simulink model "untitled"  (R2016a)
settings: Solver=VariableStepAuto  StartTime=0.0  StopTime=10.0  RelTol=1e-3
libraries: neural x419
(part 4 of 5)

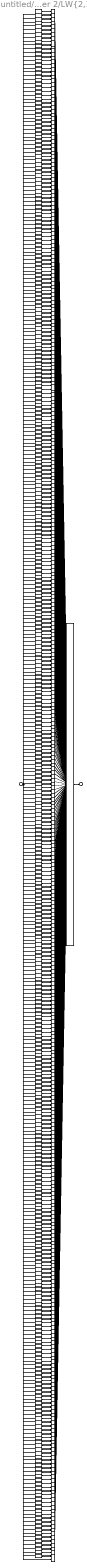
== system untitled/Function Fitting Neural Network/Layer 2/LW{2,1} ==
  "ad{2,1}" : Inport  PortDimensions=10
      mask Display: e = 0.06;c1 = [120 230 180]/255;c2 = ([120 230 180]+0)/(256+128);c3 = ([120 230 180]+128)/(256+128);patch([0 1 1 0],[0 0 1 1],c1);patch([0 1 1 1-e 1-e 0+e],[0 0 1 1-e 0+e 0+e],c2);patch([0 0 1 1-e 0+e 0+e],[0 1 1 1-e 1-e 0+e],c3);plot([0 1 1 0 0],[0 0 1 1 0]);
  "IW{2,1}(1,:)'" : Constant  Value=[0.35457568526871353;-0.37262881568746131;-0.093772998130510987;0.299001882254391;0.71652059707009119;-0.40821366360697064;-1.1727395577661341;-0.24105879281632298;-0.15545806944447227;-0.96766624006371971]
      mask Display: e = 0.06;c1 = [120 150 230]/255;c2 = ([120 150 230]+0)/383;c3 = ([120 150 230]+128)/383;patch([0 1 1 0],[0 0 1 1],c1);patch([0 1 1 1-e 1-e 0+e],[0 0 1 1-e 0+e 0+e],c2);patch([0 0 1 1-e 0+e 0+e],[0 1 1 1-e 1-e 0+e],c3);plot([0 1 1 0 0],[0 0 1 1 0]);disp('weights');
  "IW{2,1}(10,:)'" : Constant  Value=[-0.51241962484819403;0.18696428722763422;0.096689156544264743;-0.91173964698263843;1.2071503274550923;-0.1015978129931896;-1.2900331369557421;-0.89853148309609598;0.72911399796122411;0.2154652253377683]
      mask Display: e = 0.06;c1 = [120 150 230]/255;c2 = ([120 150 230]+0)/383;c3 = ([120 150 230]+128)/383;patch([0 1 1 0],[0 0 1 1],c1);patch([0 1 1 1-e 1-e 0+e],[0 0 1 1-e 0+e 0+e],c2);patch([0 0 1 1-e 0+e 0+e],[0 1 1 1-e 1-e 0+e],c3);plot([0 1 1 0 0],[0 0 1 1 0]);disp('weights');
  "IW{2,1}(100,:)'" : Constant  Value=[-0.59467351366079291;-0.46314267056547948;0.30643708606798353;0.024053983344356877;0.66007872910628429;0.75245943586493769;0.56148392880052234;0.88532483151243879;-0.50114763812176322;0.62203932838690612]
      mask Display: e = 0.06;c1 = [120 150 230]/255;c2 = ([120 150 230]+0)/383;c3 = ([120 150 230]+128)/383;patch([0 1 1 0],[0 0 1 1],c1);patch([0 1 1 1-e 1-e 0+e],[0 0 1 1-e 0+e 0+e],c2);patch([0 0 1 1-e 0+e 0+e],[0 1 1 1-e 1-e 0+e],c3);plot([0 1 1 0 0],[0 0 1 1 0]);disp('weights');
  "IW{2,1}(101,:)'" : Constant  Value=[0.132183354502735;-0.41451653539518085;0.016380979248929839;-0.74444212048968017;-0.35095430295178254;-0.45812487947094915;-0.3864796214085417;-0.1758270264418865;0.44561967553264237;-1.2062139208858689]
      mask Display: e = 0.06;c1 = [120 150 230]/255;c2 = ([120 150 230]+0)/383;c3 = ([120 150 230]+128)/383;patch([0 1 1 0],[0 0 1 1],c1);patch([0 1 1 1-e 1-e 0+e],[0 0 1 1-e 0+e 0+e],c2);patch([0 0 1 1-e 0+e 0+e],[0 1 1 1-e 1-e 0+e],c3);plot([0 1 1 0 0],[0 0 1 1 0]);disp('weights');
  "IW{2,1}(102,:)'" : Constant  Value=[0.91550733628729186;-0.17596632668060738;-0.23501466731066578;-0.43131413009170461;1.0039394563268771;-0.061370045893368474;-0.10056229228428686;0.35460263945948478;0.079910893784825646;-0.89223794061441064]
      mask Display: e = 0.06;c1 = [120 150 230]/255;c2 = ([120 150 230]+0)/383;c3 = ([120 150 230]+128)/383;patch([0 1 1 0],[0 0 1 1],c1);patch([0 1 1 1-e 1-e 0+e],[0 0 1 1-e 0+e 0+e],c2);patch([0 0 1 1-e 0+e 0+e],[0 1 1 1-e 1-e 0+e],c3);plot([0 1 1 0 0],[0 0 1 1 0]);disp('weights');
  "IW{2,1}(103,:)'" : Constant  Value=[0.012259853410431329;-0.31444307148354467;0.35552415069161591;-0.82679374849055298;-0.45038411512840826;-0.39748281945567426;-0.85214363441640906;0.44358232172792822;0.29629420030451536;0.6064841209214985]
      mask Display: e = 0.06;c1 = [120 150 230]/255;c2 = ([120 150 230]+0)/383;c3 = ([120 150 230]+128)/383;patch([0 1 1 0],[0 0 1 1],c1);patch([0 1 1 1-e 1-e 0+e],[0 0 1 1-e 0+e 0+e],c2);patch([0 0 1 1-e 0+e 0+e],[0 1 1 1-e 1-e 0+e],c3);plot([0 1 1 0 0],[0 0 1 1 0]);disp('weights');
  "IW{2,1}(104,:)'" : Constant  Value=[-0.52691192650108576;-0.19464969257009473;-0.16386531967861129;-0.31658642759094502;0.64379806911152437;0.5492776953247257;0.0085904991406464959;-0.27791306732414345;0.45618230462846576;-0.41271807660853826]
      mask Display: e = 0.06;c1 = [120 150 230]/255;c2 = ([120 150 230]+0)/383;c3 = ([120 150 230]+128)/383;patch([0 1 1 0],[0 0 1 1],c1);patch([0 1 1 1-e 1-e 0+e],[0 0 1 1-e 0+e 0+e],c2);patch([0 0 1 1-e 0+e 0+e],[0 1 1 1-e 1-e 0+e],c3);plot([0 1 1 0 0],[0 0 1 1 0]);disp('weights');
  "IW{2,1}(105,:)'" : Constant  Value=[0.0036104131310510656;-0.5108457587075188;-0.42012674601703315;-0.67458325990890222;-1.0099146022211332;0.49569765597714416;0.82567298712166171;0.10590138830719459;0.58403979278397478;0.34540661755692653]
      mask Display: e = 0.06;c1 = [120 150 230]/255;c2 = ([120 150 230]+0)/383;c3 = ([120 150 230]+128)/383;patch([0 1 1 0],[0 0 1 1],c1);patch([0 1 1 1-e 1-e 0+e],[0 0 1 1-e 0+e 0+e],c2);patch([0 0 1 1-e 0+e 0+e],[0 1 1 1-e 1-e 0+e],c3);plot([0 1 1 0 0],[0 0 1 1 0]);disp('weights');
  "IW{2,1}(106,:)'" : Constant  Value=[0.6298401480397835;-0.35713898884332712;1.0969036725783468;0.22290348339327648;0.63928028679609472;0.19280713089077245;0.57375743745156227;0.35484963283244514;0.54621996310164911;-0.42525917136785357]
      mask Display: e = 0.06;c1 = [120 150 230]/255;c2 = ([120 150 230]+0)/383;c3 = ([120 150 230]+128)/383;patch([0 1 1 0],[0 0 1 1],c1);patch([0 1 1 1-e 1-e 0+e],[0 0 1 1-e 0+e 0+e],c2);patch([0 0 1 1-e 0+e 0+e],[0 1 1 1-e 1-e 0+e],c3);plot([0 1 1 0 0],[0 0 1 1 0]);disp('weights');
  "IW{2,1}(107,:)'" : Constant  Value=[-0.54121767469762583;-0.15709203256179666;0.56849802045345743;-0.63744679364538026;-0.83237528600719402;0.30709467382596495;-0.54279673919964622;0.054529333255173174;0.20487910196507619;0.93234667245376635]
      mask Display: e = 0.06;c1 = [120 150 230]/255;c2 = ([120 150 230]+0)/383;c3 = ([120 150 230]+128)/383;patch([0 1 1 0],[0 0 1 1],c1);patch([0 1 1 1-e 1-e 0+e],[0 0 1 1-e 0+e 0+e],c2);patch([0 0 1 1-e 0+e 0+e],[0 1 1 1-e 1-e 0+e],c3);plot([0 1 1 0 0],[0 0 1 1 0]);disp('weights');
  "IW{2,1}(108,:)'" : Constant  Value=[0.87117914257995643;-0.8350687060946369;-0.52769471700262027;0.095004289510615431;1.1883750573422214;-0.049426168392697201;0.77796622090666123;0.47514241846633865;0.70746717159394057;0.46821260443696688]
      mask Display: e = 0.06;c1 = [120 150 230]/255;c2 = ([120 150 230]+0)/383;c3 = ([120 150 230]+128)/383;patch([0 1 1 0],[0 0 1 1],c1);patch([0 1 1 1-e 1-e 0+e],[0 0 1 1-e 0+e 0+e],c2);patch([0 0 1 1-e 0+e 0+e],[0 1 1 1-e 1-e 0+e],c3);plot([0 1 1 0 0],[0 0 1 1 0]);disp('weights');
  "IW{2,1}(109,:)'" : Constant  Value=[-0.093098287400667917;-0.42566624607377573;0.13802357294765616;0.12600752979896604;-0.39805809535751313;0.051077209656586242;-0.010384967949629564;-0.098925686133072455;0.95828758938569147;0.63472242371386045]
      mask Display: e = 0.06;c1 = [120 150 230]/255;c2 = ([120 150 230]+0)/383;c3 = ([120 150 230]+128)/383;patch([0 1 1 0],[0 0 1 1],c1);patch([0 1 1 1-e 1-e 0+e],[0 0 1 1-e 0+e 0+e],c2);patch([0 0 1 1-e 0+e 0+e],[0 1 1 1-e 1-e 0+e],c3);plot([0 1 1 0 0],[0 0 1 1 0]);disp('weights');
  "IW{2,1}(11,:)'" : Constant  Value=[0.87385905042111978;-0.59302251482942259;-0.57235715014876254;0.68353185522794968;1.0174079732112598;0.27032333860384478;-0.055552601487100089;-0.60055456873861501;0.69962443470780555;-0.87073796700187378]
      mask Display: e = 0.06;c1 = [120 150 230]/255;c2 = ([120 150 230]+0)/383;c3 = ([120 150 230]+128)/383;patch([0 1 1 0],[0 0 1 1],c1);patch([0 1 1 1-e 1-e 0+e],[0 0 1 1-e 0+e 0+e],c2);patch([0 0 1 1-e 0+e 0+e],[0 1 1 1-e 1-e 0+e],c3);plot([0 1 1 0 0],[0 0 1 1 0]);disp('weights');
  "IW{2,1}(110,:)'" : Constant  Value=[-0.45402764551089492;-0.4424626913130032;0.70634245673847851;0.12095992557048846;-0.76716468124193804;0.64679971773739886;0.73068307254207221;-0.1155523840382818;0.75520677335095443;-5.4313536676370289e-06]
      mask Display: e = 0.06;c1 = [120 150 230]/255;c2 = ([120 150 230]+0)/383;c3 = ([120 150 230]+128)/383;patch([0 1 1 0],[0 0 1 1],c1);patch([0 1 1 1-e 1-e 0+e],[0 0 1 1-e 0+e 0+e],c2);patch([0 0 1 1-e 0+e 0+e],[0 1 1 1-e 1-e 0+e],c3);plot([0 1 1 0 0],[0 0 1 1 0]);disp('weights');
  "IW{2,1}(111,:)'" : Constant  Value=[0.35856321400782343;-0.12534766693171134;0.07962987090539092;-0.60785703622425813;-0.38430086232607419;0.30093885714405233;-0.29137973701213238;0.24631778243741809;-0.5626882874146204;-0.6833696969081674]
      mask Display: e = 0.06;c1 = [120 150 230]/255;c2 = ([120 150 230]+0)/383;c3 = ([120 150 230]+128)/383;patch([0 1 1 0],[0 0 1 1],c1);patch([0 1 1 1-e 1-e 0+e],[0 0 1 1-e 0+e 0+e],c2);patch([0 0 1 1-e 0+e 0+e],[0 1 1 1-e 1-e 0+e],c3);plot([0 1 1 0 0],[0 0 1 1 0]);disp('weights');
  "IW{2,1}(112,:)'" : Constant  Value=[-0.51368243852562334;-0.48320720571860942;0.15046834876398124;-0.15687559453180761;0.4695672881405818;0.40398577095198729;-0.8294845938603097;0.45460692171736328;-0.65214613716902159;0.5645422206690478]
      mask Display: e = 0.06;c1 = [120 150 230]/255;c2 = ([120 150 230]+0)/383;c3 = ([120 150 230]+128)/383;patch([0 1 1 0],[0 0 1 1],c1);patch([0 1 1 1-e 1-e 0+e],[0 0 1 1-e 0+e 0+e],c2);patch([0 0 1 1-e 0+e 0+e],[0 1 1 1-e 1-e 0+e],c3);plot([0 1 1 0 0],[0 0 1 1 0]);disp('weights');
  "IW{2,1}(113,:)'" : Constant  Value=[0.2249827070654358;-0.5547870151241886;0.44125214045465366;0.10185870942545092;-0.72373304904497293;0.36734856354623896;-0.3943082956206293;-0.013381755084662945;-0.61597198634890338;0.073567333518367112]
      mask Display: e = 0.06;c1 = [120 150 230]/255;c2 = ([120 150 230]+0)/383;c3 = ([120 150 230]+128)/383;patch([0 1 1 0],[0 0 1 1],c1);patch([0 1 1 1-e 1-e 0+e],[0 0 1 1-e 0+e 0+e],c2);patch([0 0 1 1-e 0+e 0+e],[0 1 1 1-e 1-e 0+e],c3);plot([0 1 1 0 0],[0 0 1 1 0]);disp('weights');
  "IW{2,1}(114,:)'" : Constant  Value=[0.44715657086469585;-0.72184644042513646;-0.10679542344572371;0.33394805863425275;1.3097117535626552;0.13752345875085706;0.0041012097003376366;0.52921934544137084;0.47705001987924522;0.60162273497358432]
      mask Display: e = 0.06;c1 = [120 150 230]/255;c2 = ([120 150 230]+0)/383;c3 = ([120 150 230]+128)/383;patch([0 1 1 0],[0 0 1 1],c1);patch([0 1 1 1-e 1-e 0+e],[0 0 1 1-e 0+e 0+e],c2);patch([0 0 1 1-e 0+e 0+e],[0 1 1 1-e 1-e 0+e],c3);plot([0 1 1 0 0],[0 0 1 1 0]);disp('weights');
  "IW{2,1}(115,:)'" : Constant  Value=[0.072990874063348754;0.3863994496468931;-0.99669381823398551;-0.82947335628810992;-0.926316182620321;0.12138423091903472;-0.42001636335877995;-0.52417760541218628;0.11809912221407559;0.74754410579861164]
      mask Display: e = 0.06;c1 = [120 150 230]/255;c2 = ([120 150 230]+0)/383;c3 = ([120 150 230]+128)/383;patch([0 1 1 0],[0 0 1 1],c1);patch([0 1 1 1-e 1-e 0+e],[0 0 1 1-e 0+e 0+e],c2);patch([0 0 1 1-e 0+e 0+e],[0 1 1 1-e 1-e 0+e],c3);plot([0 1 1 0 0],[0 0 1 1 0]);disp('weights');
  "IW{2,1}(116,:)'" : Constant  Value=[-0.2288055411522181;0.14131988055967634;0.52041469449043676;-0.99856714860427098;0.17410368995406242;-0.052745805695831871;-0.99979512395444892;-0.35899147958971089;0.020783894468624331;-0.074273715439050342]
      mask Display: e = 0.06;c1 = [120 150 230]/255;c2 = ([120 150 230]+0)/383;c3 = ([120 150 230]+128)/383;patch([0 1 1 0],[0 0 1 1],c1);patch([0 1 1 1-e 1-e 0+e],[0 0 1 1-e 0+e 0+e],c2);patch([0 0 1 1-e 0+e 0+e],[0 1 1 1-e 1-e 0+e],c3);plot([0 1 1 0 0],[0 0 1 1 0]);disp('weights');
  "IW{2,1}(117,:)'" : Constant  Value=[-0.82340701668346539;-0.51434424071955409;0.91471776355589407;-0.33288238922418745;0.25648880682466646;0.70822982577740778;-0.6932001556180224;0.31607280530056825;-0.93009913518226872;0.068609139618715453]
      mask Display: e = 0.06;c1 = [120 150 230]/255;c2 = ([120 150 230]+0)/383;c3 = ([120 150 230]+128)/383;patch([0 1 1 0],[0 0 1 1],c1);patch([0 1 1 1-e 1-e 0+e],[0 0 1 1-e 0+e 0+e],c2);patch([0 0 1 1-e 0+e 0+e],[0 1 1 1-e 1-e 0+e],c3);plot([0 1 1 0 0],[0 0 1 1 0]);disp('weights');
  "IW{2,1}(118,:)'" : Constant  Value=[-0.49649736447447651;0.45372633367474352;-0.34080312653242439;-0.66503308065530253;-0.1437992940186234;0.40249309287773155;-0.99295207713203126;-0.33562443638377937;-0.56546214554735619;0.49432810354427731]
      mask Display: e = 0.06;c1 = [120 150 230]/255;c2 = ([120 150 230]+0)/383;c3 = ([120 150 230]+128)/383;patch([0 1 1 0],[0 0 1 1],c1);patch([0 1 1 1-e 1-e 0+e],[0 0 1 1-e 0+e 0+e],c2);patch([0 0 1 1-e 0+e 0+e],[0 1 1 1-e 1-e 0+e],c3);plot([0 1 1 0 0],[0 0 1 1 0]);disp('weights');
  "IW{2,1}(119,:)'" : Constant  Value=[-0.10669085982625769;-0.21956149733535044;0.58793916789199496;-0.40100123749963718;-0.91327196109126496;0.53224945141593838;0.47283979571705442;-0.4790545028876399;1.1407185294966518;0.0053917100134790452]
      mask Display: e = 0.06;c1 = [120 150 230]/255;c2 = ([120 150 230]+0)/383;c3 = ([120 150 230]+128)/383;patch([0 1 1 0],[0 0 1 1],c1);patch([0 1 1 1-e 1-e 0+e],[0 0 1 1-e 0+e 0+e],c2);patch([0 0 1 1-e 0+e 0+e],[0 1 1 1-e 1-e 0+e],c3);plot([0 1 1 0 0],[0 0 1 1 0]);disp('weights');
  "IW{2,1}(12,:)'" : Constant  Value=[0.48160846672355573;0.19812719218488389;-0.44365884094007213;-0.1118865542679382;0.27293932443032587;-0.22992509263083483;-1.2232905553509303;-0.49844923236274263;0.45638164301901762;0.12236853164908057]
      mask Display: e = 0.06;c1 = [120 150 230]/255;c2 = ([120 150 230]+0)/383;c3 = ([120 150 230]+128)/383;patch([0 1 1 0],[0 0 1 1],c1);patch([0 1 1 1-e 1-e 0+e],[0 0 1 1-e 0+e 0+e],c2);patch([0 0 1 1-e 0+e 0+e],[0 1 1 1-e 1-e 0+e],c3);plot([0 1 1 0 0],[0 0 1 1 0]);disp('weights');
  "IW{2,1}(120,:)'" : Constant  Value=[-0.10634859977705739;-0.052631616825708348;1.4195649331520863;-0.00084437965909707957;0.42285466275429279;0.70700655299443582;0.34595288214413045;0.14152229005737385;-0.062790561497810926;-0.50122881361225213]
      mask Display: e = 0.06;c1 = [120 150 230]/255;c2 = ([120 150 230]+0)/383;c3 = ([120 150 230]+128)/383;patch([0 1 1 0],[0 0 1 1],c1);patch([0 1 1 1-e 1-e 0+e],[0 0 1 1-e 0+e 0+e],c2);patch([0 0 1 1-e 0+e 0+e],[0 1 1 1-e 1-e 0+e],c3);plot([0 1 1 0 0],[0 0 1 1 0]);disp('weights');
  "IW{2,1}(121,:)'" : Constant  Value=[0.75241460306983421;-0.12382045592416158;-0.18934015310768379;0.15978093552599948;-0.40957040115013393;0.55440558737447043;0.31139781430429297;0.35891166148113807;0.84576008771658606;-0.92215142010749429]
      mask Display: e = 0.06;c1 = [120 150 230]/255;c2 = ([120 150 230]+0)/383;c3 = ([120 150 230]+128)/383;patch([0 1 1 0],[0 0 1 1],c1);patch([0 1 1 1-e 1-e 0+e],[0 0 1 1-e 0+e 0+e],c2);patch([0 0 1 1-e 0+e 0+e],[0 1 1 1-e 1-e 0+e],c3);plot([0 1 1 0 0],[0 0 1 1 0]);disp('weights');
  "IW{2,1}(122,:)'" : Constant  Value=[0.014533892077952471;-1.0864692283910478;-0.24978734334647062;-0.20714287190409467;0.41688992619603121;0.020843004186868241;-0.30036513169667467;0.6447122172862042;-0.44816953174537666;-0.6254452491744753]
      mask Display: e = 0.06;c1 = [120 150 230]/255;c2 = ([120 150 230]+0)/383;c3 = ([120 150 230]+128)/383;patch([0 1 1 0],[0 0 1 1],c1);patch([0 1 1 1-e 1-e 0+e],[0 0 1 1-e 0+e 0+e],c2);patch([0 0 1 1-e 0+e 0+e],[0 1 1 1-e 1-e 0+e],c3);plot([0 1 1 0 0],[0 0 1 1 0]);disp('weights');
  "IW{2,1}(123,:)'" : Constant  Value=[-0.55358584751208206;-0.92521608564350843;0.67501683373877341;-0.070487248336855296;0.020102317195281716;-0.31375904864237314;-1.0252812554265067;-0.29798368298503497;-0.22574251461160327;-0.057919377180048304]
      mask Display: e = 0.06;c1 = [120 150 230]/255;c2 = ([120 150 230]+0)/383;c3 = ([120 150 230]+128)/383;patch([0 1 1 0],[0 0 1 1],c1);patch([0 1 1 1-e 1-e 0+e],[0 0 1 1-e 0+e 0+e],c2);patch([0 0 1 1-e 0+e 0+e],[0 1 1 1-e 1-e 0+e],c3);plot([0 1 1 0 0],[0 0 1 1 0]);disp('weights');
  "IW{2,1}(124,:)'" : Constant  Value=[-0.094164787441411352;-0.90477229098315259;-0.14308614220465629;0.68442827404295736;0.95717575287916334;-0.18018870819129618;-1.0367015099687653;-0.228224166373137;0.44195239019836341;0.29375654463105255]
      mask Display: e = 0.06;c1 = [120 150 230]/255;c2 = ([120 150 230]+0)/383;c3 = ([120 150 230]+128)/383;patch([0 1 1 0],[0 0 1 1],c1);patch([0 1 1 1-e 1-e 0+e],[0 0 1 1-e 0+e 0+e],c2);patch([0 0 1 1-e 0+e 0+e],[0 1 1 1-e 1-e 0+e],c3);plot([0 1 1 0 0],[0 0 1 1 0]);disp('weights');
  "IW{2,1}(125,:)'" : Constant  Value=[0.25918346779046053;-0.66229732874088987;-0.14821536867020529;0.37319280184569709;0.77589616900903002;0.66975340214018286;0.86153956282309252;0.34949141088372687;-0.71824829000813462;0.8783877605606627]
      mask Display: e = 0.06;c1 = [120 150 230]/255;c2 = ([120 150 230]+0)/383;c3 = ([120 150 230]+128)/383;patch([0 1 1 0],[0 0 1 1],c1);patch([0 1 1 1-e 1-e 0+e],[0 0 1 1-e 0+e 0+e],c2);patch([0 0 1 1-e 0+e 0+e],[0 1 1 1-e 1-e 0+e],c3);plot([0 1 1 0 0],[0 0 1 1 0]);disp('weights');
  "IW{2,1}(126,:)'" : Constant  Value=[-0.085774924571177247;-1.2775593839237314;-1.0753491198620599;-0.1245259294998598;0.88107812747589931;-0.42695412098538321;-0.58480038198142781;0.82133593724887144;-0.75444202274592564;0.17411838762112253]
      mask Display: e = 0.06;c1 = [120 150 230]/255;c2 = ([120 150 230]+0)/383;c3 = ([120 150 230]+128)/383;patch([0 1 1 0],[0 0 1 1],c1);patch([0 1 1 1-e 1-e 0+e],[0 0 1 1-e 0+e 0+e],c2);patch([0 0 1 1-e 0+e 0+e],[0 1 1 1-e 1-e 0+e],c3);plot([0 1 1 0 0],[0 0 1 1 0]);disp('weights');
  "IW{2,1}(127,:)'" : Constant  Value=[0.19769923896271896;-0.89301981169820355;-0.11564107353940761;-0.25978116749604885;0.56145028987742485;0.42377493028536328;1.2224631895737739;0.57960114490207171;0.37954472845902248;0.11026282514903726]
      mask Display: e = 0.06;c1 = [120 150 230]/255;c2 = ([120 150 230]+0)/383;c3 = ([120 150 230]+128)/383;patch([0 1 1 0],[0 0 1 1],c1);patch([0 1 1 1-e 1-e 0+e],[0 0 1 1-e 0+e 0+e],c2);patch([0 0 1 1-e 0+e 0+e],[0 1 1 1-e 1-e 0+e],c3);plot([0 1 1 0 0],[0 0 1 1 0]);disp('weights');
  "IW{2,1}(128,:)'" : Constant  Value=[0.52884557596552373;-0.25984156317850038;-0.12794366690907111;0.01803659075444497;-0.27347206670087748;0.342733749696636;-0.51354095947049949;0.16186322264992775;-1.0862616684542652;1.4767430332722691]
      mask Display: e = 0.06;c1 = [120 150 230]/255;c2 = ([120 150 230]+0)/383;c3 = ([120 150 230]+128)/383;patch([0 1 1 0],[0 0 1 1],c1);patch([0 1 1 1-e 1-e 0+e],[0 0 1 1-e 0+e 0+e],c2);patch([0 0 1 1-e 0+e 0+e],[0 1 1 1-e 1-e 0+e],c3);plot([0 1 1 0 0],[0 0 1 1 0]);disp('weights');
  "IW{2,1}(129,:)'" : Constant  Value=[0.75786961871891667;-0.074835868624982871;0.79040911501239242;1.0007053012623659;0.37791249894770557;0.85316218872741612;0.40970699716135928;0.88783479708554969;-0.87875083537845844;0.59899649409211353]
      mask Display: e = 0.06;c1 = [120 150 230]/255;c2 = ([120 150 230]+0)/383;c3 = ([120 150 230]+128)/383;patch([0 1 1 0],[0 0 1 1],c1);patch([0 1 1 1-e 1-e 0+e],[0 0 1 1-e 0+e 0+e],c2);patch([0 0 1 1-e 0+e 0+e],[0 1 1 1-e 1-e 0+e],c3);plot([0 1 1 0 0],[0 0 1 1 0]);disp('weights');
  "IW{2,1}(13,:)'" : Constant  Value=[0.68737360350036181;0.14343559982558957;0.35348444111783106;0.60648354004990934;0.91124708494743012;0.04306279224824705;-0.18153377551600688;0.68901300485973116;-0.50222409270449153;0.13877128185435972]
      mask Display: e = 0.06;c1 = [120 150 230]/255;c2 = ([120 150 230]+0)/383;c3 = ([120 150 230]+128)/383;patch([0 1 1 0],[0 0 1 1],c1);patch([0 1 1 1-e 1-e 0+e],[0 0 1 1-e 0+e 0+e],c2);patch([0 0 1 1-e 0+e 0+e],[0 1 1 1-e 1-e 0+e],c3);plot([0 1 1 0 0],[0 0 1 1 0]);disp('weights');
  "IW{2,1}(130,:)'" : Constant  Value=[0.54323359350819234;-0.25298207203940526;0.39779238695437691;0.28493583185010518;-0.72980298213089956;0.0007700830524480784;-0.45352416582028754;0.077090561776502087;-0.19742973340063341;-0.29070953650683073]
      mask Display: e = 0.06;c1 = [120 150 230]/255;c2 = ([120 150 230]+0)/383;c3 = ([120 150 230]+128)/383;patch([0 1 1 0],[0 0 1 1],c1);patch([0 1 1 1-e 1-e 0+e],[0 0 1 1-e 0+e 0+e],c2);patch([0 0 1 1-e 0+e 0+e],[0 1 1 1-e 1-e 0+e],c3);plot([0 1 1 0 0],[0 0 1 1 0]);disp('weights');
  "IW{2,1}(131,:)'" : Constant  Value=[0.97878280264957052;-0.49403704756137012;-0.36677975235608196;0.097786011441210408;-0.018498962251421613;-0.36530395873255661;0.2334949438478936;-0.22826989708304976;0.15268980758730025;0.14933168696978888]
      mask Display: e = 0.06;c1 = [120 150 230]/255;c2 = ([120 150 230]+0)/383;c3 = ([120 150 230]+128)/383;patch([0 1 1 0],[0 0 1 1],c1);patch([0 1 1 1-e 1-e 0+e],[0 0 1 1-e 0+e 0+e],c2);patch([0 0 1 1-e 0+e 0+e],[0 1 1 1-e 1-e 0+e],c3);plot([0 1 1 0 0],[0 0 1 1 0]);disp('weights');
  "IW{2,1}(132,:)'" : Constant  Value=[0.60411093516280645;0.81353606944854429;0.003599919896469711;-0.9407960401058918;0.13795065004212817;0.41634349891179523;0.61553232960671089;0.18584762270653454;0.75915028452746958;-0.72757720678792848]
      mask Display: e = 0.06;c1 = [120 150 230]/255;c2 = ([120 150 230]+0)/383;c3 = ([120 150 230]+128)/383;patch([0 1 1 0],[0 0 1 1],c1);patch([0 1 1 1-e 1-e 0+e],[0 0 1 1-e 0+e 0+e],c2);patch([0 0 1 1-e 0+e 0+e],[0 1 1 1-e 1-e 0+e],c3);plot([0 1 1 0 0],[0 0 1 1 0]);disp('weights');
  "IW{2,1}(133,:)'" : Constant  Value=[0.89636858614286585;-0.43930648748674328;0.36348095586936136;0.42202233354664997;0.080242274820562204;-0.17527706896099893;-0.27678234817463548;0.18205392307498788;0.26248544652801364;-0.60731321474183864]
      mask Display: e = 0.06;c1 = [120 150 230]/255;c2 = ([120 150 230]+0)/383;c3 = ([120 150 230]+128)/383;patch([0 1 1 0],[0 0 1 1],c1);patch([0 1 1 1-e 1-e 0+e],[0 0 1 1-e 0+e 0+e],c2);patch([0 0 1 1-e 0+e 0+e],[0 1 1 1-e 1-e 0+e],c3);plot([0 1 1 0 0],[0 0 1 1 0]);disp('weights');
  "IW{2,1}(134,:)'" : Constant  Value=[0.46766779301282968;-0.66166835902964338;-0.053471630666557482;0.20941091529739264;-0.27431112396490887;-0.038380363421930963;0.57150995549276795;-0.11805819126615381;0.4542250235667678;0.55470191658962753]
      mask Display: e = 0.06;c1 = [120 150 230]/255;c2 = ([120 150 230]+0)/383;c3 = ([120 150 230]+128)/383;patch([0 1 1 0],[0 0 1 1],c1);patch([0 1 1 1-e 1-e 0+e],[0 0 1 1-e 0+e 0+e],c2);patch([0 0 1 1-e 0+e 0+e],[0 1 1 1-e 1-e 0+e],c3);plot([0 1 1 0 0],[0 0 1 1 0]);disp('weights');
  "IW{2,1}(135,:)'" : Constant  Value=[0.43487119300343791;-0.12294690238958098;-0.087736019523446507;0.26167006899088735;-0.5885537372425822;0.57930981669587878;-0.33638400569811111;0.3704508366766428;-0.3399032648473701;-0.28242557070351021]
      mask Display: e = 0.06;c1 = [120 150 230]/255;c2 = ([120 150 230]+0)/383;c3 = ([120 150 230]+128)/383;patch([0 1 1 0],[0 0 1 1],c1);patch([0 1 1 1-e 1-e 0+e],[0 0 1 1-e 0+e 0+e],c2);patch([0 0 1 1-e 0+e 0+e],[0 1 1 1-e 1-e 0+e],c3);plot([0 1 1 0 0],[0 0 1 1 0]);disp('weights');
  "IW{2,1}(136,:)'" : Constant  Value=[0.87531369177677609;-0.088562053715001116;-0.50157240895004473;-0.47102435346078919;0.69915570499538215;-0.27921213245334076;-0.87326892756430141;0.36052387179430673;-0.96143693001145092;-0.17549088416610464]
      mask Display: e = 0.06;c1 = [120 150 230]/255;c2 = ([120 150 230]+0)/383;c3 = ([120 150 230]+128)/383;patch([0 1 1 0],[0 0 1 1],c1);patch([0 1 1 1-e 1-e 0+e],[0 0 1 1-e 0+e 0+e],c2);patch([0 0 1 1-e 0+e 0+e],[0 1 1 1-e 1-e 0+e],c3);plot([0 1 1 0 0],[0 0 1 1 0]);disp('weights');
  "IW{2,1}(137,:)'" : Constant  Value=[0.04084567294535886;-0.45479850199360849;-0.15935677807927359;-0.16347981152794955;0.83695772071454166;0.69898633357112272;0.92626956822206041;0.31086917495667193;-0.18959112727733612;0.7499543456261748]
      mask Display: e = 0.06;c1 = [120 150 230]/255;c2 = ([120 150 230]+0)/383;c3 = ([120 150 230]+128)/383;patch([0 1 1 0],[0 0 1 1],c1);patch([0 1 1 1-e 1-e 0+e],[0 0 1 1-e 0+e 0+e],c2);patch([0 0 1 1-e 0+e 0+e],[0 1 1 1-e 1-e 0+e],c3);plot([0 1 1 0 0],[0 0 1 1 0]);disp('weights');
  "IW{2,1}(138,:)'" : Constant  Value=[0.57219232295499267;0.020263776079628176;-0.079704395170736755;-0.74272920860931724;0.82984320022030256;0.24958130088689573;0.77599202689430868;0.31725933454895744;0.42162457988928725;-0.24703646084574413]
      mask Display: e = 0.06;c1 = [120 150 230]/255;c2 = ([120 150 230]+0)/383;c3 = ([120 150 230]+128)/383;patch([0 1 1 0],[0 0 1 1],c1);patch([0 1 1 1-e 1-e 0+e],[0 0 1 1-e 0+e 0+e],c2);patch([0 0 1 1-e 0+e 0+e],[0 1 1 1-e 1-e 0+e],c3);plot([0 1 1 0 0],[0 0 1 1 0]);disp('weights');
  "IW{2,1}(139,:)'" : Constant  Value=[-0.64791329129744479;-0.68039534992550543;0.46068321870552537;-0.44670816247921685;-0.85457524198659396;0.052372287861784883;-0.28315196682942978;0.050960586513293604;-0.34113385269778135;-0.12619683269990617]
      mask Display: e = 0.06;c1 = [120 150 230]/255;c2 = ([120 150 230]+0)/383;c3 = ([120 150 230]+128)/383;patch([0 1 1 0],[0 0 1 1],c1);patch([0 1 1 1-e 1-e 0+e],[0 0 1 1-e 0+e 0+e],c2);patch([0 0 1 1-e 0+e 0+e],[0 1 1 1-e 1-e 0+e],c3);plot([0 1 1 0 0],[0 0 1 1 0]);disp('weights');
  "IW{2,1}(14,:)'" : Constant  Value=[0.60307547539237827;0.26160630807644503;-0.31915455123711362;0.35648864783644302;0.10935038552164415;0.57115159516591585;0.13337076223726663;-0.33810699894513374;-0.0076439180204547971;-0.34620005775426466]
      mask Display: e = 0.06;c1 = [120 150 230]/255;c2 = ([120 150 230]+0)/383;c3 = ([120 150 230]+128)/383;patch([0 1 1 0],[0 0 1 1],c1);patch([0 1 1 1-e 1-e 0+e],[0 0 1 1-e 0+e 0+e],c2);patch([0 0 1 1-e 0+e 0+e],[0 1 1 1-e 1-e 0+e],c3);plot([0 1 1 0 0],[0 0 1 1 0]);disp('weights');
  "IW{2,1}(140,:)'" : Constant  Value=[-0.0030291752852869558;-0.67980394133413324;-0.17885139181676857;-0.76669362139205643;0.22816259255475249;-0.47415457060627852;-1.1503135723297553;-0.61111712626978165;-0.12145632927079997;-0.85689992494030265]
      mask Display: e = 0.06;c1 = [120 150 230]/255;c2 = ([120 150 230]+0)/383;c3 = ([120 150 230]+128)/383;patch([0 1 1 0],[0 0 1 1],c1);patch([0 1 1 1-e 1-e 0+e],[0 0 1 1-e 0+e 0+e],c2);patch([0 0 1 1-e 0+e 0+e],[0 1 1 1-e 1-e 0+e],c3);plot([0 1 1 0 0],[0 0 1 1 0]);disp('weights');
  "IW{2,1}(141,:)'" : Constant  Value=[1.1528381514813444;-0.19886352123262094;-0.32237521779107103;0.53280504643341076;0.54235638409397091;-0.20431979798160893;0.41859342160632868;-0.27049055688648832;0.72348698962931113;0.22721198189363229]
      mask Display: e = 0.06;c1 = [120 150 230]/255;c2 = ([120 150 230]+0)/383;c3 = ([120 150 230]+128)/383;patch([0 1 1 0],[0 0 1 1],c1);patch([0 1 1 1-e 1-e 0+e],[0 0 1 1-e 0+e 0+e],c2);patch([0 0 1 1-e 0+e 0+e],[0 1 1 1-e 1-e 0+e],c3);plot([0 1 1 0 0],[0 0 1 1 0]);disp('weights');
  "IW{2,1}(142,:)'" : Constant  Value=[1.0348774094391338;0.39994075004194773;-0.10449199246842319;0.58555814890475077;-0.43854398931414074;0.62129764197704607;0.57989198576789014;0.61806327947082651;-0.80509314522689135;0.22740352648194026]
      mask Display: e = 0.06;c1 = [120 150 230]/255;c2 = ([120 150 230]+0)/383;c3 = ([120 150 230]+128)/383;patch([0 1 1 0],[0 0 1 1],c1);patch([0 1 1 1-e 1-e 0+e],[0 0 1 1-e 0+e 0+e],c2);patch([0 0 1 1-e 0+e 0+e],[0 1 1 1-e 1-e 0+e],c3);plot([0 1 1 0 0],[0 0 1 1 0]);disp('weights');
  "IW{2,1}(143,:)'" : Constant  Value=[0.47591930778768854;0.11029936675550972;-0.11704275436264812;-1.1282355903680503;0.035452001204951289;-0.35020455737237144;-0.41406855655358321;-0.057474545214064456;-0.24301739685938317;-0.75257830822867067]
      mask Display: e = 0.06;c1 = [120 150 230]/255;c2 = ([120 150 230]+0)/383;c3 = ([120 150 230]+128)/383;patch([0 1 1 0],[0 0 1 1],c1);patch([0 1 1 1-e 1-e 0+e],[0 0 1 1-e 0+e 0+e],c2);patch([0 0 1 1-e 0+e 0+e],[0 1 1 1-e 1-e 0+e],c3);plot([0 1 1 0 0],[0 0 1 1 0]);disp('weights');
  "IW{2,1}(144,:)'" : Constant  Value=[0.013610878879226157;-0.5936025788659649;0.17473336943233647;0.11562238591574327;0.65243191169465042;0.69623129247364601;0.033335398108974762;0.26830968898347057;-0.18982946576075041;-0.3178018271525288]
      mask Display: e = 0.06;c1 = [120 150 230]/255;c2 = ([120 150 230]+0)/383;c3 = ([120 150 230]+128)/383;patch([0 1 1 0],[0 0 1 1],c1);patch([0 1 1 1-e 1-e 0+e],[0 0 1 1-e 0+e 0+e],c2);patch([0 0 1 1-e 0+e 0+e],[0 1 1 1-e 1-e 0+e],c3);plot([0 1 1 0 0],[0 0 1 1 0]);disp('weights');
  "IW{2,1}(145,:)'" : Constant  Value=[0.79353310108425479;-0.98041238760606764;0.43142067668329331;0.94935906057659536;-0.25235217004692806;-0.11597467566125697;-0.79824077009467964;0.58212520912044108;-0.62611583634461465;-0.26615231117298133]
      mask Display: e = 0.06;c1 = [120 150 230]/255;c2 = ([120 150 230]+0)/383;c3 = ([120 150 230]+128)/383;patch([0 1 1 0],[0 0 1 1],c1);patch([0 1 1 1-e 1-e 0+e],[0 0 1 1-e 0+e 0+e],c2);patch([0 0 1 1-e 0+e 0+e],[0 1 1 1-e 1-e 0+e],c3);plot([0 1 1 0 0],[0 0 1 1 0]);disp('weights');
  "IW{2,1}(146,:)'" : Constant  Value=[-0.14663084735383669;-0.7152012856519111;0.79022637736240497;-0.39265024231146162;0.11015162851622627;0.1439881491271458;-0.21722187234832716;0.35490782758032535;-0.28781516352467973;-0.83905117783707472]
      mask Display: e = 0.06;c1 = [120 150 230]/255;c2 = ([120 150 230]+0)/383;c3 = ([120 150 230]+128)/383;patch([0 1 1 0],[0 0 1 1],c1);patch([0 1 1 1-e 1-e 0+e],[0 0 1 1-e 0+e 0+e],c2);patch([0 0 1 1-e 0+e 0+e],[0 1 1 1-e 1-e 0+e],c3);plot([0 1 1 0 0],[0 0 1 1 0]);disp('weights');
  "IW{2,1}(147,:)'" : Constant  Value=[0.51456095092215304;0.013308895325224501;0.23973578416266431;-0.39893358253935407;0.86217847435459549;0.23731709690746533;0.32107943016162388;0.4579415028239332;-0.12170571728965782;-0.72497605428726442]
      mask Display: e = 0.06;c1 = [120 150 230]/255;c2 = ([120 150 230]+0)/383;c3 = ([120 150 230]+128)/383;patch([0 1 1 0],[0 0 1 1],c1);patch([0 1 1 1-e 1-e 0+e],[0 0 1 1-e 0+e 0+e],c2);patch([0 0 1 1-e 0+e 0+e],[0 1 1 1-e 1-e 0+e],c3);plot([0 1 1 0 0],[0 0 1 1 0]);disp('weights');
  "IW{2,1}(148,:)'" : Constant  Value=[-0.28370341159362489;0.14189555301935247;0.22615733950226197;-1.4289170794829864;0.19275807464534023;-0.29588546279050809;-0.60250261553372697;-0.55024367335468194;0.28602429652844596;-1.2087566889439874]
      mask Display: e = 0.06;c1 = [120 150 230]/255;c2 = ([120 150 230]+0)/383;c3 = ([120 150 230]+128)/383;patch([0 1 1 0],[0 0 1 1],c1);patch([0 1 1 1-e 1-e 0+e],[0 0 1 1-e 0+e 0+e],c2);patch([0 0 1 1-e 0+e 0+e],[0 1 1 1-e 1-e 0+e],c3);plot([0 1 1 0 0],[0 0 1 1 0]);disp('weights');
  "IW{2,1}(149,:)'" : Constant  Value=[0.29220286997692346;-0.42868361288169421;0.091667071657286048;0.0023825430328358599;0.68759817291230851;0.48731248515528514;0.073982555723268464;-0.47896314396146461;0.2481890200979214;-0.78006686064629083]
      mask Display: e = 0.06;c1 = [120 150 230]/255;c2 = ([120 150 230]+0)/383;c3 = ([120 150 230]+128)/383;patch([0 1 1 0],[0 0 1 1],c1);patch([0 1 1 1-e 1-e 0+e],[0 0 1 1-e 0+e 0+e],c2);patch([0 0 1 1-e 0+e 0+e],[0 1 1 1-e 1-e 0+e],c3);plot([0 1 1 0 0],[0 0 1 1 0]);disp('weights');
  "IW{2,1}(15,:)'" : Constant  Value=[0.027354246156082423;-0.020646121194017458;0.20550677662375755;-0.27498293666632234;-0.23869423019492847;0.096752104574001796;-1.0510442688956552;-0.83070324486292213;0.79732978178235814;-0.83889015875671324]
      mask Display: e = 0.06;c1 = [120 150 230]/255;c2 = ([120 150 230]+0)/383;c3 = ([120 150 230]+128)/383;patch([0 1 1 0],[0 0 1 1],c1);patch([0 1 1 1-e 1-e 0+e],[0 0 1 1-e 0+e 0+e],c2);patch([0 0 1 1-e 0+e 0+e],[0 1 1 1-e 1-e 0+e],c3);plot([0 1 1 0 0],[0 0 1 1 0]);disp('weights');
  "IW{2,1}(150,:)'" : Constant  Value=[0.072314821230475806;-0.089772997057432122;-0.18096313889990884;-0.68836942558038616;0.61239840942242607;0.20212542154346036;0.45292734172087445;-0.010485284330795569;0.43170063614257087;0.1810436350354182]
      mask Display: e = 0.06;c1 = [120 150 230]/255;c2 = ([120 150 230]+0)/383;c3 = ([120 150 230]+128)/383;patch([0 1 1 0],[0 0 1 1],c1);patch([0 1 1 1-e 1-e 0+e],[0 0 1 1-e 0+e 0+e],c2);patch([0 0 1 1-e 0+e 0+e],[0 1 1 1-e 1-e 0+e],c3);plot([0 1 1 0 0],[0 0 1 1 0]);disp('weights');
  "IW{2,1}(151,:)'" : Constant  Value=[0.63791744792223604;-0.52440012362597233;-0.56769479278375701;0.11437610965471345;-0.80753930809768182;0.067650457274930187;-0.57024662358183942;0.34659618077985344;0.22302197923452585;0.93405287340364618]
      mask Display: e = 0.06;c1 = [120 150 230]/255;c2 = ([120 150 230]+0)/383;c3 = ([120 150 230]+128)/383;patch([0 1 1 0],[0 0 1 1],c1);patch([0 1 1 1-e 1-e 0+e],[0 0 1 1-e 0+e 0+e],c2);patch([0 0 1 1-e 0+e 0+e],[0 1 1 1-e 1-e 0+e],c3);plot([0 1 1 0 0],[0 0 1 1 0]);disp('weights');
  "IW{2,1}(152,:)'" : Constant  Value=[0.024791146885373871;-0.061381854892575499;0.28132930386047827;0.34991097193464282;1.1325090703607825;0.68024391904761816;-0.32738013100226526;0.087353940817818623;-0.39973306984110546;-0.53282532586843079]
      mask Display: e = 0.06;c1 = [120 150 230]/255;c2 = ([120 150 230]+0)/383;c3 = ([120 150 230]+128)/383;patch([0 1 1 0],[0 0 1 1],c1);patch([0 1 1 1-e 1-e 0+e],[0 0 1 1-e 0+e 0+e],c2);patch([0 0 1 1-e 0+e 0+e],[0 1 1 1-e 1-e 0+e],c3);plot([0 1 1 0 0],[0 0 1 1 0]);disp('weights');
  "IW{2,1}(153,:)'" : Constant  Value=[1.06491207737031;0.34010495276119823;-0.33332750748593798;0.28754584157773494;0.1756827854738448;0.27114649356392573;-0.63555735273315328;-0.78358807532218089;0.47929413963746681;-0.41492527236323945]
      mask Display: e = 0.06;c1 = [120 150 230]/255;c2 = ([120 150 230]+0)/383;c3 = ([120 150 230]+128)/383;patch([0 1 1 0],[0 0 1 1],c1);patch([0 1 1 1-e 1-e 0+e],[0 0 1 1-e 0+e 0+e],c2);patch([0 0 1 1-e 0+e 0+e],[0 1 1 1-e 1-e 0+e],c3);plot([0 1 1 0 0],[0 0 1 1 0]);disp('weights');
  "IW{2,1}(154,:)'" : Constant  Value=[0.8907178035764266;0.64946018103878111;0.70999227520614228;-0.30385696809634594;-0.36157016609471532;0.15420578223584994;-0.82312648802465249;0.31504114362832575;0.22849012442186289;-0.53556675269302623]
      mask Display: e = 0.06;c1 = [120 150 230]/255;c2 = ([120 150 230]+0)/383;c3 = ([120 150 230]+128)/383;patch([0 1 1 0],[0 0 1 1],c1);patch([0 1 1 1-e 1-e 0+e],[0 0 1 1-e 0+e 0+e],c2);patch([0 0 1 1-e 0+e 0+e],[0 1 1 1-e 1-e 0+e],c3);plot([0 1 1 0 0],[0 0 1 1 0]);disp('weights');
  "IW{2,1}(155,:)'" : Constant  Value=[0.56845857160035473;0.12794428308819397;-1.0559824792320389;-0.19454418478274776;-0.84777242407021192;0.32075585679187341;-0.16663460168597199;0.1717876039808795;-0.25217272172011002;0.50041646367493386]
      mask Display: e = 0.06;c1 = [120 150 230]/255;c2 = ([120 150 230]+0)/383;c3 = ([120 150 230]+128)/383;patch([0 1 1 0],[0 0 1 1],c1);patch([0 1 1 1-e 1-e 0+e],[0 0 1 1-e 0+e 0+e],c2);patch([0 0 1 1-e 0+e 0+e],[0 1 1 1-e 1-e 0+e],c3);plot([0 1 1 0 0],[0 0 1 1 0]);disp('weights');
  "IW{2,1}(156,:)'" : Constant  Value=[0.31734265948367746;-0.86274430070716202;0.7834191942023877;-0.39048802992256659;-0.63274357899852163;-0.25199370032607038;0.609149678410427;-0.0067052634023740537;1.0982604504147797;-0.44922930641990172]
      mask Display: e = 0.06;c1 = [120 150 230]/255;c2 = ([120 150 230]+0)/383;c3 = ([120 150 230]+128)/383;patch([0 1 1 0],[0 0 1 1],c1);patch([0 1 1 1-e 1-e 0+e],[0 0 1 1-e 0+e 0+e],c2);patch([0 0 1 1-e 0+e 0+e],[0 1 1 1-e 1-e 0+e],c3);plot([0 1 1 0 0],[0 0 1 1 0]);disp('weights');
  "IW{2,1}(157,:)'" : Constant  Value=[0.46809691262560055;0.14921700932002308;-0.65528379707823659;-0.55658907950372849;-0.69744891022332689;-0.60807580914863935;-1.2588155232097933;-0.54444707579354246;0.37452072641424944;-0.14818449071741602]
      mask Display: e = 0.06;c1 = [120 150 230]/255;c2 = ([120 150 230]+0)/383;c3 = ([120 150 230]+128)/383;patch([0 1 1 0],[0 0 1 1],c1);patch([0 1 1 1-e 1-e 0+e],[0 0 1 1-e 0+e 0+e],c2);patch([0 0 1 1-e 0+e 0+e],[0 1 1 1-e 1-e 0+e],c3);plot([0 1 1 0 0],[0 0 1 1 0]);disp('weights');
  "IW{2,1}(158,:)'" : Constant  Value=[0.19381412396696396;-0.4109650382526846;0.10823672208743454;-0.20929112356827995;-0.018694478198532871;0.30898456362246651;0.80357213701133889;0.87978647648148112;0.43286312443462516;-0.69647290849462973]
      mask Display: e = 0.06;c1 = [120 150 230]/255;c2 = ([120 150 230]+0)/383;c3 = ([120 150 230]+128)/383;patch([0 1 1 0],[0 0 1 1],c1);patch([0 1 1 1-e 1-e 0+e],[0 0 1 1-e 0+e 0+e],c2);patch([0 0 1 1-e 0+e 0+e],[0 1 1 1-e 1-e 0+e],c3);plot([0 1 1 0 0],[0 0 1 1 0]);disp('weights');
  "IW{2,1}(159,:)'" : Constant  Value=[-0.16816729366042349;-0.37333912502906175;-0.09840730171743628;-0.5524480626789513;0.38611411392686612;-0.21572732899710118;-0.83672091286657235;-0.560883860276987;0.66597929951592083;0.67041291507497425]
      mask Display: e = 0.06;c1 = [120 150 230]/255;c2 = ([120 150 230]+0)/383;c3 = ([120 150 230]+128)/383;patch([0 1 1 0],[0 0 1 1],c1);patch([0 1 1 1-e 1-e 0+e],[0 0 1 1-e 0+e 0+e],c2);patch([0 0 1 1-e 0+e 0+e],[0 1 1 1-e 1-e 0+e],c3);plot([0 1 1 0 0],[0 0 1 1 0]);disp('weights');
  "IW{2,1}(16,:)'" : Constant  Value=[0.54500389609400801;-0.63254888749985183;0.56314824431668098;-0.23027672723642426;-0.96518502128329753;0.12665190368120977;-0.20424130555782183;1.242002707834805;-0.37284731794168946;-0.37726013178485546]
      mask Display: e = 0.06;c1 = [120 150 230]/255;c2 = ([120 150 230]+0)/383;c3 = ([120 150 230]+128)/383;patch([0 1 1 0],[0 0 1 1],c1);patch([0 1 1 1-e 1-e 0+e],[0 0 1 1-e 0+e 0+e],c2);patch([0 0 1 1-e 0+e 0+e],[0 1 1 1-e 1-e 0+e],c3);plot([0 1 1 0 0],[0 0 1 1 0]);disp('weights');
  "IW{2,1}(160,:)'" : Constant  Value=[-0.23590294691840655;-0.85450674135541582;-0.53479330254763791;-0.36592560334689678;0.70936245493875361;0.59723231973233504;0.30367180773738833;0.31583099812655235;-0.1676910401005674;0.44565952373596124]
      mask Display: e = 0.06;c1 = [120 150 230]/255;c2 = ([120 150 230]+0)/383;c3 = ([120 150 230]+128)/383;patch([0 1 1 0],[0 0 1 1],c1);patch([0 1 1 1-e 1-e 0+e],[0 0 1 1-e 0+e 0+e],c2);patch([0 0 1 1-e 0+e 0+e],[0 1 1 1-e 1-e 0+e],c3);plot([0 1 1 0 0],[0 0 1 1 0]);disp('weights');
  "IW{2,1}(161,:)'" : Constant  Value=[-0.20980911549445522;0.0048233137333358045;-0.7404754118418424;-0.81106299834945106;0.725800071975924;-0.24916693952693403;-0.49543679646348288;-0.19807508926887657;1.1369857852347991;0.067816778055167615]
      mask Display: e = 0.06;c1 = [120 150 230]/255;c2 = ([120 150 230]+0)/383;c3 = ([120 150 230]+128)/383;patch([0 1 1 0],[0 0 1 1],c1);patch([0 1 1 1-e 1-e 0+e],[0 0 1 1-e 0+e 0+e],c2);patch([0 0 1 1-e 0+e 0+e],[0 1 1 1-e 1-e 0+e],c3);plot([0 1 1 0 0],[0 0 1 1 0]);disp('weights');
  "IW{2,1}(162,:)'" : Constant  Value=[0.15946274930453933;0.35736127554318675;-0.95546442801440756;-0.48592108616737795;0.57224277220179176;-0.20782531981751939;-0.41967417167070847;-0.29583239859493787;-0.076514831711105957;0.3931400366352773]
      mask Display: e = 0.06;c1 = [120 150 230]/255;c2 = ([120 150 230]+0)/383;c3 = ([120 150 230]+128)/383;patch([0 1 1 0],[0 0 1 1],c1);patch([0 1 1 1-e 1-e 0+e],[0 0 1 1-e 0+e 0+e],c2);patch([0 0 1 1-e 0+e 0+e],[0 1 1 1-e 1-e 0+e],c3);plot([0 1 1 0 0],[0 0 1 1 0]);disp('weights');
  "IW{2,1}(163,:)'" : Constant  Value=[-0.41818876656468723;0.24666092656643618;0.25895271607792936;-0.21241786365920245;-0.26130772575641703;0.32494949253514976;0.010562454187801495;-0.41456821743445693;0.25700421914338173;0.3203409423415875]
      mask Display: e = 0.06;c1 = [120 150 230]/255;c2 = ([120 150 230]+0)/383;c3 = ([120 150 230]+128)/383;patch([0 1 1 0],[0 0 1 1],c1);patch([0 1 1 1-e 1-e 0+e],[0 0 1 1-e 0+e 0+e],c2);patch([0 0 1 1-e 0+e 0+e],[0 1 1 1-e 1-e 0+e],c3);plot([0 1 1 0 0],[0 0 1 1 0]);disp('weights');
  "IW{2,1}(164,:)'" : Constant  Value=[0.51442066996386182;-0.003015819577765616;-0.063433191582938364;0.29527459969141168;-0.22920317431019332;-0.11623367236491922;-0.67479362637486962;-0.33250111130902082;-0.060330481809740211;-0.4274158094906596]
      mask Display: e = 0.06;c1 = [120 150 230]/255;c2 = ([120 150 230]+0)/383;c3 = ([120 150 230]+128)/383;patch([0 1 1 0],[0 0 1 1],c1);patch([0 1 1 1-e 1-e 0+e],[0 0 1 1-e 0+e 0+e],c2);patch([0 0 1 1-e 0+e 0+e],[0 1 1 1-e 1-e 0+e],c3);plot([0 1 1 0 0],[0 0 1 1 0]);disp('weights');
  "IW{2,1}(165,:)'" : Constant  Value=[0.46264296028077168;-0.47456720555458254;-0.42881117844521055;0.5184619575001751;0.16632291496523247;0.64116846063992838;-0.059537704139637659;-0.44025216263581707;-0.41095361974311811;-0.34776341799400051]
      mask Display: e = 0.06;c1 = [120 150 230]/255;c2 = ([120 150 230]+0)/383;c3 = ([120 150 230]+128)/383;patch([0 1 1 0],[0 0 1 1],c1);patch([0 1 1 1-e 1-e 0+e],[0 0 1 1-e 0+e 0+e],c2);patch([0 0 1 1-e 0+e 0+e],[0 1 1 1-e 1-e 0+e],c3);plot([0 1 1 0 0],[0 0 1 1 0]);disp('weights');
  "IW{2,1}(166,:)'" : Constant  Value=[-0.56682680391906259;-1.0546403264091522;-0.078840842338531239;-0.6012955379016125;-0.28815352659836974;-0.099630358253869566;-1.13460790898653;-0.65049525295991606;-0.29178248430398995;-0.69560962096145773]
      mask Display: e = 0.06;c1 = [120 150 230]/255;c2 = ([120 150 230]+0)/383;c3 = ([120 150 230]+128)/383;patch([0 1 1 0],[0 0 1 1],c1);patch([0 1 1 1-e 1-e 0+e],[0 0 1 1-e 0+e 0+e],c2);patch([0 0 1 1-e 0+e 0+e],[0 1 1 1-e 1-e 0+e],c3);plot([0 1 1 0 0],[0 0 1 1 0]);disp('weights');
  "IW{2,1}(167,:)'" : Constant  Value=[0.6195179573000994;-0.42436485859452522;-0.48387875371814193;0.91662737211073253;0.21389937292278516;0.087568551737672251;-1.0060614399240657;-0.75648432983775293;0.011322954345955497;-0.38600263205734392]
      mask Display: e = 0.06;c1 = [120 150 230]/255;c2 = ([120 150 230]+0)/383;c3 = ([120 150 230]+128)/383;patch([0 1 1 0],[0 0 1 1],c1);patch([0 1 1 1-e 1-e 0+e],[0 0 1 1-e 0+e 0+e],c2);patch([0 0 1 1-e 0+e 0+e],[0 1 1 1-e 1-e 0+e],c3);plot([0 1 1 0 0],[0 0 1 1 0]);disp('weights');
  "IW{2,1}(168,:)'" : Constant  Value=[0.87803930246973994;-0.64967807828078117;-0.0765156835334318;0.35915079988800569;-0.53964414359746771;-0.091909730221217956;0.28389258631612507;0.22304266887181889;-0.17025742639382721;0.27104891723090158]
      mask Display: e = 0.06;c1 = [120 150 230]/255;c2 = ([120 150 230]+0)/383;c3 = ([120 150 230]+128)/383;patch([0 1 1 0],[0 0 1 1],c1);patch([0 1 1 1-e 1-e 0+e],[0 0 1 1-e 0+e 0+e],c2);patch([0 0 1 1-e 0+e 0+e],[0 1 1 1-e 1-e 0+e],c3);plot([0 1 1 0 0],[0 0 1 1 0]);disp('weights');
  "IW{2,1}(169,:)'" : Constant  Value=[0.20939950067808555;-0.6119137149274616;0.19817931006281517;1.0219748917205338;0.096216914609944998;0.39363302227042019;0.44273382852698839;0.21655929294817444;-0.45439108193042532;0.76901779900856715]
      mask Display: e = 0.06;c1 = [120 150 230]/255;c2 = ([120 150 230]+0)/383;c3 = ([120 150 230]+128)/383;patch([0 1 1 0],[0 0 1 1],c1);patch([0 1 1 1-e 1-e 0+e],[0 0 1 1-e 0+e 0+e],c2);patch([0 0 1 1-e 0+e 0+e],[0 1 1 1-e 1-e 0+e],c3);plot([0 1 1 0 0],[0 0 1 1 0]);disp('weights');
  "IW{2,1}(17,:)'" : Constant  Value=[0.81894282446014177;-0.51446726892821204;-0.31038522558405462;0.47285478738766384;-0.020859091060327961;-0.22496815770814105;0.25938528927576238;0.059496496021567202;1.0442686890653139;0.38229940784494337]
      mask Display: e = 0.06;c1 = [120 150 230]/255;c2 = ([120 150 230]+0)/383;c3 = ([120 150 230]+128)/383;patch([0 1 1 0],[0 0 1 1],c1);patch([0 1 1 1-e 1-e 0+e],[0 0 1 1-e 0+e 0+e],c2);patch([0 0 1 1-e 0+e 0+e],[0 1 1 1-e 1-e 0+e],c3);plot([0 1 1 0 0],[0 0 1 1 0]);disp('weights');
  "IW{2,1}(170,:)'" : Constant  Value=[-0.27913100818495928;-0.2454778736151394;0.36675655699298504;0.23697130763511251;1.3133448313299465;0.54989741663652048;0.070807991668398573;0.42521625942145352;-0.65691248034242911;0.5302805390293629]
      mask Display: e = 0.06;c1 = [120 150 230]/255;c2 = ([120 150 230]+0)/383;c3 = ([120 150 230]+128)/383;patch([0 1 1 0],[0 0 1 1],c1);patch([0 1 1 1-e 1-e 0+e],[0 0 1 1-e 0+e 0+e],c2);patch([0 0 1 1-e 0+e 0+e],[0 1 1 1-e 1-e 0+e],c3);plot([0 1 1 0 0],[0 0 1 1 0]);disp('weights');
  "IW{2,1}(171,:)'" : Constant  Value=[-0.25846526751739252;-0.013142232040668833;0.10377364805326694;-0.32671987291845445;-0.23177289387293715;0.78743574151607487;0.030221850926831065;-0.81991417077719653;0.62344408919992222;0.91302104542621609]
      mask Display: e = 0.06;c1 = [120 150 230]/255;c2 = ([120 150 230]+0)/383;c3 = ([120 150 230]+128)/383;patch([0 1 1 0],[0 0 1 1],c1);patch([0 1 1 1-e 1-e 0+e],[0 0 1 1-e 0+e 0+e],c2);patch([0 0 1 1-e 0+e 0+e],[0 1 1 1-e 1-e 0+e],c3);plot([0 1 1 0 0],[0 0 1 1 0]);disp('weights');
  "IW{2,1}(172,:)'" : Constant  Value=[0.10633562063829582;-0.86237993149419501;0.75170695989268177;0.6542559027955126;-0.81783635159227608;0.32967460392178483;0.17193623657594009;0.48051005832656746;-0.65968087717478952;-0.52085021402544907]
      mask Display: e = 0.06;c1 = [120 150 230]/255;c2 = ([120 150 230]+0)/383;c3 = ([120 150 230]+128)/383;patch([0 1 1 0],[0 0 1 1],c1);patch([0 1 1 1-e 1-e 0+e],[0 0 1 1-e 0+e 0+e],c2);patch([0 0 1 1-e 0+e 0+e],[0 1 1 1-e 1-e 0+e],c3);plot([0 1 1 0 0],[0 0 1 1 0]);disp('weights');
  "IW{2,1}(173,:)'" : Constant  Value=[0.016548589156018974;-0.49419750466291595;-0.29641096164146885;0.29117837672946029;-0.44205107244597158;0.41773709504345657;-0.65903750996005239;-0.44714934294122266;0.48686398435158518;-0.10022828916760965]
      mask Display: e = 0.06;c1 = [120 150 230]/255;c2 = ([120 150 230]+0)/383;c3 = ([120 150 230]+128)/383;patch([0 1 1 0],[0 0 1 1],c1);patch([0 1 1 1-e 1-e 0+e],[0 0 1 1-e 0+e 0+e],c2);patch([0 0 1 1-e 0+e 0+e],[0 1 1 1-e 1-e 0+e],c3);plot([0 1 1 0 0],[0 0 1 1 0]);disp('weights');
  "IW{2,1}(174,:)'" : Constant  Value=[-0.88999776304472689;-0.18842923501235428;0.046850110280029833;-0.90343767112563311;0.61503488515168847;0.037403917800678643;0.094057894475024384;0.54278576673373036;0.073287024694441816;0.14100812008670038]
      mask Display: e = 0.06;c1 = [120 150 230]/255;c2 = ([120 150 230]+0)/383;c3 = ([120 150 230]+128)/383;patch([0 1 1 0],[0 0 1 1],c1);patch([0 1 1 1-e 1-e 0+e],[0 0 1 1-e 0+e 0+e],c2);patch([0 0 1 1-e 0+e 0+e],[0 1 1 1-e 1-e 0+e],c3);plot([0 1 1 0 0],[0 0 1 1 0]);disp('weights');
  "IW{2,1}(175,:)'" : Constant  Value=[0.72217215343645957;-0.66903742695171364;-0.10242314493416457;1.018833764230008;0.72161421700818285;0.22189515186677078;0.19254459160618059;-0.45683014048433296;0.53534274244557611;0.011771515362042212]
      mask Display: e = 0.06;c1 = [120 150 230]/255;c2 = ([120 150 230]+0)/383;c3 = ([120 150 230]+128)/383;patch([0 1 1 0],[0 0 1 1],c1);patch([0 1 1 1-e 1-e 0+e],[0 0 1 1-e 0+e 0+e],c2);patch([0 0 1 1-e 0+e 0+e],[0 1 1 1-e 1-e 0+e],c3);plot([0 1 1 0 0],[0 0 1 1 0]);disp('weights');
  "IW{2,1}(176,:)'" : Constant  Value=[-0.7373269705752864;-0.90739110540597945;0.56376119251460188;-0.48156633527009346;0.02782465596027156;-0.27624888250573465;-0.856366138196477;0.47470746186210044;0.18931638585273874;-0.49351285377095633]
      mask Display: e = 0.06;c1 = [120 150 230]/255;c2 = ([120 150 230]+0)/383;c3 = ([120 150 230]+128)/383;patch([0 1 1 0],[0 0 1 1],c1);patch([0 1 1 1-e 1-e 0+e],[0 0 1 1-e 0+e 0+e],c2);patch([0 0 1 1-e 0+e 0+e],[0 1 1 1-e 1-e 0+e],c3);plot([0 1 1 0 0],[0 0 1 1 0]);disp('weights');
  "IW{2,1}(177,:)'" : Constant  Value=[0.10269823935240455;-0.30352664674513768;0.22093178649163309;0.71817796571774806;0.18936923658931637;0.40542095141755036;-0.19702640909188004;-0.440707627651236;0.59900206021414604;-0.74781703845442959]
      mask Display: e = 0.06;c1 = [120 150 230]/255;c2 = ([120 150 230]+0)/383;c3 = ([120 150 230]+128)/383;patch([0 1 1 0],[0 0 1 1],c1);patch([0 1 1 1-e 1-e 0+e],[0 0 1 1-e 0+e 0+e],c2);patch([0 0 1 1-e 0+e 0+e],[0 1 1 1-e 1-e 0+e],c3);plot([0 1 1 0 0],[0 0 1 1 0]);disp('weights');
  "IW{2,1}(178,:)'" : Constant  Value=[-0.36171886361001393;-0.18158881446760097;-0.745179397415204;-0.58052317446565205;0.24984348357947567;0.43177945705306553;-0.15354231227537943;-0.7202415269582757;-0.054053778329340926;0.37901139175012044]
      mask Display: e = 0.06;c1 = [120 150 230]/255;c2 = ([120 150 230]+0)/383;c3 = ([120 150 230]+128)/383;patch([0 1 1 0],[0 0 1 1],c1);patch([0 1 1 1-e 1-e 0+e],[0 0 1 1-e 0+e 0+e],c2);patch([0 0 1 1-e 0+e 0+e],[0 1 1 1-e 1-e 0+e],c3);plot([0 1 1 0 0],[0 0 1 1 0]);disp('weights');
  "IW{2,1}(179,:)'" : Constant  Value=[-0.092182278592989567;0.41337242390499912;0.55728343874011566;-0.87263068876906269;0.74220344764568724;0.76631460808129481;0.31201534345855264;-0.078516748860913477;0.52208645060422088;-0.75478621932196899]
      mask Display: e = 0.06;c1 = [120 150 230]/255;c2 = ([120 150 230]+0)/383;c3 = ([120 150 230]+128)/383;patch([0 1 1 0],[0 0 1 1],c1);patch([0 1 1 1-e 1-e 0+e],[0 0 1 1-e 0+e 0+e],c2);patch([0 0 1 1-e 0+e 0+e],[0 1 1 1-e 1-e 0+e],c3);plot([0 1 1 0 0],[0 0 1 1 0]);disp('weights');
  "IW{2,1}(18,:)'" : Constant  Value=[-0.25108895720467872;-0.093179752262753046;-1.1583518408841476;-1.1986576200001648;0.63971843648226867;0.22639251867300381;-0.1809504493495992;0.61776091742268402;-0.27179554259361055;0.0014167658363768432]
      mask Display: e = 0.06;c1 = [120 150 230]/255;c2 = ([120 150 230]+0)/383;c3 = ([120 150 230]+128)/383;patch([0 1 1 0],[0 0 1 1],c1);patch([0 1 1 1-e 1-e 0+e],[0 0 1 1-e 0+e 0+e],c2);patch([0 0 1 1-e 0+e 0+e],[0 1 1 1-e 1-e 0+e],c3);plot([0 1 1 0 0],[0 0 1 1 0]);disp('weights');
  "IW{2,1}(180,:)'" : Constant  Value=[0.85551308701337014;-0.31060855492951112;0.65255316019715592;0.82401074947796293;0.94011601181086735;0.13552939767779215;0.8035887975255811;0.53757944629404619;0.3186513042647619;0.41886670226367506]
      mask Display: e = 0.06;c1 = [120 150 230]/255;c2 = ([120 150 230]+0)/383;c3 = ([120 150 230]+128)/383;patch([0 1 1 0],[0 0 1 1],c1);patch([0 1 1 1-e 1-e 0+e],[0 0 1 1-e 0+e 0+e],c2);patch([0 0 1 1-e 0+e 0+e],[0 1 1 1-e 1-e 0+e],c3);plot([0 1 1 0 0],[0 0 1 1 0]);disp('weights');
  "IW{2,1}(181,:)'" : Constant  Value=[0.85049256938935047;0.32145161891390411;-0.69781514905558839;0.66679282776124471;-0.53513490708208145;0.39865543790669927;-0.130545513428522;-0.52857480499465515;0.72494884030690532;0.1605976655727967]
      mask Display: e = 0.06;c1 = [120 150 230]/255;c2 = ([120 150 230]+0)/383;c3 = ([120 150 230]+128)/383;patch([0 1 1 0],[0 0 1 1],c1);patch([0 1 1 1-e 1-e 0+e],[0 0 1 1-e 0+e 0+e],c2);patch([0 0 1 1-e 0+e 0+e],[0 1 1 1-e 1-e 0+e],c3);plot([0 1 1 0 0],[0 0 1 1 0]);disp('weights');
  "IW{2,1}(182,:)'" : Constant  Value=[-0.37603792495338156;-0.0099835123339639953;-1.3281817791639543;-0.86314832801347952;1.1728665682731454;0.19397703618908713;-0.18619213302364218;-0.17573168397270189;-0.012107716568831528;0.14348825668909582]
      mask Display: e = 0.06;c1 = [120 150 230]/255;c2 = ([120 150 230]+0)/383;c3 = ([120 150 230]+128)/383;patch([0 1 1 0],[0 0 1 1],c1);patch([0 1 1 1-e 1-e 0+e],[0 0 1 1-e 0+e 0+e],c2);patch([0 0 1 1-e 0+e 0+e],[0 1 1 1-e 1-e 0+e],c3);plot([0 1 1 0 0],[0 0 1 1 0]);disp('weights');
  "IW{2,1}(183,:)'" : Constant  Value=[0.16817333000559975;0.63100536433842369;0.54903222590035905;-0.49679287126849403;0.16875873793777552;0.36791315167548538;0.28663714554804509;-0.70714304785232318;1.4946680158414725;-0.46775720041362062]
      mask Display: e = 0.06;c1 = [120 150 230]/255;c2 = ([120 150 230]+0)/383;c3 = ([120 150 230]+128)/383;patch([0 1 1 0],[0 0 1 1],c1);patch([0 1 1 1-e 1-e 0+e],[0 0 1 1-e 0+e 0+e],c2);patch([0 0 1 1-e 0+e 0+e],[0 1 1 1-e 1-e 0+e],c3);plot([0 1 1 0 0],[0 0 1 1 0]);disp('weights');
  "IW{2,1}(184,:)'" : Constant  Value=[0.047934784280745629;-0.39575624193468595;-1.0959749537890722;0.30627341260610319;0.097091258045236939;0.31774041645006901;-0.67685934300876349;-0.76644321650823677;0.51451311834098856;0.90962500470855057]
      mask Display: e = 0.06;c1 = [120 150 230]/255;c2 = ([120 150 230]+0)/383;c3 = ([120 150 230]+128)/383;patch([0 1 1 0],[0 0 1 1],c1);patch([0 1 1 1-e 1-e 0+e],[0 0 1 1-e 0+e 0+e],c2);patch([0 0 1 1-e 0+e 0+e],[0 1 1 1-e 1-e 0+e],c3);plot([0 1 1 0 0],[0 0 1 1 0]);disp('weights');
  "IW{2,1}(185,:)'" : Constant  Value=[0.046537852836134763;-0.0062843468709279648;-0.37402446162115566;-0.40134023508785066;1.5477063429026801;0.17387883782123947;0.067541254576563403;0.25394819350228459;0.38512740575257087;0.018414650207841166]
      mask Display: e = 0.06;c1 = [120 150 230]/255;c2 = ([120 150 230]+0)/383;c3 = ([120 150 230]+128)/383;patch([0 1 1 0],[0 0 1 1],c1);patch([0 1 1 1-e 1-e 0+e],[0 0 1 1-e 0+e 0+e],c2);patch([0 0 1 1-e 0+e 0+e],[0 1 1 1-e 1-e 0+e],c3);plot([0 1 1 0 0],[0 0 1 1 0]);disp('weights');
  "IW{2,1}(186,:)'" : Constant  Value=[0.61759025866700457;-0.92994575187839823;0.93488927827575541;0.89045936940593584;1.258670562551607;0.11177485271907656;-0.65090925733832561;-0.078664566520097595;0.053694022227722848;-0.87541147860924684]
      mask Display: e = 0.06;c1 = [120 150 230]/255;c2 = ([120 150 230]+0)/383;c3 = ([120 150 230]+128)/383;patch([0 1 1 0],[0 0 1 1],c1);patch([0 1 1 1-e 1-e 0+e],[0 0 1 1-e 0+e 0+e],c2);patch([0 0 1 1-e 0+e 0+e],[0 1 1 1-e 1-e 0+e],c3);plot([0 1 1 0 0],[0 0 1 1 0]);disp('weights');
  "IW{2,1}(187,:)'" : Constant  Value=[0.76884480612180228;0.11329054637067972;-0.21942903182175491;0.67872109840551498;0.95164586301952836;0.35983963025737098;0.022897218012072645;-0.09090443777740459;-0.38171796290943411;0.55375590908588634]
      mask Display: e = 0.06;c1 = [120 150 230]/255;c2 = ([120 150 230]+0)/383;c3 = ([120 150 230]+128)/383;patch([0 1 1 0],[0 0 1 1],c1);patch([0 1 1 1-e 1-e 0+e],[0 0 1 1-e 0+e 0+e],c2);patch([0 0 1 1-e 0+e 0+e],[0 1 1 1-e 1-e 0+e],c3);plot([0 1 1 0 0],[0 0 1 1 0]);disp('weights');
  "IW{2,1}(188,:)'" : Constant  Value=[0.70358793376835527;-0.55796733425216383;-0.45706376825812789;0.4546269675628527;-0.073070748989446377;0.32145936767011574;0.56617430140181313;-0.47748983370511089;0.41123415995988094;0.66336490957639738]
      mask Display: e = 0.06;c1 = [120 150 230]/255;c2 = ([120 150 230]+0)/383;c3 = ([120 150 230]+128)/383;patch([0 1 1 0],[0 0 1 1],c1);patch([0 1 1 1-e 1-e 0+e],[0 0 1 1-e 0+e 0+e],c2);patch([0 0 1 1-e 0+e 0+e],[0 1 1 1-e 1-e 0+e],c3);plot([0 1 1 0 0],[0 0 1 1 0]);disp('weights');
  "IW{2,1}(189,:)'" : Constant  Value=[-0.32110456180561431;-1.2263767891329498;-0.26963321970240545;0.54117992498542966;0.83833156620162641;-0.04136760461162492;-0.94072550481154082;-0.65731100712463597;0.444982980735877;-0.59108501059979646]
      mask Display: e = 0.06;c1 = [120 150 230]/255;c2 = ([120 150 230]+0)/383;c3 = ([120 150 230]+128)/383;patch([0 1 1 0],[0 0 1 1],c1);patch([0 1 1 1-e 1-e 0+e],[0 0 1 1-e 0+e 0+e],c2);patch([0 0 1 1-e 0+e 0+e],[0 1 1 1-e 1-e 0+e],c3);plot([0 1 1 0 0],[0 0 1 1 0]);disp('weights');
  "IW{2,1}(19,:)'" : Constant  Value=[-0.42466338773943008;0.30525837946336959;-0.43246729879998019;-1.1535649631011169;-0.50626563841911876;0.22721417896560964;-0.63118235424394287;-0.28664722582486807;0.28187192581159864;0.24956707676893047]
      mask Display: e = 0.06;c1 = [120 150 230]/255;c2 = ([120 150 230]+0)/383;c3 = ([120 150 230]+128)/383;patch([0 1 1 0],[0 0 1 1],c1);patch([0 1 1 1-e 1-e 0+e],[0 0 1 1-e 0+e 0+e],c2);patch([0 0 1 1-e 0+e 0+e],[0 1 1 1-e 1-e 0+e],c3);plot([0 1 1 0 0],[0 0 1 1 0]);disp('weights');
  "IW{2,1}(190,:)'" : Constant  Value=[0.068537509287233872;-0.25316533762515925;0.49082108051414158;0.038079211205332475;0.10677706184554632;0.26916953009500449;-0.029698750456729511;-0.62706397497197064;0.93344251883839224;0.71886427879899073]
      mask Display: e = 0.06;c1 = [120 150 230]/255;c2 = ([120 150 230]+0)/383;c3 = ([120 150 230]+128)/383;patch([0 1 1 0],[0 0 1 1],c1);patch([0 1 1 1-e 1-e 0+e],[0 0 1 1-e 0+e 0+e],c2);patch([0 0 1 1-e 0+e 0+e],[0 1 1 1-e 1-e 0+e],c3);plot([0 1 1 0 0],[0 0 1 1 0]);disp('weights');
  "IW{2,1}(191,:)'" : Constant  Value=[-0.4927865989812209;-1.010137802556051;-0.63522639455978336;-0.26863243825246297;0.0263531740547778;-0.028208810575061805;-0.59552301125005558;0.12075910858384577;0.11140865234165143;0.77405125598200886]
      mask Display: e = 0.06;c1 = [120 150 230]/255;c2 = ([120 150 230]+0)/383;c3 = ([120 150 230]+128)/383;patch([0 1 1 0],[0 0 1 1],c1);patch([0 1 1 1-e 1-e 0+e],[0 0 1 1-e 0+e 0+e],c2);patch([0 0 1 1-e 0+e 0+e],[0 1 1 1-e 1-e 0+e],c3);plot([0 1 1 0 0],[0 0 1 1 0]);disp('weights');
  "IW{2,1}(192,:)'" : Constant  Value=[-0.35508200362027881;0.94706132028716239;0.46989663584233382;-0.8433788302485925;0.57999810590176826;1.0389219595562069;0.28379895359678009;-0.51398694395277977;0.52139856687887809;0.10668301990223852]
      mask Display: e = 0.06;c1 = [120 150 230]/255;c2 = ([120 150 230]+0)/383;c3 = ([120 150 230]+128)/383;patch([0 1 1 0],[0 0 1 1],c1);patch([0 1 1 1-e 1-e 0+e],[0 0 1 1-e 0+e 0+e],c2);patch([0 0 1 1-e 0+e 0+e],[0 1 1 1-e 1-e 0+e],c3);plot([0 1 1 0 0],[0 0 1 1 0]);disp('weights');
  "IW{2,1}(193,:)'" : Constant  Value=[0.24465911418136888;0.27608872625581377;0.15170135187990061;-0.51613386239583736;-0.44394926509277277;0.39454902502004685;0.16353108390186949;0.43957893086632388;-0.54388947883017535;0.27974083443819675]
      mask Display: e = 0.06;c1 = [120 150 230]/255;c2 = ([120 150 230]+0)/383;c3 = ([120 150 230]+128)/383;patch([0 1 1 0],[0 0 1 1],c1);patch([0 1 1 1-e 1-e 0+e],[0 0 1 1-e 0+e 0+e],c2);patch([0 0 1 1-e 0+e 0+e],[0 1 1 1-e 1-e 0+e],c3);plot([0 1 1 0 0],[0 0 1 1 0]);disp('weights');
  "IW{2,1}(194,:)'" : Constant  Value=[0.47078374800802336;-0.32947934122827388;-0.45952905102777986;-0.53009841622510789;-0.55905423526645204;-0.44796068088372587;-1.0912203084322505;-0.20628949073363131;-0.77994015298617447;-0.6343331343812868]
      mask Display: e = 0.06;c1 = [120 150 230]/255;c2 = ([120 150 230]+0)/383;c3 = ([120 150 230]+128)/383;patch([0 1 1 0],[0 0 1 1],c1);patch([0 1 1 1-e 1-e 0+e],[0 0 1 1-e 0+e 0+e],c2);patch([0 0 1 1-e 0+e 0+e],[0 1 1 1-e 1-e 0+e],c3);plot([0 1 1 0 0],[0 0 1 1 0]);disp('weights');
  "IW{2,1}(195,:)'" : Constant  Value=[-0.22384741006970438;0.065343623252045707;-0.6524115814439666;-0.42393982071009739;-0.43987623838173229;0.38576026597986673;0.21575954523952179;-0.48632729101776229;-0.19020413942221132;0.90922376853824127]
      mask Display: e = 0.06;c1 = [120 150 230]/255;c2 = ([120 150 230]+0)/383;c3 = ([120 150 230]+128)/383;patch([0 1 1 0],[0 0 1 1],c1);patch([0 1 1 1-e 1-e 0+e],[0 0 1 1-e 0+e 0+e],c2);patch([0 0 1 1-e 0+e 0+e],[0 1 1 1-e 1-e 0+e],c3);plot([0 1 1 0 0],[0 0 1 1 0]);disp('weights');
  "IW{2,1}(196,:)'" : Constant  Value=[-0.26431345529015293;-0.20147583687366455;0.02822469528429572;-0.014445151914472876;0.048333138607184689;-0.072064632745538315;0.24803174662007194;-0.60429093322208316;1.31439641348351;-0.14707347828765271]
      mask Display: e = 0.06;c1 = [120 150 230]/255;c2 = ([120 150 230]+0)/383;c3 = ([120 150 230]+128)/383;patch([0 1 1 0],[0 0 1 1],c1);patch([0 1 1 1-e 1-e 0+e],[0 0 1 1-e 0+e 0+e],c2);patch([0 0 1 1-e 0+e 0+e],[0 1 1 1-e 1-e 0+e],c3);plot([0 1 1 0 0],[0 0 1 1 0]);disp('weights');
  "IW{2,1}(197,:)'" : Constant  Value=[0.20802221234898938;-0.22721838625378779;0.10045488554222855;0.52692609166272075;-0.82060639733571661;0.47539644727342345;-0.29116438496536468;0.42767627109377976;0.17015301828332521;0.78947831663936585]
      mask Display: e = 0.06;c1 = [120 150 230]/255;c2 = ([120 150 230]+0)/383;c3 = ([120 150 230]+128)/383;patch([0 1 1 0],[0 0 1 1],c1);patch([0 1 1 1-e 1-e 0+e],[0 0 1 1-e 0+e 0+e],c2);patch([0 0 1 1-e 0+e 0+e],[0 1 1 1-e 1-e 0+e],c3);plot([0 1 1 0 0],[0 0 1 1 0]);disp('weights');
  "IW{2,1}(198,:)'" : Constant  Value=[0.42099525080402705;0.46525784710580842;-0.1242949312516361;-0.5487899104190973;0.57248605256128349;-0.27937504230969046;-1.3174899428052336;-0.0025540508195908973;-0.20213103084916789;-0.16985247156171523]
      mask Display: e = 0.06;c1 = [120 150 230]/255;c2 = ([120 150 230]+0)/383;c3 = ([120 150 230]+128)/383;patch([0 1 1 0],[0 0 1 1],c1);patch([0 1 1 1-e 1-e 0+e],[0 0 1 1-e 0+e 0+e],c2);patch([0 0 1 1-e 0+e 0+e],[0 1 1 1-e 1-e 0+e],c3);plot([0 1 1 0 0],[0 0 1 1 0]);disp('weights');
  "IW{2,1}(199,:)'" : Constant  Value=[-0.23117054456329983;-0.5321444346425197;-0.65304074440914728;-0.62217423440882302;1.2676055555517332;0.41300397965323249;0.61218365726099278;0.61556940114801761;-0.1874023035490433;-0.65886423604674682]
      mask Display: e = 0.06;c1 = [120 150 230]/255;c2 = ([120 150 230]+0)/383;c3 = ([120 150 230]+128)/383;patch([0 1 1 0],[0 0 1 1],c1);patch([0 1 1 1-e 1-e 0+e],[0 0 1 1-e 0+e 0+e],c2);patch([0 0 1 1-e 0+e 0+e],[0 1 1 1-e 1-e 0+e],c3);plot([0 1 1 0 0],[0 0 1 1 0]);disp('weights');
  "IW{2,1}(2,:)'" : Constant  Value=[0.25949474513700821;0.27404905561003717;0.24689148904879843;-0.27900883154251277;0.026418089508562947;-0.16549248779253889;-0.66848679485546136;-0.18877728693607593;0.68189394237642176;-1.0292156166463777]
      mask Display: e = 0.06;c1 = [120 150 230]/255;c2 = ([120 150 230]+0)/383;c3 = ([120 150 230]+128)/383;patch([0 1 1 0],[0 0 1 1],c1);patch([0 1 1 1-e 1-e 0+e],[0 0 1 1-e 0+e 0+e],c2);patch([0 0 1 1-e 0+e 0+e],[0 1 1 1-e 1-e 0+e],c3);plot([0 1 1 0 0],[0 0 1 1 0]);disp('weights');
  "IW{2,1}(20,:)'" : Constant  Value=[-0.19545683452662219;0.50875214343101505;0.66654983585370642;-1.0535271615333135;-0.46270573105690765;0.69351314666331454;-0.032681624300444342;0.44314299974200017;-0.30959621197586668;-0.28439955807584327]
      mask Display: e = 0.06;c1 = [120 150 230]/255;c2 = ([120 150 230]+0)/383;c3 = ([120 150 230]+128)/383;patch([0 1 1 0],[0 0 1 1],c1);patch([0 1 1 1-e 1-e 0+e],[0 0 1 1-e 0+e 0+e],c2);patch([0 0 1 1-e 0+e 0+e],[0 1 1 1-e 1-e 0+e],c3);plot([0 1 1 0 0],[0 0 1 1 0]);disp('weights');
  "IW{2,1}(200,:)'" : Constant  Value=[-0.72899873579023677;-0.37936256536626978;0.63724945914508635;-0.33756626789769151;0.73649645979662914;0.64136803888965099;-0.053590218177324428;-0.31298479545605379;0.3190340057275638;0.41508454219615926]
      mask Display: e = 0.06;c1 = [120 150 230]/255;c2 = ([120 150 230]+0)/383;c3 = ([120 150 230]+128)/383;patch([0 1 1 0],[0 0 1 1],c1);patch([0 1 1 1-e 1-e 0+e],[0 0 1 1-e 0+e 0+e],c2);patch([0 0 1 1-e 0+e 0+e],[0 1 1 1-e 1-e 0+e],c3);plot([0 1 1 0 0],[0 0 1 1 0]);disp('weights');
  "IW{2,1}(201,:)'" : Constant  Value=[0.92340333043975265;-0.0039808182425180028;-0.046844512802280011;-0.34763059017447517;-0.1267756517840104;-0.19812607805181814;0.31023516072429325;0.56543241203741068;0.095077584589467135;-0.66491864721197458]
      mask Display: e = 0.06;c1 = [120 150 230]/255;c2 = ([120 150 230]+0)/383;c3 = ([120 150 230]+128)/383;patch([0 1 1 0],[0 0 1 1],c1);patch([0 1 1 1-e 1-e 0+e],[0 0 1 1-e 0+e 0+e],c2);patch([0 0 1 1-e 0+e 0+e],[0 1 1 1-e 1-e 0+e],c3);plot([0 1 1 0 0],[0 0 1 1 0]);disp('weights');
  "IW{2,1}(202,:)'" : Constant  Value=[0.46312235821641756;0.5559448238418957;0.18093720218458409;-0.24065938651651231;0.86294613845269952;0.56838426897923244;0.5738945385310037;-0.05309197528972058;1.2565388129265169;-0.20107442312165602]
      mask Display: e = 0.06;c1 = [120 150 230]/255;c2 = ([120 150 230]+0)/383;c3 = ([120 150 230]+128)/383;patch([0 1 1 0],[0 0 1 1],c1);patch([0 1 1 1-e 1-e 0+e],[0 0 1 1-e 0+e 0+e],c2);patch([0 0 1 1-e 0+e 0+e],[0 1 1 1-e 1-e 0+e],c3);plot([0 1 1 0 0],[0 0 1 1 0]);disp('weights');
  "IW{2,1}(203,:)'" : Constant  Value=[0.50630743154547242;-0.51395221199921903;0.8199556135957452;0.50085566911179669;-0.64232154587450641;-0.057979383595117229;0.16322308534987262;-0.28332042741319902;0.62246227342986504;-0.63567211574527049]
      mask Display: e = 0.06;c1 = [120 150 230]/255;c2 = ([120 150 230]+0)/383;c3 = ([120 150 230]+128)/383;patch([0 1 1 0],[0 0 1 1],c1);patch([0 1 1 1-e 1-e 0+e],[0 0 1 1-e 0+e 0+e],c2);patch([0 0 1 1-e 0+e 0+e],[0 1 1 1-e 1-e 0+e],c3);plot([0 1 1 0 0],[0 0 1 1 0]);disp('weights');
  "IW{2,1}(204,:)'" : Constant  Value=[-0.66968452976597581;0.092865303655802089;-0.60992566012051364;-1.2244707935701307;0.64085097511385913;0.48666688235405697;0.55290514547448466;-0.7096068043461472;0.21973430669400296;-0.029957128558043777]
      mask Display: e = 0.06;c1 = [120 150 230]/255;c2 = ([120 150 230]+0)/383;c3 = ([120 150 230]+128)/383;patch([0 1 1 0],[0 0 1 1],c1);patch([0 1 1 1-e 1-e 0+e],[0 0 1 1-e 0+e 0+e],c2);patch([0 0 1 1-e 0+e 0+e],[0 1 1 1-e 1-e 0+e],c3);plot([0 1 1 0 0],[0 0 1 1 0]);disp('weights');
  "IW{2,1}(205,:)'" : Constant  Value=[0.11397993506061543;-0.42798673212952532;-0.13718165410915778;0.48726746852653796;-0.084421798623953548;-0.23622739608265009;-0.85987350105819771;-0.36294441940663974;-0.21612462443617386;0.11731792628614579]
      mask Display: e = 0.06;c1 = [120 150 230]/255;c2 = ([120 150 230]+0)/383;c3 = ([120 150 230]+128)/383;patch([0 1 1 0],[0 0 1 1],c1);patch([0 1 1 1-e 1-e 0+e],[0 0 1 1-e 0+e 0+e],c2);patch([0 0 1 1-e 0+e 0+e],[0 1 1 1-e 1-e 0+e],c3);plot([0 1 1 0 0],[0 0 1 1 0]);disp('weights');
  "IW{2,1}(206,:)'" : Constant  Value=[0.057318410942542197;-0.76850256118465377;-0.53145164584056626;-0.36944081061591505;-0.2441054311638714;0.026461896444463173;0.35882347355104577;0.18623345523413559;-0.14954928892099145;0.75454904401198264]
      mask Display: e = 0.06;c1 = [120 150 230]/255;c2 = ([120 150 230]+0)/383;c3 = ([120 150 230]+128)/383;patch([0 1 1 0],[0 0 1 1],c1);patch([0 1 1 1-e 1-e 0+e],[0 0 1 1-e 0+e 0+e],c2);patch([0 0 1 1-e 0+e 0+e],[0 1 1 1-e 1-e 0+e],c3);plot([0 1 1 0 0],[0 0 1 1 0]);disp('weights');
  "IW{2,1}(207,:)'" : Constant  Value=[0.19356060696320265;-0.06106389421450388;-0.59874036118572938;0.21964758165026138;0.51145415801312055;0.74301144123098883;0.75249351939945941;-0.58733170812658941;-0.00091217610775649882;-0.10879235041151854]
      mask Display: e = 0.06;c1 = [120 150 230]/255;c2 = ([120 150 230]+0)/383;c3 = ([120 150 230]+128)/383;patch([0 1 1 0],[0 0 1 1],c1);patch([0 1 1 1-e 1-e 0+e],[0 0 1 1-e 0+e 0+e],c2);patch([0 0 1 1-e 0+e 0+e],[0 1 1 1-e 1-e 0+e],c3);plot([0 1 1 0 0],[0 0 1 1 0]);disp('weights');
  "IW{2,1}(208,:)'" : Constant  Value=[-0.74248088429949866;-0.54201161233097661;1.1567315469730624;-1.0829767846213416;0.040741747913651982;-0.17994590602310034;0.11151391403344207;-0.37906942028107082;0.040505884534297654;-0.78942496529865402]
      mask Display: e = 0.06;c1 = [120 150 230]/255;c2 = ([120 150 230]+0)/383;c3 = ([120 150 230]+128)/383;patch([0 1 1 0],[0 0 1 1],c1);patch([0 1 1 1-e 1-e 0+e],[0 0 1 1-e 0+e 0+e],c2);patch([0 0 1 1-e 0+e 0+e],[0 1 1 1-e 1-e 0+e],c3);plot([0 1 1 0 0],[0 0 1 1 0]);disp('weights');
  "IW{2,1}(209,:)'" : Constant  Value=[-0.14067190073031863;-0.59765516264259455;0.20644246549840942;0.067880711918986869;-0.49194999549194507;0.47381699262228638;0.6517713703284721;-0.35305027350426343;0.98379903876694208;-0.94184722600465365]
      mask Display: e = 0.06;c1 = [120 150 230]/255;c2 = ([120 150 230]+0)/383;c3 = ([120 150 230]+128)/383;patch([0 1 1 0],[0 0 1 1],c1);patch([0 1 1 1-e 1-e 0+e],[0 0 1 1-e 0+e 0+e],c2);patch([0 0 1 1-e 0+e 0+e],[0 1 1 1-e 1-e 0+e],c3);plot([0 1 1 0 0],[0 0 1 1 0]);disp('weights');
  "IW{2,1}(21,:)'" : Constant  Value=[0.45366992966853942;0.45490326884659449;1.0963158012115111;0.038509984295997557;0.83970623573865011;0.84604954973911906;-0.33756223820403514;-0.55246614682097284;0.0027237819748140157;-0.53030398742179741]
      mask Display: e = 0.06;c1 = [120 150 230]/255;c2 = ([120 150 230]+0)/383;c3 = ([120 150 230]+128)/383;patch([0 1 1 0],[0 0 1 1],c1);patch([0 1 1 1-e 1-e 0+e],[0 0 1 1-e 0+e 0+e],c2);patch([0 0 1 1-e 0+e 0+e],[0 1 1 1-e 1-e 0+e],c3);plot([0 1 1 0 0],[0 0 1 1 0]);disp('weights');
  "IW{2,1}(210,:)'" : Constant  Value=[0.69979671629031182;0.30677801418354911;0.54343427450080339;-0.43028518684601869;0.31769496357554239;-0.049317525554840591;-1.0009586799619743;-0.57280580259329372;0.043857896376099381;-0.7405139701563942]
      mask Display: e = 0.06;c1 = [120 150 230]/255;c2 = ([120 150 230]+0)/383;c3 = ([120 150 230]+128)/383;patch([0 1 1 0],[0 0 1 1],c1);patch([0 1 1 1-e 1-e 0+e],[0 0 1 1-e 0+e 0+e],c2);patch([0 0 1 1-e 0+e 0+e],[0 1 1 1-e 1-e 0+e],c3);plot([0 1 1 0 0],[0 0 1 1 0]);disp('weights');
  "IW{2,1}(211,:)'" : Constant  Value=[0.62604944877521651;-0.37925081658834692;-0.53008971219512602;0.91974505169613041;-0.52255465391473155;0.59748339042701915;0.95915232451125432;-0.18538599727052135;0.50787051618320156;0.98059747139836251]
      mask Display: e = 0.06;c1 = [120 150 230]/255;c2 = ([120 150 230]+0)/383;c3 = ([120 150 230]+128)/383;patch([0 1 1 0],[0 0 1 1],c1);patch([0 1 1 1-e 1-e 0+e],[0 0 1 1-e 0+e 0+e],c2);patch([0 0 1 1-e 0+e 0+e],[0 1 1 1-e 1-e 0+e],c3);plot([0 1 1 0 0],[0 0 1 1 0]);disp('weights');
  "IW{2,1}(212,:)'" : Constant  Value=[0.41823345617651103;-0.43666910727142944;0.29172348451702695;0.43400210441702458;-0.3871376872531358;0.020606682798345988;-0.16477698825132792;-0.65277867854046145;1.1388090399224922;0.10812541283196375]
      mask Display: e = 0.06;c1 = [120 150 230]/255;c2 = ([120 150 230]+0)/383;c3 = ([120 150 230]+128)/383;patch([0 1 1 0],[0 0 1 1],c1);patch([0 1 1 1-e 1-e 0+e],[0 0 1 1-e 0+e 0+e],c2);patch([0 0 1 1-e 0+e 0+e],[0 1 1 1-e 1-e 0+e],c3);plot([0 1 1 0 0],[0 0 1 1 0]);disp('weights');
  "IW{2,1}(213,:)'" : Constant  Value=[0.20452461099923058;0.20512375872234967;-1.1592637016623766;-0.42851575303103573;0.018965975686606906;0.054003192355522867;-0.45606473533841008;-0.57722303569832456;-0.024158750462212553;-0.078465273555406445]
      mask Display: e = 0.06;c1 = [120 150 230]/255;c2 = ([120 150 230]+0)/383;c3 = ([120 150 230]+128)/383;patch([0 1 1 0],[0 0 1 1],c1);patch([0 1 1 1-e 1-e 0+e],[0 0 1 1-e 0+e 0+e],c2);patch([0 0 1 1-e 0+e 0+e],[0 1 1 1-e 1-e 0+e],c3);plot([0 1 1 0 0],[0 0 1 1 0]);disp('weights');
  "IW{2,1}(214,:)'" : Constant  Value=[-0.65797789102452364;-0.78501171646642154;0.77482520286555356;-0.45241603450117074;-1.1010387876735175;0.6768652814625653;0.62567385366432893;0.013222094140427548;0.19100910087746462;-0.52425071311504179]
      mask Display: e = 0.06;c1 = [120 150 230]/255;c2 = ([120 150 230]+0)/383;c3 = ([120 150 230]+128)/383;patch([0 1 1 0],[0 0 1 1],c1);patch([0 1 1 1-e 1-e 0+e],[0 0 1 1-e 0+e 0+e],c2);patch([0 0 1 1-e 0+e 0+e],[0 1 1 1-e 1-e 0+e],c3);plot([0 1 1 0 0],[0 0 1 1 0]);disp('weights');
  "IW{2,1}(215,:)'" : Constant  Value=[0.25385949863730967;-0.42425435325696387;-0.23758765824961753;-0.16024225066118145;-0.16128618270470124;0.55772629709647092;0.059456086377371514;0.12400159540683586;-0.4487096867553178;-0.22321780024873006]
      mask Display: e = 0.06;c1 = [120 150 230]/255;c2 = ([120 150 230]+0)/383;c3 = ([120 150 230]+128)/383;patch([0 1 1 0],[0 0 1 1],c1);patch([0 1 1 1-e 1-e 0+e],[0 0 1 1-e 0+e 0+e],c2);patch([0 0 1 1-e 0+e 0+e],[0 1 1 1-e 1-e 0+e],c3);plot([0 1 1 0 0],[0 0 1 1 0]);disp('weights');
  "IW{2,1}(216,:)'" : Constant  Value=[-0.45399020879708624;-0.85092489890020429;0.82291761620260195;0.0027024967174258535;-1.1570883685183611;0.55438872885640511;0.57186746971162639;-0.018073135208704988;-0.49705820867955003;-0.36219229723637014]
      mask Display: e = 0.06;c1 = [120 150 230]/255;c2 = ([120 150 230]+0)/383;c3 = ([120 150 230]+128)/383;patch([0 1 1 0],[0 0 1 1],c1);patch([0 1 1 1-e 1-e 0+e],[0 0 1 1-e 0+e 0+e],c2);patch([0 0 1 1-e 0+e 0+e],[0 1 1 1-e 1-e 0+e],c3);plot([0 1 1 0 0],[0 0 1 1 0]);disp('weights');
  "IW{2,1}(217,:)'" : Constant  Value=[0.046537895895906872;0.57081299424710785;0.67472935489505914;-0.15913146877979181;-0.97303556922561885;0.56870376496188313;-0.74970415207164864;-0.36160148224727673;-0.27413347494930995;-0.69833416781866386]
      mask Display: e = 0.06;c1 = [120 150 230]/255;c2 = ([120 150 230]+0)/383;c3 = ([120 150 230]+128)/383;patch([0 1 1 0],[0 0 1 1],c1);patch([0 1 1 1-e 1-e 0+e],[0 0 1 1-e 0+e 0+e],c2);patch([0 0 1 1-e 0+e 0+e],[0 1 1 1-e 1-e 0+e],c3);plot([0 1 1 0 0],[0 0 1 1 0]);disp('weights');
  "IW{2,1}(218,:)'" : Constant  Value=[0.82035931459752531;-0.37025359423496162;0.84633906045049256;-0.19068053153299838;-0.38843410044274973;-0.18531375242106884;0.1601042248796761;0.53175716795355565;-0.51993315777636062;-0.63993543260717067]
      mask Display: e = 0.06;c1 = [120 150 230]/255;c2 = ([120 150 230]+0)/383;c3 = ([120 150 230]+128)/383;patch([0 1 1 0],[0 0 1 1],c1);patch([0 1 1 1-e 1-e 0+e],[0 0 1 1-e 0+e 0+e],c2);patch([0 0 1 1-e 0+e 0+e],[0 1 1 1-e 1-e 0+e],c3);plot([0 1 1 0 0],[0 0 1 1 0]);disp('weights');
  "IW{2,1}(219,:)'" : Constant  Value=[0.75708640080133138;0.51796085250254742;-0.1921176650981152;-0.82348906698187885;-0.35075375855277846;0.056447690110284165;-0.27613828683470198;0.15580568606706857;-0.27860236892548285;-0.80119851338716686]
      mask Display: e = 0.06;c1 = [120 150 230]/255;c2 = ([120 150 230]+0)/383;c3 = ([120 150 230]+128)/383;patch([0 1 1 0],[0 0 1 1],c1);patch([0 1 1 1-e 1-e 0+e],[0 0 1 1-e 0+e 0+e],c2);patch([0 0 1 1-e 0+e 0+e],[0 1 1 1-e 1-e 0+e],c3);plot([0 1 1 0 0],[0 0 1 1 0]);disp('weights');
  "IW{2,1}(22,:)'" : Constant  Value=[0.27330482480698859;-0.14893393251111636;-0.30858673727969876;-0.74971249354603509;0.44963816242251808;-0.0076434553255140814;-1.04120380390606;-0.66316621569652057;1.0953212525925315;-1.0731901723106909]
      mask Display: e = 0.06;c1 = [120 150 230]/255;c2 = ([120 150 230]+0)/383;c3 = ([120 150 230]+128)/383;patch([0 1 1 0],[0 0 1 1],c1);patch([0 1 1 1-e 1-e 0+e],[0 0 1 1-e 0+e 0+e],c2);patch([0 0 1 1-e 0+e 0+e],[0 1 1 1-e 1-e 0+e],c3);plot([0 1 1 0 0],[0 0 1 1 0]);disp('weights');
  "IW{2,1}(220,:)'" : Constant  Value=[-0.1378045758833997;-0.17112826911304735;0.18979690251548573;-0.68394205149599541;0.26282245408208055;0.55548630236333074;-0.062090838979711863;-0.58062077075172491;0.21151225500264484;-0.70494915304989825]
      mask Display: e = 0.06;c1 = [120 150 230]/255;c2 = ([120 150 230]+0)/383;c3 = ([120 150 230]+128)/383;patch([0 1 1 0],[0 0 1 1],c1);patch([0 1 1 1-e 1-e 0+e],[0 0 1 1-e 0+e 0+e],c2);patch([0 0 1 1-e 0+e 0+e],[0 1 1 1-e 1-e 0+e],c3);plot([0 1 1 0 0],[0 0 1 1 0]);disp('weights');
  "IW{2,1}(221,:)'" : Constant  Value=[0.56476289770092802;-0.18812300511214045;-0.80313903630386296;0.16470559612680719;-0.54122932557280512;0.082224238028203889;-0.79622612801027137;-0.53290350614427451;-0.31766899743896132;-0.32850527709830024]
      mask Display: e = 0.06;c1 = [120 150 230]/255;c2 = ([120 150 230]+0)/383;c3 = ([120 150 230]+128)/383;patch([0 1 1 0],[0 0 1 1],c1);patch([0 1 1 1-e 1-e 0+e],[0 0 1 1-e 0+e 0+e],c2);patch([0 0 1 1-e 0+e 0+e],[0 1 1 1-e 1-e 0+e],c3);plot([0 1 1 0 0],[0 0 1 1 0]);disp('weights');
  "IW{2,1}(222,:)'" : Constant  Value=[-0.50392444311761031;-0.70284240031256884;0.52823726164178675;0.07354418000521093;0.099473021540476103;0.68731454058406816;0.53957384237918349;-0.42436142207589655;-0.41524379955097024;-0.72051948528538023]
      mask Display: e = 0.06;c1 = [120 150 230]/255;c2 = ([120 150 230]+0)/383;c3 = ([120 150 230]+128)/383;patch([0 1 1 0],[0 0 1 1],c1);patch([0 1 1 1-e 1-e 0+e],[0 0 1 1-e 0+e 0+e],c2);patch([0 0 1 1-e 0+e 0+e],[0 1 1 1-e 1-e 0+e],c3);plot([0 1 1 0 0],[0 0 1 1 0]);disp('weights');
  "IW{2,1}(223,:)'" : Constant  Value=[-0.48937429220612105;-0.5025442026922281;0.86113551104477548;-0.54102363680258558;0.52852391284094924;0.29626566341420718;0.8795190075321645;0.37282218899900943;1.05095808866757;0.18432388986475123]
      mask Display: e = 0.06;c1 = [120 150 230]/255;c2 = ([120 150 230]+0)/383;c3 = ([120 150 230]+128)/383;patch([0 1 1 0],[0 0 1 1],c1);patch([0 1 1 1-e 1-e 0+e],[0 0 1 1-e 0+e 0+e],c2);patch([0 0 1 1-e 0+e 0+e],[0 1 1 1-e 1-e 0+e],c3);plot([0 1 1 0 0],[0 0 1 1 0]);disp('weights');
  "IW{2,1}(224,:)'" : Constant  Value=[-0.070270595508442835;-0.34786746760055287;-0.09019422850349107;0.43129161510178093;-0.019131182553020099;0.093862969379661654;0.14903585396370678;-0.050009686413069271;0.593312080235182;0.41424077556211947]
      mask Display: e = 0.06;c1 = [120 150 230]/255;c2 = ([120 150 230]+0)/383;c3 = ([120 150 230]+128)/383;patch([0 1 1 0],[0 0 1 1],c1);patch([0 1 1 1-e 1-e 0+e],[0 0 1 1-e 0+e 0+e],c2);patch([0 0 1 1-e 0+e 0+e],[0 1 1 1-e 1-e 0+e],c3);plot([0 1 1 0 0],[0 0 1 1 0]);disp('weights');
  "IW{2,1}(225,:)'" : Constant  Value=[-0.46678996394800742;-1.0647699571919316;-0.31842507769472173;-0.30074211336720719;1.2806220304878604;-0.0089895963763926279;-0.59886725005903585;-0.34787107477473217;0.80306159587915737;-0.79727156091609785]
      mask Display: e = 0.06;c1 = [120 150 230]/255;c2 = ([120 150 230]+0)/383;c3 = ([120 150 230]+128)/383;patch([0 1 1 0],[0 0 1 1],c1);patch([0 1 1 1-e 1-e 0+e],[0 0 1 1-e 0+e 0+e],c2);patch([0 0 1 1-e 0+e 0+e],[0 1 1 1-e 1-e 0+e],c3);plot([0 1 1 0 0],[0 0 1 1 0]);disp('weights');
  "IW{2,1}(226,:)'" : Constant  Value=[1.3154441576336888;0.29821617835534953;-0.31389922754018473;0.53506155391716836;-0.24903222661910279;-0.28689821375871516;-0.16983587607237485;-0.099355267256668239;1.0795772567121036;-0.34992750408549916]
      mask Display: e = 0.06;c1 = [120 150 230]/255;c2 = ([120 150 230]+0)/383;c3 = ([120 150 230]+128)/383;patch([0 1 1 0],[0 0 1 1],c1);patch([0 1 1 1-e 1-e 0+e],[0 0 1 1-e 0+e 0+e],c2);patch([0 0 1 1-e 0+e 0+e],[0 1 1 1-e 1-e 0+e],c3);plot([0 1 1 0 0],[0 0 1 1 0]);disp('weights');
  "IW{2,1}(227,:)'" : Constant  Value=[0.020513355990515181;-0.1910624099566646;0.29444829112962156;-0.094727456487779776;0.89907908706386896;0.62749431410729106;0.16111451951283853;0.41401546155882812;-0.14281605679236098;-0.13505124096436083]
      mask Display: e = 0.06;c1 = [120 150 230]/255;c2 = ([120 150 230]+0)/383;c3 = ([120 150 230]+128)/383;patch([0 1 1 0],[0 0 1 1],c1);patch([0 1 1 1-e 1-e 0+e],[0 0 1 1-e 0+e 0+e],c2);patch([0 0 1 1-e 0+e 0+e],[0 1 1 1-e 1-e 0+e],c3);plot([0 1 1 0 0],[0 0 1 1 0]);disp('weights');
  "IW{2,1}(228,:)'" : Constant  Value=[0.33139652012830351;-0.032003466176489248;-0.55357573135634774;0.14595016159271385;0.89017271071574666;0.012482538612546557;-0.91111157554264477;-0.81939318744028222;0.92010569550519561;-1.2161823481630396]
      mask Display: e = 0.06;c1 = [120 150 230]/255;c2 = ([120 150 230]+0)/383;c3 = ([120 150 230]+128)/383;patch([0 1 1 0],[0 0 1 1],c1);patch([0 1 1 1-e 1-e 0+e],[0 0 1 1-e 0+e 0+e],c2);patch([0 0 1 1-e 0+e 0+e],[0 1 1 1-e 1-e 0+e],c3);plot([0 1 1 0 0],[0 0 1 1 0]);disp('weights');
  "IW{2,1}(229,:)'" : Constant  Value=[0.56947152675786716;-0.091677599634437446;-0.77355033261405948;-0.35570583337065709;0.34982387111194035;-0.36444094799989757;-0.5138384591163313;-0.88053383084989312;1.0016652394648762;-0.90501063044679286]
      mask Display: e = 0.06;c1 = [120 150 230]/255;c2 = ([120 150 230]+0)/383;c3 = ([120 150 230]+128)/383;patch([0 1 1 0],[0 0 1 1],c1);patch([0 1 1 1-e 1-e 0+e],[0 0 1 1-e 0+e 0+e],c2);patch([0 0 1 1-e 0+e 0+e],[0 1 1 1-e 1-e 0+e],c3);plot([0 1 1 0 0],[0 0 1 1 0]);disp('weights');
  "IW{2,1}(23,:)'" : Constant  Value=[1.50575939144251;0.018187922474404816;-0.55565556100398616;0.27785366714477056;0.60627506863689673;0.1723379882080146;0.29362726167786629;0.56103092995246295;-0.50922520490367429;-0.94858523765997949]
      mask Display: e = 0.06;c1 = [120 150 230]/255;c2 = ([120 150 230]+0)/383;c3 = ([120 150 230]+128)/383;patch([0 1 1 0],[0 0 1 1],c1);patch([0 1 1 1-e 1-e 0+e],[0 0 1 1-e 0+e 0+e],c2);patch([0 0 1 1-e 0+e 0+e],[0 1 1 1-e 1-e 0+e],c3);plot([0 1 1 0 0],[0 0 1 1 0]);disp('weights');
  "IW{2,1}(230,:)'" : Constant  Value=[0.59554299499571561;-0.51755402360636515;-0.10570615406539717;0.40072573920502708;-0.81067750126657634;-0.17374352680539151;0.028037491157477057;-0.36789528339875155;0.28537060906358558;-0.61144628107571164]
      mask Display: e = 0.06;c1 = [120 150 230]/255;c2 = ([120 150 230]+0)/383;c3 = ([120 150 230]+128)/383;patch([0 1 1 0],[0 0 1 1],c1);patch([0 1 1 1-e 1-e 0+e],[0 0 1 1-e 0+e 0+e],c2);patch([0 0 1 1-e 0+e 0+e],[0 1 1 1-e 1-e 0+e],c3);plot([0 1 1 0 0],[0 0 1 1 0]);disp('weights');
  "IW{2,1}(231,:)'" : Constant  Value=[-0.62812309307326164;-0.65427470678046318;0.031781872968657143;-0.5294037151727653;-0.17483239368891901;-0.152647022838581;0.1400772152186826;-0.71033896401457075;1.394845786109274;0.66752264729044875]
      mask Display: e = 0.06;c1 = [120 150 230]/255;c2 = ([120 150 230]+0)/383;c3 = ([120 150 230]+128)/383;patch([0 1 1 0],[0 0 1 1],c1);patch([0 1 1 1-e 1-e 0+e],[0 0 1 1-e 0+e 0+e],c2);patch([0 0 1 1-e 0+e 0+e],[0 1 1 1-e 1-e 0+e],c3);plot([0 1 1 0 0],[0 0 1 1 0]);disp('weights');
  "IW{2,1}(232,:)'" : Constant  Value=[-0.13184734214167013;-0.87147983478940083;-0.83645272417824879;-0.19447552595217585;1.3270532112742985;-0.26015513914574884;-0.92785635963865043;0.10335036359074506;-0.59042116042330983;-0.30837729681330217]
      mask Display: e = 0.06;c1 = [120 150 230]/255;c2 = ([120 150 230]+0)/383;c3 = ([120 150 230]+128)/383;patch([0 1 1 0],[0 0 1 1],c1);patch([0 1 1 1-e 1-e 0+e],[0 0 1 1-e 0+e 0+e],c2);patch([0 0 1 1-e 0+e 0+e],[0 1 1 1-e 1-e 0+e],c3);plot([0 1 1 0 0],[0 0 1 1 0]);disp('weights');
  "IW{2,1}(233,:)'" : Constant  Value=[0.41708916594289669;-0.23319094515920535;-0.32914652551994117;0.77370900690419842;0.57791226940695595;0.31782815565784128;-0.22091140196478759;0.11695500675117387;-0.68661026154823546;0.44047821956700861]
      mask Display: e = 0.06;c1 = [120 150 230]/255;c2 = ([120 150 230]+0)/383;c3 = ([120 150 230]+128)/383;patch([0 1 1 0],[0 0 1 1],c1);patch([0 1 1 1-e 1-e 0+e],[0 0 1 1-e 0+e 0+e],c2);patch([0 0 1 1-e 0+e 0+e],[0 1 1 1-e 1-e 0+e],c3);plot([0 1 1 0 0],[0 0 1 1 0]);disp('weights');
  "IW{2,1}(234,:)'" : Constant  Value=[0.44414095449370761;-0.90435027038450633;0.60714738222060638;0.036968079542790355;-0.20776735489115694;-0.28783947333693782;0.17425148160904552;0.82218694973617246;-0.39174420291278544;-0.65161128717011096]
      mask Display: e = 0.06;c1 = [120 150 230]/255;c2 = ([120 150 230]+0)/383;c3 = ([120 150 230]+128)/383;patch([0 1 1 0],[0 0 1 1],c1);patch([0 1 1 1-e 1-e 0+e],[0 0 1 1-e 0+e 0+e],c2);patch([0 0 1 1-e 0+e 0+e],[0 1 1 1-e 1-e 0+e],c3);plot([0 1 1 0 0],[0 0 1 1 0]);disp('weights');
  "IW{2,1}(235,:)'" : Constant  Value=[0.36468834648549531;0.74228633275105549;0.3140964078773848;0.060525739551830181;0.43706134820349019;0.71997945648632344;-0.63228083324403539;-0.18189189170358902;-0.29694348474491211;-0.82164112570448466]
      mask Display: e = 0.06;c1 = [120 150 230]/255;c2 = ([120 150 230]+0)/383;c3 = ([120 150 230]+128)/383;patch([0 1 1 0],[0 0 1 1],c1);patch([0 1 1 1-e 1-e 0+e],[0 0 1 1-e 0+e 0+e],c2);patch([0 0 1 1-e 0+e 0+e],[0 1 1 1-e 1-e 0+e],c3);plot([0 1 1 0 0],[0 0 1 1 0]);disp('weights');
  "IW{2,1}(236,:)'" : Constant  Value=[0.35986808374079327;-0.86400071892662045;-0.31177839581600403;0.54487215273154777;-0.36185865908306031;-0.31185751725208688;-0.14042377020497077;0.68140490108584773;0.068773963724546;0.36966892324181044]
      mask Display: e = 0.06;c1 = [120 150 230]/255;c2 = ([120 150 230]+0)/383;c3 = ([120 150 230]+128)/383;patch([0 1 1 0],[0 0 1 1],c1);patch([0 1 1 1-e 1-e 0+e],[0 0 1 1-e 0+e 0+e],c2);patch([0 0 1 1-e 0+e 0+e],[0 1 1 1-e 1-e 0+e],c3);plot([0 1 1 0 0],[0 0 1 1 0]);disp('weights');
  "IW{2,1}(237,:)'" : Constant  Value=[0.39103055345550197;-0.5556142299956055;0.43333103644651905;0.4409150909979711;0.24858232150074305;0.13606620434748415;-0.82903912707487137;0.17249033187502427;-0.78234402916575951;0.089224558442368332]
      mask Display: e = 0.06;c1 = [120 150 230]/255;c2 = ([120 150 230]+0)/383;c3 = ([120 150 230]+128)/383;patch([0 1 1 0],[0 0 1 1],c1);patch([0 1 1 1-e 1-e 0+e],[0 0 1 1-e 0+e 0+e],c2);patch([0 0 1 1-e 0+e 0+e],[0 1 1 1-e 1-e 0+e],c3);plot([0 1 1 0 0],[0 0 1 1 0]);disp('weights');
  "IW{2,1}(238,:)'" : Constant  Value=[0.16801978046946642;-0.089534951282248573;0.19322830742261143;-0.17498369476261438;1.0333716320201038;0.1685013012990032;0.45887888411387656;0.41939546312311304;0.41119422608604045;0.54315721034250652]
      mask Display: e = 0.06;c1 = [120 150 230]/255;c2 = ([120 150 230]+0)/383;c3 = ([120 150 230]+128)/383;patch([0 1 1 0],[0 0 1 1],c1);patch([0 1 1 1-e 1-e 0+e],[0 0 1 1-e 0+e 0+e],c2);patch([0 0 1 1-e 0+e 0+e],[0 1 1 1-e 1-e 0+e],c3);plot([0 1 1 0 0],[0 0 1 1 0]);disp('weights');
  "IW{2,1}(239,:)'" : Constant  Value=[0.035040797004477986;-0.57277758793250566;-0.58322881432493001;-0.23149573241932608;0.069794774950948241;0.208252639026138;0.44986922921635408;-0.27250984001842138;1.1512482624155072;-0.80939140353842176]
      mask Display: e = 0.06;c1 = [120 150 230]/255;c2 = ([120 150 230]+0)/383;c3 = ([120 150 230]+128)/383;patch([0 1 1 0],[0 0 1 1],c1);patch([0 1 1 1-e 1-e 0+e],[0 0 1 1-e 0+e 0+e],c2);patch([0 0 1 1-e 0+e 0+e],[0 1 1 1-e 1-e 0+e],c3);plot([0 1 1 0 0],[0 0 1 1 0]);disp('weights');
  "IW{2,1}(24,:)'" : Constant  Value=[0.21973398681526335;-1.1436823341459299;-0.60628955975317445;-0.53374276066982118;-0.62153722570776515;-0.32626205375088224;0.31220182279086184;0.2314492289281726;0.78476443487015768;-0.22170430986240608]
      mask Display: e = 0.06;c1 = [120 150 230]/255;c2 = ([120 150 230]+0)/383;c3 = ([120 150 230]+128)/383;patch([0 1 1 0],[0 0 1 1],c1);patch([0 1 1 1-e 1-e 0+e],[0 0 1 1-e 0+e 0+e],c2);patch([0 0 1 1-e 0+e 0+e],[0 1 1 1-e 1-e 0+e],c3);plot([0 1 1 0 0],[0 0 1 1 0]);disp('weights');
  "IW{2,1}(240,:)'" : Constant  Value=[-0.96135520764168703;-0.96461248502398378;-0.048294956843569464;0.45009380513302244;-0.8336511940977851;0.55437484812975502;0.21155121670441104;0.15410761252360125;-0.25373790780095601;0.83497552165123246]
      mask Display: e = 0.06;c1 = [120 150 230]/255;c2 = ([120 150 230]+0)/383;c3 = ([120 150 230]+128)/383;patch([0 1 1 0],[0 0 1 1],c1);patch([0 1 1 1-e 1-e 0+e],[0 0 1 1-e 0+e 0+e],c2);patch([0 0 1 1-e 0+e 0+e],[0 1 1 1-e 1-e 0+e],c3);plot([0 1 1 0 0],[0 0 1 1 0]);disp('weights');
  "IW{2,1}(241,:)'" : Constant  Value=[0.13020315923379128;-0.23120502000239179;0.55453273251704471;0.077958439015734377;0.3027348360688546;0.49989626081302935;-0.10476583027884188;-0.33674727752198241;0.44837994226293049;-0.20987889269878474]
      mask Display: e = 0.06;c1 = [120 150 230]/255;c2 = ([120 150 230]+0)/383;c3 = ([120 150 230]+128)/383;patch([0 1 1 0],[0 0 1 1],c1);patch([0 1 1 1-e 1-e 0+e],[0 0 1 1-e 0+e 0+e],c2);patch([0 0 1 1-e 0+e 0+e],[0 1 1 1-e 1-e 0+e],c3);plot([0 1 1 0 0],[0 0 1 1 0]);disp('weights');
  "IW{2,1}(242,:)'" : Constant  Value=[-0.64034031355320131;0.018715088117638987;-0.21406510753490851;-0.74323900598263726;0.30219508445987059;0.85116622370543771;0.056640465771343421;-0.31138102795735711;0.23036730314299148;-0.092773912363107475]
      mask Display: e = 0.06;c1 = [120 150 230]/255;c2 = ([120 150 230]+0)/383;c3 = ([120 150 230]+128)/383;patch([0 1 1 0],[0 0 1 1],c1);patch([0 1 1 1-e 1-e 0+e],[0 0 1 1-e 0+e 0+e],c2);patch([0 0 1 1-e 0+e 0+e],[0 1 1 1-e 1-e 0+e],c3);plot([0 1 1 0 0],[0 0 1 1 0]);disp('weights');
  "IW{2,1}(243,:)'" : Constant  Value=[-0.17274003839115129;0.25672479991418728;-0.48204218375965313;-0.85847740264322336;-0.56302820070197013;-0.033661652343751403;-0.96883627798976901;-0.051921655620075585;-0.3847261897319707;-0.59558409051988559]
      mask Display: e = 0.06;c1 = [120 150 230]/255;c2 = ([120 150 230]+0)/383;c3 = ([120 150 230]+128)/383;patch([0 1 1 0],[0 0 1 1],c1);patch([0 1 1 1-e 1-e 0+e],[0 0 1 1-e 0+e 0+e],c2);patch([0 0 1 1-e 0+e 0+e],[0 1 1 1-e 1-e 0+e],c3);plot([0 1 1 0 0],[0 0 1 1 0]);disp('weights');
  "IW{2,1}(244,:)'" : Constant  Value=[0.085983704804946881;-0.92499714560334811;-0.16666013369503591;0.17547791294163267;0.96824616547753928;0.23871549246269863;-0.13598760587053238;0.13309100026777404;0.13710649267119285;-0.85347795193868392]
      mask Display: e = 0.06;c1 = [120 150 230]/255;c2 = ([120 150 230]+0)/383;c3 = ([120 150 230]+128)/383;patch([0 1 1 0],[0 0 1 1],c1);patch([0 1 1 1-e 1-e 0+e],[0 0 1 1-e 0+e 0+e],c2);patch([0 0 1 1-e 0+e 0+e],[0 1 1 1-e 1-e 0+e],c3);plot([0 1 1 0 0],[0 0 1 1 0]);disp('weights');
  "IW{2,1}(245,:)'" : Constant  Value=[0.21127506244990382;0.064038419119733542;-0.87579334693848732;0.049343590933313614;0.15496292736831468;0.67960107490191135;0.69949044596273746;0.21431553127855105;0.55661760120722215;0.44047651773754193]
      mask Display: e = 0.06;c1 = [120 150 230]/255;c2 = ([120 150 230]+0)/383;c3 = ([120 150 230]+128)/383;patch([0 1 1 0],[0 0 1 1],c1);patch([0 1 1 1-e 1-e 0+e],[0 0 1 1-e 0+e 0+e],c2);patch([0 0 1 1-e 0+e 0+e],[0 1 1 1-e 1-e 0+e],c3);plot([0 1 1 0 0],[0 0 1 1 0]);disp('weights');
  "IW{2,1}(246,:)'" : Constant  Value=[-1.0222252492719335;-1.0120019615506841;0.92422213094976768;-0.0053899573541809995;-0.56781736862000076;0.62983638817888821;-0.039121560552239573;-0.1732256231114698;-0.76434081273625187;-0.35445202428243744]
      mask Display: e = 0.06;c1 = [120 150 230]/255;c2 = ([120 150 230]+0)/383;c3 = ([120 150 230]+128)/383;patch([0 1 1 0],[0 0 1 1],c1);patch([0 1 1 1-e 1-e 0+e],[0 0 1 1-e 0+e 0+e],c2);patch([0 0 1 1-e 0+e 0+e],[0 1 1 1-e 1-e 0+e],c3);plot([0 1 1 0 0],[0 0 1 1 0]);disp('weights');
  "IW{2,1}(247,:)'" : Constant  Value=[-0.050002313837095261;-0.82359164802419071;-0.20439103587839355;0.84492055483131123;-0.26538261370857735;0.37884863489051013;-0.037832447429256719;0.42079644862986015;-0.70053398779746545;0.61050072942272338]
      mask Display: e = 0.06;c1 = [120 150 230]/255;c2 = ([120 150 230]+0)/383;c3 = ([120 150 230]+128)/383;patch([0 1 1 0],[0 0 1 1],c1);patch([0 1 1 1-e 1-e 0+e],[0 0 1 1-e 0+e 0+e],c2);patch([0 0 1 1-e 0+e 0+e],[0 1 1 1-e 1-e 0+e],c3);plot([0 1 1 0 0],[0 0 1 1 0]);disp('weights');
  "IW{2,1}(248,:)'" : Constant  Value=[-0.28794061804902188;-0.096007329839398581;-0.89677145521420998;-1.1445751355787819;0.69501371514359389;0.064397334910957005;0.64169293629906898;0.39577806173883689;0.090204334866688274;-0.57637480701137422]
      mask Display: e = 0.06;c1 = [120 150 230]/255;c2 = ([120 150 230]+0)/383;c3 = ([120 150 230]+128)/383;patch([0 1 1 0],[0 0 1 1],c1);patch([0 1 1 1-e 1-e 0+e],[0 0 1 1-e 0+e 0+e],c2);patch([0 0 1 1-e 0+e 0+e],[0 1 1 1-e 1-e 0+e],c3);plot([0 1 1 0 0],[0 0 1 1 0]);disp('weights');
  "IW{2,1}(249,:)'" : Constant  Value=[0.077534865494603727;-1.1409457164335404;-0.15657793641064155;0.59483714413088373;0.21494459405246355;0.080060226464897299;0.46355034536071105;-0.45916261263394303;0.99206366059174322;-0.22339672517524248]
      mask Display: e = 0.06;c1 = [120 150 230]/255;c2 = ([120 150 230]+0)/383;c3 = ([120 150 230]+128)/383;patch([0 1 1 0],[0 0 1 1],c1);patch([0 1 1 1-e 1-e 0+e],[0 0 1 1-e 0+e 0+e],c2);patch([0 0 1 1-e 0+e 0+e],[0 1 1 1-e 1-e 0+e],c3);plot([0 1 1 0 0],[0 0 1 1 0]);disp('weights');
  "IW{2,1}(25,:)'" : Constant  Value=[0.96457291233423004;-0.46981586331317515;-0.054799386455200882;0.36242952310236098;-0.46327519821427871;0.3713694979941109;0.2312079945846478;0.49056079654419438;-0.20948713440918099;-0.12150259990967367]
      mask Display: e = 0.06;c1 = [120 150 230]/255;c2 = ([120 150 230]+0)/383;c3 = ([120 150 230]+128)/383;patch([0 1 1 0],[0 0 1 1],c1);patch([0 1 1 1-e 1-e 0+e],[0 0 1 1-e 0+e 0+e],c2);patch([0 0 1 1-e 0+e 0+e],[0 1 1 1-e 1-e 0+e],c3);plot([0 1 1 0 0],[0 0 1 1 0]);disp('weights');
  "IW{2,1}(250,:)'" : Constant  Value=[-0.71414911274584869;-0.98524078704592044;0.45395861206062249;0.13722062083066294;0.16500931307790143;0.078335306255862713;-0.065848014408416089;-0.64641257997965018;1.2450665047624918;-0.21900490036239872]
      mask Display: e = 0.06;c1 = [120 150 230]/255;c2 = ([120 150 230]+0)/383;c3 = ([120 150 230]+128)/383;patch([0 1 1 0],[0 0 1 1],c1);patch([0 1 1 1-e 1-e 0+e],[0 0 1 1-e 0+e 0+e],c2);patch([0 0 1 1-e 0+e 0+e],[0 1 1 1-e 1-e 0+e],c3);plot([0 1 1 0 0],[0 0 1 1 0]);disp('weights');
  "IW{2,1}(251,:)'" : Constant  Value=[0.43351641386761963;-0.33723750034179378;-0.61779749748369128;0.055340018684454484;-0.17126909387425493;-0.15626689281550188;0.0096573961509642536;-0.5240492259382602;-0.039855959588991657;-0.23562497199362481]
      mask Display: e = 0.06;c1 = [120 150 230]/255;c2 = ([120 150 230]+0)/383;c3 = ([120 150 230]+128)/383;patch([0 1 1 0],[0 0 1 1],c1);patch([0 1 1 1-e 1-e 0+e],[0 0 1 1-e 0+e 0+e],c2);patch([0 0 1 1-e 0+e 0+e],[0 1 1 1-e 1-e 0+e],c3);plot([0 1 1 0 0],[0 0 1 1 0]);disp('weights');
  "IW{2,1}(252,:)'" : Constant  Value=[0.43696801285456111;-0.33097786117400579;0.5585754143001781;0.47079017325854844;0.26789850086799538;0.54709363695118984;0.046764832653588259;0.38329906443896611;-0.49048765269199424;-0.92783339414391275]
      mask Display: e = 0.06;c1 = [120 150 230]/255;c2 = ([120 150 230]+0)/383;c3 = ([120 150 230]+128)/383;patch([0 1 1 0],[0 0 1 1],c1);patch([0 1 1 1-e 1-e 0+e],[0 0 1 1-e 0+e 0+e],c2);patch([0 0 1 1-e 0+e 0+e],[0 1 1 1-e 1-e 0+e],c3);plot([0 1 1 0 0],[0 0 1 1 0]);disp('weights');
  "IW{2,1}(253,:)'" : Constant  Value=[-0.87276360450199597;-0.67078401305716928;0.25381730527101853;-0.6436126900248319;-0.8342822510671547;-0.19632907363623225;-1.2167330414036244;0.034221623684767583;-0.5304688644811314;0.22440390585362097]
      mask Display: e = 0.06;c1 = [120 150 230]/255;c2 = ([120 150 230]+0)/383;c3 = ([120 150 230]+128)/383;patch([0 1 1 0],[0 0 1 1],c1);patch([0 1 1 1-e 1-e 0+e],[0 0 1 1-e 0+e 0+e],c2);patch([0 0 1 1-e 0+e 0+e],[0 1 1 1-e 1-e 0+e],c3);plot([0 1 1 0 0],[0 0 1 1 0]);disp('weights');
  "IW{2,1}(254,:)'" : Constant  Value=[0.035437120188879151;0.13313126820856125;-0.0085044465338833322;0.38315073091836077;0.15639995330689893;0.85886606689416345;0.039623434244681947;-0.27977182075010387;0.024958278459098527;-0.70901690466982936]
      mask Display: e = 0.06;c1 = [120 150 230]/255;c2 = ([120 150 230]+0)/383;c3 = ([120 150 230]+128)/383;patch([0 1 1 0],[0 0 1 1],c1);patch([0 1 1 1-e 1-e 0+e],[0 0 1 1-e 0+e 0+e],c2);patch([0 0 1 1-e 0+e 0+e],[0 1 1 1-e 1-e 0+e],c3);plot([0 1 1 0 0],[0 0 1 1 0]);disp('weights');
  "IW{2,1}(255,:)'" : Constant  Value=[-0.31933641342173319;0.013534458435914637;-0.83940381025728972;-0.39245646754288849;0.97835608401610852;0.85283146940069599;0.81354460567163778;0.27568195666282536;-0.27497364616679754;0.075585374205106762]
      mask Display: e = 0.06;c1 = [120 150 230]/255;c2 = ([120 150 230]+0)/383;c3 = ([120 150 230]+128)/383;patch([0 1 1 0],[0 0 1 1],c1);patch([0 1 1 1-e 1-e 0+e],[0 0 1 1-e 0+e 0+e],c2);patch([0 0 1 1-e 0+e 0+e],[0 1 1 1-e 1-e 0+e],c3);plot([0 1 1 0 0],[0 0 1 1 0]);disp('weights');
  "IW{2,1}(256,:)'" : Constant  Value=[-0.71164642020576463;-0.041794205547340049;0.90690708645634555;-0.53890406927602086;0.091801758990201279;0.45920088443252238;-0.54755428181455146;-0.41507674580199261;-0.12642034925652534;-0.38844645037797282]
      mask Display: e = 0.06;c1 = [120 150 230]/255;c2 = ([120 150 230]+0)/383;c3 = ([120 150 230]+128)/383;patch([0 1 1 0],[0 0 1 1],c1);patch([0 1 1 1-e 1-e 0+e],[0 0 1 1-e 0+e 0+e],c2);patch([0 0 1 1-e 0+e 0+e],[0 1 1 1-e 1-e 0+e],c3);plot([0 1 1 0 0],[0 0 1 1 0]);disp('weights');
  "IW{2,1}(257,:)'" : Constant  Value=[-0.55241839947577376;-0.0075251768660122634;-0.11511184531383988;-0.47186492737820607;-0.41741899918696673;0.50193811071566952;-0.66146748958301804;-0.30316948858702308;-0.51886266723090257;0.2415124527575756]
      mask Display: e = 0.06;c1 = [120 150 230]/255;c2 = ([120 150 230]+0)/383;c3 = ([120 150 230]+128)/383;patch([0 1 1 0],[0 0 1 1],c1);patch([0 1 1 1-e 1-e 0+e],[0 0 1 1-e 0+e 0+e],c2);patch([0 0 1 1-e 0+e 0+e],[0 1 1 1-e 1-e 0+e],c3);plot([0 1 1 0 0],[0 0 1 1 0]);disp('weights');
  "IW{2,1}(258,:)'" : Constant  Value=[-0.45149571520380527;-1.0264571576040447;-0.35198869787238052;0.65165207576477546;0.97513261858301259;0.15426693497698263;-0.1626117725060465;0.51182322093845134;-0.40500392973113764;0.035203979998439938]
      mask Display: e = 0.06;c1 = [120 150 230]/255;c2 = ([120 150 230]+0)/383;c3 = ([120 150 230]+128)/383;patch([0 1 1 0],[0 0 1 1],c1);patch([0 1 1 1-e 1-e 0+e],[0 0 1 1-e 0+e 0+e],c2);patch([0 0 1 1-e 0+e 0+e],[0 1 1 1-e 1-e 0+e],c3);plot([0 1 1 0 0],[0 0 1 1 0]);disp('weights');
  "IW{2,1}(259,:)'" : Constant  Value=[-0.055741404031106868;-0.7611900048281145;-0.79795247945863634;0.078021828608886484;-0.69062118934335859;0.16008856975917596;-0.19804171050294544;-0.37323828498828276;0.65715797675188226;0.25419644784309764]
      mask Display: e = 0.06;c1 = [120 150 230]/255;c2 = ([120 150 230]+0)/383;c3 = ([120 150 230]+128)/383;patch([0 1 1 0],[0 0 1 1],c1);patch([0 1 1 1-e 1-e 0+e],[0 0 1 1-e 0+e 0+e],c2);patch([0 0 1 1-e 0+e 0+e],[0 1 1 1-e 1-e 0+e],c3);plot([0 1 1 0 0],[0 0 1 1 0]);disp('weights');
  "IW{2,1}(26,:)'" : Constant  Value=[0.25517033073029199;-0.72764229304324191;0.0036127760731148595;0.26587910494925932;0.97153617269845793;0.10920674281997844;0.01832837009559804;0.083871178715840738;0.50805685608161466;-0.29013234047303166]
      mask Display: e = 0.06;c1 = [120 150 230]/255;c2 = ([120 150 230]+0)/383;c3 = ([120 150 230]+128)/383;patch([0 1 1 0],[0 0 1 1],c1);patch([0 1 1 1-e 1-e 0+e],[0 0 1 1-e 0+e 0+e],c2);patch([0 0 1 1-e 0+e 0+e],[0 1 1 1-e 1-e 0+e],c3);plot([0 1 1 0 0],[0 0 1 1 0]);disp('weights');
  "IW{2,1}(260,:)'" : Constant  Value=[0.51345924513578778;0.40938182762108566;-0.051806933548541448;-0.24474659168097246;-0.73284161126097669;0.37393328565167122;0.29774492778742251;-0.27402511068759011;0.47768897980085967;-0.44730884805527427]
      mask Display: e = 0.06;c1 = [120 150 230]/255;c2 = ([120 150 230]+0)/383;c3 = ([120 150 230]+128)/383;patch([0 1 1 0],[0 0 1 1],c1);patch([0 1 1 1-e 1-e 0+e],[0 0 1 1-e 0+e 0+e],c2);patch([0 0 1 1-e 0+e 0+e],[0 1 1 1-e 1-e 0+e],c3);plot([0 1 1 0 0],[0 0 1 1 0]);disp('weights');
  "IW{2,1}(261,:)'" : Constant  Value=[0.63615420663444056;0.23096569666966538;-0.66134824130830661;-0.34457735978190651;0.053401107238947532;0.0054508889529595317;0.39415552838416607;-0.57548101807194418;0.42284379066314332;-0.18598203870298058]
      mask Display: e = 0.06;c1 = [120 150 230]/255;c2 = ([120 150 230]+0)/383;c3 = ([120 150 230]+128)/383;patch([0 1 1 0],[0 0 1 1],c1);patch([0 1 1 1-e 1-e 0+e],[0 0 1 1-e 0+e 0+e],c2);patch([0 0 1 1-e 0+e 0+e],[0 1 1 1-e 1-e 0+e],c3);plot([0 1 1 0 0],[0 0 1 1 0]);disp('weights');
  "IW{2,1}(262,:)'" : Constant  Value=[-0.066094152415709567;0.28795378829601515;-0.68295385268602882;-0.7155760049125901;0.050572307537125577;0.3208895220732112;-0.22704239990883351;-0.33199236856935566;0.16124933061965174;0.73543783039784272]
      mask Display: e = 0.06;c1 = [120 150 230]/255;c2 = ([120 150 230]+0)/383;c3 = ([120 150 230]+128)/383;patch([0 1 1 0],[0 0 1 1],c1);patch([0 1 1 1-e 1-e 0+e],[0 0 1 1-e 0+e 0+e],c2);patch([0 0 1 1-e 0+e 0+e],[0 1 1 1-e 1-e 0+e],c3);plot([0 1 1 0 0],[0 0 1 1 0]);disp('weights');
  "IW{2,1}(263,:)'" : Constant  Value=[0.30895473721967126;-0.6860765962938371;-0.75098313998129262;0.34160379049720757;0.90469315822410867;-0.027473820093956824;0.58283403285429702;0.61846759713802424;-0.17649672455808407;0.43233209125517691]
      mask Display: e = 0.06;c1 = [120 150 230]/255;c2 = ([120 150 230]+0)/383;c3 = ([120 150 230]+128)/383;patch([0 1 1 0],[0 0 1 1],c1);patch([0 1 1 1-e 1-e 0+e],[0 0 1 1-e 0+e 0+e],c2);patch([0 0 1 1-e 0+e 0+e],[0 1 1 1-e 1-e 0+e],c3);plot([0 1 1 0 0],[0 0 1 1 0]);disp('weights');
  "IW{2,1}(264,:)'" : Constant  Value=[-0.075363704777043294;0.46550262564986145;-0.52464229636386872;-0.11042142990911871;0.48821874010194943;0.59855250873934496;-0.40634873990324361;-0.77592638700287575;0.33187726042231325;0.60061476275299153]
      mask Display: e = 0.06;c1 = [120 150 230]/255;c2 = ([120 150 230]+0)/383;c3 = ([120 150 230]+128)/383;patch([0 1 1 0],[0 0 1 1],c1);patch([0 1 1 1-e 1-e 0+e],[0 0 1 1-e 0+e 0+e],c2);patch([0 0 1 1-e 0+e 0+e],[0 1 1 1-e 1-e 0+e],c3);plot([0 1 1 0 0],[0 0 1 1 0]);disp('weights');
  "IW{2,1}(265,:)'" : Constant  Value=[-0.79232237937075967;-0.52101858867642448;-0.18915828622369396;0.40869344875907321;0.11084886169723879;0.63036612862895258;-0.53311053030266542;-0.71213225465382812;0.54846330903036578;0.7457686034380151]
      mask Display: e = 0.06;c1 = [120 150 230]/255;c2 = ([120 150 230]+0)/383;c3 = ([120 150 230]+128)/383;patch([0 1 1 0],[0 0 1 1],c1);patch([0 1 1 1-e 1-e 0+e],[0 0 1 1-e 0+e 0+e],c2);patch([0 0 1 1-e 0+e 0+e],[0 1 1 1-e 1-e 0+e],c3);plot([0 1 1 0 0],[0 0 1 1 0]);disp('weights');
  "IW{2,1}(266,:)'" : Constant  Value=[0.022127317588624379;-0.89456009308553519;-0.16573165822739239;0.81853734313976867;-0.57580523051228605;0.14533346047042722;-0.8282724535501107;-0.028849529912576659;-0.69151629624508082;0.57305971544868539]
      mask Display: e = 0.06;c1 = [120 150 230]/255;c2 = ([120 150 230]+0)/383;c3 = ([120 150 230]+128)/383;patch([0 1 1 0],[0 0 1 1],c1);patch([0 1 1 1-e 1-e 0+e],[0 0 1 1-e 0+e 0+e],c2);patch([0 0 1 1-e 0+e 0+e],[0 1 1 1-e 1-e 0+e],c3);plot([0 1 1 0 0],[0 0 1 1 0]);disp('weights');
  "IW{2,1}(267,:)'" : Constant  Value=[1.1053159593761666;-0.047825088621556877;0.49213973041308307;0.24645413904411562;-0.29027986812619794;-0.28239455792724122;-0.46746273643932423;0.42440127696778385;0.43337734583892107;-1.2412054257603498]
      mask Display: e = 0.06;c1 = [120 150 230]/255;c2 = ([120 150 230]+0)/383;c3 = ([120 150 230]+128)/383;patch([0 1 1 0],[0 0 1 1],c1);patch([0 1 1 1-e 1-e 0+e],[0 0 1 1-e 0+e 0+e],c2);patch([0 0 1 1-e 0+e 0+e],[0 1 1 1-e 1-e 0+e],c3);plot([0 1 1 0 0],[0 0 1 1 0]);disp('weights');
  "IW{2,1}(268,:)'" : Constant  Value=[0.43628185150001442;0.53071156829917343;-0.32823623175178279;0.60538183642473642;-0.10092923391910566;0.89931264475262185;1.0032563144587607;-0.38555236008839339;0.63940185465529875;0.74003381643419974]
      mask Display: e = 0.06;c1 = [120 150 230]/255;c2 = ([120 150 230]+0)/383;c3 = ([120 150 230]+128)/383;patch([0 1 1 0],[0 0 1 1],c1);patch([0 1 1 1-e 1-e 0+e],[0 0 1 1-e 0+e 0+e],c2);patch([0 0 1 1-e 0+e 0+e],[0 1 1 1-e 1-e 0+e],c3);plot([0 1 1 0 0],[0 0 1 1 0]);disp('weights');
  "IW{2,1}(269,:)'" : Constant  Value=[0.69806910904335939;-0.190526182534411;-0.85269364481936327;-0.086905919671124265;0.13808068172602705;-0.34465551179791731;-0.15306702044439272;-0.35034092840566999;-0.033033311827623812;-0.29268682458823797]
      mask Display: e = 0.06;c1 = [120 150 230]/255;c2 = ([120 150 230]+0)/383;c3 = ([120 150 230]+128)/383;patch([0 1 1 0],[0 0 1 1],c1);patch([0 1 1 1-e 1-e 0+e],[0 0 1 1-e 0+e 0+e],c2);patch([0 0 1 1-e 0+e 0+e],[0 1 1 1-e 1-e 0+e],c3);plot([0 1 1 0 0],[0 0 1 1 0]);disp('weights');
  "IW{2,1}(27,:)'" : Constant  Value=[0.89091647481762581;0.52761745117453718;0.54406190183958336;0.43809284691595402;0.4443259227222916;0.85714916716660539;0.14214891816429548;0.095033775413739696;-0.20781387930646197;-0.34084287552715875]
      mask Display: e = 0.06;c1 = [120 150 230]/255;c2 = ([120 150 230]+0)/383;c3 = ([120 150 230]+128)/383;patch([0 1 1 0],[0 0 1 1],c1);patch([0 1 1 1-e 1-e 0+e],[0 0 1 1-e 0+e 0+e],c2);patch([0 0 1 1-e 0+e 0+e],[0 1 1 1-e 1-e 0+e],c3);plot([0 1 1 0 0],[0 0 1 1 0]);disp('weights');
  "IW{2,1}(270,:)'" : Constant  Value=[0.77303027421688131;0.38326046471613145;-0.517325305424577;-0.23915357480561902;1.1702659684621521;-0.013920390887004808;-0.61994161609720833;-1.0496525837689854;0.27077276648403015;-0.11236296679235855]
      mask Display: e = 0.06;c1 = [120 150 230]/255;c2 = ([120 150 230]+0)/383;c3 = ([120 150 230]+128)/383;patch([0 1 1 0],[0 0 1 1],c1);patch([0 1 1 1-e 1-e 0+e],[0 0 1 1-e 0+e 0+e],c2);patch([0 0 1 1-e 0+e 0+e],[0 1 1 1-e 1-e 0+e],c3);plot([0 1 1 0 0],[0 0 1 1 0]);disp('weights');
  "IW{2,1}(271,:)'" : Constant  Value=[-0.5905299022626449;-0.53833523429317387;0.89751494159751077;-0.13862562755413088;1.0537102312756457;0.2304639935117252;-0.52011784209759937;-0.68385014430374158;0.24145063539347641;-0.99663536923540796]
      mask Display: e = 0.06;c1 = [120 150 230]/255;c2 = ([120 150 230]+0)/383;c3 = ([120 150 230]+128)/383;patch([0 1 1 0],[0 0 1 1],c1);patch([0 1 1 1-e 1-e 0+e],[0 0 1 1-e 0+e 0+e],c2);patch([0 0 1 1-e 0+e 0+e],[0 1 1 1-e 1-e 0+e],c3);plot([0 1 1 0 0],[0 0 1 1 0]);disp('weights');
  "IW{2,1}(272,:)'" : Constant  Value=[0.27584809004912159;-0.14502913463608247;0.41798840464894699;0.42732984532013801;-0.11337855568258556;0.18871074328618456;-0.26113127960322791;-0.069592990325535314;0.61757352443106694;0.31532974072100595]
      mask Display: e = 0.06;c1 = [120 150 230]/255;c2 = ([120 150 230]+0)/383;c3 = ([120 150 230]+128)/383;patch([0 1 1 0],[0 0 1 1],c1);patch([0 1 1 1-e 1-e 0+e],[0 0 1 1-e 0+e 0+e],c2);patch([0 0 1 1-e 0+e 0+e],[0 1 1 1-e 1-e 0+e],c3);plot([0 1 1 0 0],[0 0 1 1 0]);disp('weights');
  "IW{2,1}(273,:)'" : Constant  Value=[-0.42158396375474727;-0.24679932869522553;0.87683888492226147;-0.4895069247574545;1.1599085846789841;0.25677310504503748;0.49398999833035684;0.56573755938643955;-0.46812017198782019;0.049838424719162777]
      mask Display: e = 0.06;c1 = [120 150 230]/255;c2 = ([120 150 230]+0)/383;c3 = ([120 150 230]+128)/383;patch([0 1 1 0],[0 0 1 1],c1);patch([0 1 1 1-e 1-e 0+e],[0 0 1 1-e 0+e 0+e],c2);patch([0 0 1 1-e 0+e 0+e],[0 1 1 1-e 1-e 0+e],c3);plot([0 1 1 0 0],[0 0 1 1 0]);disp('weights');
  "IW{2,1}(274,:)'" : Constant  Value=[0.23636923508839383;0.63054708176209295;-0.57441658342908497;-0.20828955543116107;0.16620342575187824;0.78686515771633758;0.065315064097418302;-0.52035631186551501;0.36363755209391907;-0.013411834313057688]
      mask Display: e = 0.06;c1 = [120 150 230]/255;c2 = ([120 150 230]+0)/383;c3 = ([120 150 230]+128)/383;patch([0 1 1 0],[0 0 1 1],c1);patch([0 1 1 1-e 1-e 0+e],[0 0 1 1-e 0+e 0+e],c2);patch([0 0 1 1-e 0+e 0+e],[0 1 1 1-e 1-e 0+e],c3);plot([0 1 1 0 0],[0 0 1 1 0]);disp('weights');
  "IW{2,1}(275,:)'" : Constant  Value=[0.049976064050844662;-0.60152910869347254;0.82626058577215999;0.4858466683419822;0.46652343722820189;-0.022354635227192055;-0.1380544380127868;-0.20622496703540727;0.47053170385119025;0.17617493009757801]
      mask Display: e = 0.06;c1 = [120 150 230]/255;c2 = ([120 150 230]+0)/383;c3 = ([120 150 230]+128)/383;patch([0 1 1 0],[0 0 1 1],c1);patch([0 1 1 1-e 1-e 0+e],[0 0 1 1-e 0+e 0+e],c2);patch([0 0 1 1-e 0+e 0+e],[0 1 1 1-e 1-e 0+e],c3);plot([0 1 1 0 0],[0 0 1 1 0]);disp('weights');
  "IW{2,1}(276,:)'" : Constant  Value=[-0.098333130503617666;-0.062228673718169307;0.088999480854506194;0.41046912451158879;0.78860168265885344;0.72232157354817594;0.43823905417741515;-0.69272761579247277;0.043602268601175026;0.20798449315789011]
      mask Display: e = 0.06;c1 = [120 150 230]/255;c2 = ([120 150 230]+0)/383;c3 = ([120 150 230]+128)/383;patch([0 1 1 0],[0 0 1 1],c1);patch([0 1 1 1-e 1-e 0+e],[0 0 1 1-e 0+e 0+e],c2);patch([0 0 1 1-e 0+e 0+e],[0 1 1 1-e 1-e 0+e],c3);plot([0 1 1 0 0],[0 0 1 1 0]);disp('weights');
  "IW{2,1}(277,:)'" : Constant  Value=[-0.52017439255032449;0.10013394977913695;-0.14963298277165371;-0.296622626701181;0.82439903180489871;0.56578579669822715;-0.38520321288204684;-0.37085001068666107;0.5738090340525801;-0.20107985642635923]
      mask Display: e = 0.06;c1 = [120 150 230]/255;c2 = ([120 150 230]+0)/383;c3 = ([120 150 230]+128)/383;patch([0 1 1 0],[0 0 1 1],c1);patch([0 1 1 1-e 1-e 0+e],[0 0 1 1-e 0+e 0+e],c2);patch([0 0 1 1-e 0+e 0+e],[0 1 1 1-e 1-e 0+e],c3);plot([0 1 1 0 0],[0 0 1 1 0]);disp('weights');
  "IW{2,1}(278,:)'" : Constant  Value=[0.90180897884250322;-0.46700803236009636;0.60358653097003245;0.23592695311990158;0.22712642237754754;-0.026651769629828459;-0.27067045838613468;0.21833429587830921;-0.33560332826965694;-0.60236638097503736]
      mask Display: e = 0.06;c1 = [120 150 230]/255;c2 = ([120 150 230]+0)/383;c3 = ([120 150 230]+128)/383;patch([0 1 1 0],[0 0 1 1],c1);patch([0 1 1 1-e 1-e 0+e],[0 0 1 1-e 0+e 0+e],c2);patch([0 0 1 1-e 0+e 0+e],[0 1 1 1-e 1-e 0+e],c3);plot([0 1 1 0 0],[0 0 1 1 0]);disp('weights');
  "IW{2,1}(279,:)'" : Constant  Value=[-0.20739172804319383;-0.70657598949130507;0.69259282352572815;-0.018221115938342386;-0.73269032412663015;-0.22026497232946785;-0.10586068148005634;-0.48146578207017265;0.52964459435453826;-0.41116651923036807]
      mask Display: e = 0.06;c1 = [120 150 230]/255;c2 = ([120 150 230]+0)/383;c3 = ([120 150 230]+128)/383;patch([0 1 1 0],[0 0 1 1],c1);patch([0 1 1 1-e 1-e 0+e],[0 0 1 1-e 0+e 0+e],c2);patch([0 0 1 1-e 0+e 0+e],[0 1 1 1-e 1-e 0+e],c3);plot([0 1 1 0 0],[0 0 1 1 0]);disp('weights');
  "IW{2,1}(28,:)'" : Constant  Value=[-0.25639164520633223;-1.2771642838347312;-0.051395838019100012;0.49030336357852139;-0.57235428943319788;0.12398868161855148;0.17692639854798661;0.36695964617092147;0.77398428952215292;0.63693021671450434]
      mask Display: e = 0.06;c1 = [120 150 230]/255;c2 = ([120 150 230]+0)/383;c3 = ([120 150 230]+128)/383;patch([0 1 1 0],[0 0 1 1],c1);patch([0 1 1 1-e 1-e 0+e],[0 0 1 1-e 0+e 0+e],c2);patch([0 0 1 1-e 0+e 0+e],[0 1 1 1-e 1-e 0+e],c3);plot([0 1 1 0 0],[0 0 1 1 0]);disp('weights');
  "IW{2,1}(280,:)'" : Constant  Value=[-0.36646136954350345;0.12012876612569849;0.20400217844611152;-0.26847491515466082;-0.33422241632155508;0.62340571265977651;-0.79307763075453352;-0.72554022323474143;0.2030290431705925;-0.056082089373337501]
      mask Display: e = 0.06;c1 = [120 150 230]/255;c2 = ([120 150 230]+0)/383;c3 = ([120 150 230]+128)/383;patch([0 1 1 0],[0 0 1 1],c1);patch([0 1 1 1-e 1-e 0+e],[0 0 1 1-e 0+e 0+e],c2);patch([0 0 1 1-e 0+e 0+e],[0 1 1 1-e 1-e 0+e],c3);plot([0 1 1 0 0],[0 0 1 1 0]);disp('weights');
  "IW{2,1}(281,:)'" : Constant  Value=[0.034042688386363262;-0.11935723878905605;-0.28830714475802388;-0.094370634924616462;-0.11970917645598812;0.47792361440840081;-0.57137927209339268;0.19498841413951451;-0.50731372417849996;0.52833374585420168]
      mask Display: e = 0.06;c1 = [120 150 230]/255;c2 = ([120 150 230]+0)/383;c3 = ([120 150 230]+128)/383;patch([0 1 1 0],[0 0 1 1],c1);patch([0 1 1 1-e 1-e 0+e],[0 0 1 1-e 0+e 0+e],c2);patch([0 0 1 1-e 0+e 0+e],[0 1 1 1-e 1-e 0+e],c3);plot([0 1 1 0 0],[0 0 1 1 0]);disp('weights');
  "IW{2,1}(282,:)'" : Constant  Value=[0.069268479440545178;-0.53114536972110171;-0.1027572480807078;-0.65265155366818228;0.3835962515629649;-0.27600926623411781;-0.74558327629358534;-0.94972035596402171;-0.13512764597712332;0.054189234610065418]
      mask Display: e = 0.06;c1 = [120 150 230]/255;c2 = ([120 150 230]+0)/383;c3 = ([120 150 230]+128)/383;patch([0 1 1 0],[0 0 1 1],c1);patch([0 1 1 1-e 1-e 0+e],[0 0 1 1-e 0+e 0+e],c2);patch([0 0 1 1-e 0+e 0+e],[0 1 1 1-e 1-e 0+e],c3);plot([0 1 1 0 0],[0 0 1 1 0]);disp('weights');
  "IW{2,1}(283,:)'" : Constant  Value=[0.53940368886931278;-0.068004009929767906;-0.99694450225411146;0.014288147587236011;-0.55614361912910759;0.00081556672774407701;0.25921341243379525;0.077845217491232355;-0.47324613887086819;-0.057555267376951935]
      mask Display: e = 0.06;c1 = [120 150 230]/255;c2 = ([120 150 230]+0)/383;c3 = ([120 150 230]+128)/383;patch([0 1 1 0],[0 0 1 1],c1);patch([0 1 1 1-e 1-e 0+e],[0 0 1 1-e 0+e 0+e],c2);patch([0 0 1 1-e 0+e 0+e],[0 1 1 1-e 1-e 0+e],c3);plot([0 1 1 0 0],[0 0 1 1 0]);disp('weights');
  "IW{2,1}(284,:)'" : Constant  Value=[-0.15340268160110279;-0.72138038618671396;-0.83758316225756579;-0.091372024786628009;0.29416246120546602;0.16261635169676769;-0.085985695805651005;0.29595496246130643;-0.50284779622088094;0.12355597101447668]
      mask Display: e = 0.06;c1 = [120 150 230]/255;c2 = ([120 150 230]+0)/383;c3 = ([120 150 230]+128)/383;patch([0 1 1 0],[0 0 1 1],c1);patch([0 1 1 1-e 1-e 0+e],[0 0 1 1-e 0+e 0+e],c2);patch([0 0 1 1-e 0+e 0+e],[0 1 1 1-e 1-e 0+e],c3);plot([0 1 1 0 0],[0 0 1 1 0]);disp('weights');
  "IW{2,1}(285,:)'" : Constant  Value=[0.69297907538577219;-0.053366725487509148;-0.48571763607333818;0.45962636398377471;-0.051651151982411769;0.48841843524038525;-0.0085973057824992871;0.1916221496397286;0.42098661340567967;-0.25484191341722301]
      mask Display: e = 0.06;c1 = [120 150 230]/255;c2 = ([120 150 230]+0)/383;c3 = ([120 150 230]+128)/383;patch([0 1 1 0],[0 0 1 1],c1);patch([0 1 1 1-e 1-e 0+e],[0 0 1 1-e 0+e 0+e],c2);patch([0 0 1 1-e 0+e 0+e],[0 1 1 1-e 1-e 0+e],c3);plot([0 1 1 0 0],[0 0 1 1 0]);disp('weights');
  "IW{2,1}(286,:)'" : Constant  Value=[0.6949124423387969;-0.50682299590648228;-1.0568739704067864;1.1056422396724093;-0.9128470137340966;0.42410644027244004;0.15736231602343026;-0.21305180338133109;0.68492862431875512;0.85816536645060459]
      mask Display: e = 0.06;c1 = [120 150 230]/255;c2 = ([120 150 230]+0)/383;c3 = ([120 150 230]+128)/383;patch([0 1 1 0],[0 0 1 1],c1);patch([0 1 1 1-e 1-e 0+e],[0 0 1 1-e 0+e 0+e],c2);patch([0 0 1 1-e 0+e 0+e],[0 1 1 1-e 1-e 0+e],c3);plot([0 1 1 0 0],[0 0 1 1 0]);disp('weights');
  "IW{2,1}(287,:)'" : Constant  Value=[-0.23822626652771825;-0.13356942912562803;0.73859528228146887;0.21402181922642624;-0.71457067504430016;0.84615744117908709;0.5124264796906709;0.40625243129088129;-0.22443733168763572;0.13629774362316199]
      mask Display: e = 0.06;c1 = [120 150 230]/255;c2 = ([120 150 230]+0)/383;c3 = ([120 150 230]+128)/383;patch([0 1 1 0],[0 0 1 1],c1);patch([0 1 1 1-e 1-e 0+e],[0 0 1 1-e 0+e 0+e],c2);patch([0 0 1 1-e 0+e 0+e],[0 1 1 1-e 1-e 0+e],c3);plot([0 1 1 0 0],[0 0 1 1 0]);disp('weights');
  "IW{2,1}(288,:)'" : Constant  Value=[-0.1680630477286528;-0.63766752351511813;-0.29395707455912901;0.40934747755031803;-0.14117313356378811;0.44077309637378759;-0.033996284274100244;0.20148731258721625;-0.49744478081550919;0.70173767033147871]
      mask Display: e = 0.06;c1 = [120 150 230]/255;c2 = ([120 150 230]+0)/383;c3 = ([120 150 230]+128)/383;patch([0 1 1 0],[0 0 1 1],c1);patch([0 1 1 1-e 1-e 0+e],[0 0 1 1-e 0+e 0+e],c2);patch([0 0 1 1-e 0+e 0+e],[0 1 1 1-e 1-e 0+e],c3);plot([0 1 1 0 0],[0 0 1 1 0]);disp('weights');
  "IW{2,1}(289,:)'" : Constant  Value=[0.5621631257208235;0.16438966582837994;1.1309206731957642;0.18005748703184979;0.07796611744071999;0.60285908165207935;0.84315239855521162;0.28517925316265985;0.021993629616559342;-0.30433465135089466]
      mask Display: e = 0.06;c1 = [120 150 230]/255;c2 = ([120 150 230]+0)/383;c3 = ([120 150 230]+128)/383;patch([0 1 1 0],[0 0 1 1],c1);patch([0 1 1 1-e 1-e 0+e],[0 0 1 1-e 0+e 0+e],c2);patch([0 0 1 1-e 0+e 0+e],[0 1 1 1-e 1-e 0+e],c3);plot([0 1 1 0 0],[0 0 1 1 0]);disp('weights');
  "IW{2,1}(29,:)'" : Constant  Value=[-0.32596470868753968;-0.66435348889860202;0.7404004205813095;-0.44893300695909433;0.62948616017576908;0.36512170697137764;-0.39998307605770278;0.28062248918165072;0.65896099019383048;-0.8565535150243242]
      mask Display: e = 0.06;c1 = [120 150 230]/255;c2 = ([120 150 230]+0)/383;c3 = ([120 150 230]+128)/383;patch([0 1 1 0],[0 0 1 1],c1);patch([0 1 1 1-e 1-e 0+e],[0 0 1 1-e 0+e 0+e],c2);patch([0 0 1 1-e 0+e 0+e],[0 1 1 1-e 1-e 0+e],c3);plot([0 1 1 0 0],[0 0 1 1 0]);disp('weights');
  "IW{2,1}(290,:)'" : Constant  Value=[0.26660057731435777;-0.68977149198395449;-1.1588444792954511;0.78262211272556181;-0.43264752817021751;0.33643990185119999;-0.43306270926095297;-0.76485348587570978;0.47252116873555194;0.90231381706806202]
      mask Display: e = 0.06;c1 = [120 150 230]/255;c2 = ([120 150 230]+0)/383;c3 = ([120 150 230]+128)/383;patch([0 1 1 0],[0 0 1 1],c1);patch([0 1 1 1-e 1-e 0+e],[0 0 1 1-e 0+e 0+e],c2);patch([0 0 1 1-e 0+e 0+e],[0 1 1 1-e 1-e 0+e],c3);plot([0 1 1 0 0],[0 0 1 1 0]);disp('weights');
  "IW{2,1}(291,:)'" : Constant  Value=[0.42707649103298162;0.046815391589819844;-0.30811006210728337;0.059554842243494499;0.95474761432856292;0.15274107420947308;-0.59955154555685053;-0.87918830710211238;0.66614653954152736;-0.81777356008630187]
      mask Display: e = 0.06;c1 = [120 150 230]/255;c2 = ([120 150 230]+0)/383;c3 = ([120 150 230]+128)/383;patch([0 1 1 0],[0 0 1 1],c1);patch([0 1 1 1-e 1-e 0+e],[0 0 1 1-e 0+e 0+e],c2);patch([0 0 1 1-e 0+e 0+e],[0 1 1 1-e 1-e 0+e],c3);plot([0 1 1 0 0],[0 0 1 1 0]);disp('weights');
  "IW{2,1}(292,:)'" : Constant  Value=[0.41844890365366894;-0.064547111187598205;-0.44271416884183346;0.22161206561066149;0.25178161729478221;0.76891171307393968;0.75032458007631608;-0.097829774640593142;0.56918307173242932;-0.74298426233703985]
      mask Display: e = 0.06;c1 = [120 150 230]/255;c2 = ([120 150 230]+0)/383;c3 = ([120 150 230]+128)/383;patch([0 1 1 0],[0 0 1 1],c1);patch([0 1 1 1-e 1-e 0+e],[0 0 1 1-e 0+e 0+e],c2);patch([0 0 1 1-e 0+e 0+e],[0 1 1 1-e 1-e 0+e],c3);plot([0 1 1 0 0],[0 0 1 1 0]);disp('weights');
  "IW{2,1}(293,:)'" : Constant  Value=[-0.39440229644328118;-0.73692298393715638;-0.22757125054279737;-0.33487263359438396;-0.61733967229999609;0.46702251080047275;0.089530154230165221;-0.11103049169042378;0.58337166894941606;-0.65998854316485545]
      mask Display: e = 0.06;c1 = [120 150 230]/255;c2 = ([120 150 230]+0)/383;c3 = ([120 150 230]+128)/383;patch([0 1 1 0],[0 0 1 1],c1);patch([0 1 1 1-e 1-e 0+e],[0 0 1 1-e 0+e 0+e],c2);patch([0 0 1 1-e 0+e 0+e],[0 1 1 1-e 1-e 0+e],c3);plot([0 1 1 0 0],[0 0 1 1 0]);disp('weights');
  "IW{2,1}(294,:)'" : Constant  Value=[-0.82289647199912264;-0.045066423671639599;0.64405425318146281;-0.97078079054218902;-0.80793850903120989;0.61220031269017117;-0.52763387789316252;-0.39375069718407496;-0.4149272223307805;-0.48244369705019963]
      mask Display: e = 0.06;c1 = [120 150 230]/255;c2 = ([120 150 230]+0)/383;c3 = ([120 150 230]+128)/383;patch([0 1 1 0],[0 0 1 1],c1);patch([0 1 1 1-e 1-e 0+e],[0 0 1 1-e 0+e 0+e],c2);patch([0 0 1 1-e 0+e 0+e],[0 1 1 1-e 1-e 0+e],c3);plot([0 1 1 0 0],[0 0 1 1 0]);disp('weights');
  "IW{2,1}(295,:)'" : Constant  Value=[-0.4961136418857347;0.063671848043851481;-0.47778157261599796;-0.78640398355633401;0.69330049406245575;0.12081941925550682;-1.1164818314650584;-0.51910988184472884;-0.69031951611070974;0.36066834925438035]
      mask Display: e = 0.06;c1 = [120 150 230]/255;c2 = ([120 150 230]+0)/383;c3 = ([120 150 230]+128)/383;patch([0 1 1 0],[0 0 1 1],c1);patch([0 1 1 1-e 1-e 0+e],[0 0 1 1-e 0+e 0+e],c2);patch([0 0 1 1-e 0+e 0+e],[0 1 1 1-e 1-e 0+e],c3);plot([0 1 1 0 0],[0 0 1 1 0]);disp('weights');
  "IW{2,1}(296,:)'" : Constant  Value=[0.171759419499527;-0.17220773779407986;-1.1844184891976459;-0.18708170261391155;0.59142675832506275;-0.33493392291807256;-0.7823280996619606;-0.80401586575838013;0.18000321342708159;0.57724150974993693]
      mask Display: e = 0.06;c1 = [120 150 230]/255;c2 = ([120 150 230]+0)/383;c3 = ([120 150 230]+128)/383;patch([0 1 1 0],[0 0 1 1],c1);patch([0 1 1 1-e 1-e 0+e],[0 0 1 1-e 0+e 0+e],c2);patch([0 0 1 1-e 0+e 0+e],[0 1 1 1-e 1-e 0+e],c3);plot([0 1 1 0 0],[0 0 1 1 0]);disp('weights');
  "IW{2,1}(297,:)'" : Constant  Value=[0.40315225441817876;0.3396726087825922;-0.42164515089006027;-0.45109447614832909;-0.41433568131683096;0.5308216058082601;-0.2898698213144319;-0.29095068526981749;-0.54226137878520986;-0.22155782186429251]
      mask Display: e = 0.06;c1 = [120 150 230]/255;c2 = ([120 150 230]+0)/383;c3 = ([120 150 230]+128)/383;patch([0 1 1 0],[0 0 1 1],c1);patch([0 1 1 1-e 1-e 0+e],[0 0 1 1-e 0+e 0+e],c2);patch([0 0 1 1-e 0+e 0+e],[0 1 1 1-e 1-e 0+e],c3);plot([0 1 1 0 0],[0 0 1 1 0]);disp('weights');
  "IW{2,1}(298,:)'" : Constant  Value=[-0.10670275961015194;-0.57305356130538543;0.091826788744195462;0.29162049273844354;-0.80753077698134013;0.2808881339048534;0.13790808252418169;-0.26996659135676399;0.61976202927245883;0.6420095281032635]
      mask Display: e = 0.06;c1 = [120 150 230]/255;c2 = ([120 150 230]+0)/383;c3 = ([120 150 230]+128)/383;patch([0 1 1 0],[0 0 1 1],c1);patch([0 1 1 1-e 1-e 0+e],[0 0 1 1-e 0+e 0+e],c2);patch([0 0 1 1-e 0+e 0+e],[0 1 1 1-e 1-e 0+e],c3);plot([0 1 1 0 0],[0 0 1 1 0]);disp('weights');
  "IW{2,1}(299,:)'" : Constant  Value=[0.2786126973864918;0.19450698519532497;0.99882613307291945;-0.23183266967665084;-0.19933728019123936;0.46098848530454872;-0.47802019193738471;-0.49138775148308989;-0.23036021582617225;-0.60090747852265669]
      mask Display: e = 0.06;c1 = [120 150 230]/255;c2 = ([120 150 230]+0)/383;c3 = ([120 150 230]+128)/383;patch([0 1 1 0],[0 0 1 1],c1);patch([0 1 1 1-e 1-e 0+e],[0 0 1 1-e 0+e 0+e],c2);patch([0 0 1 1-e 0+e 0+e],[0 1 1 1-e 1-e 0+e],c3);plot([0 1 1 0 0],[0 0 1 1 0]);disp('weights');
  "IW{2,1}(3,:)'" : Constant  Value=[-0.47862759350048178;-0.70967421087428217;-0.50077178719477977;-0.55410635955179854;0.21382056601520721;0.19331663149275419;0.13447161312108802;-0.047749864051421009;0.59694474749160009;0.94516070609036384]
      mask Display: e = 0.06;c1 = [120 150 230]/255;c2 = ([120 150 230]+0)/383;c3 = ([120 150 230]+128)/383;patch([0 1 1 0],[0 0 1 1],c1);patch([0 1 1 1-e 1-e 0+e],[0 0 1 1-e 0+e 0+e],c2);patch([0 0 1 1-e 0+e 0+e],[0 1 1 1-e 1-e 0+e],c3);plot([0 1 1 0 0],[0 0 1 1 0]);disp('weights');
  "IW{2,1}(30,:)'" : Constant  Value=[0.34991111729289071;0.090995489129136437;0.3476639715935283;-0.46295723314789627;0.54162849664972179;0.18289764573943601;0.29503361927332861;0.61272933211648228;0.51219445385489226;0.16684531897353061]
      mask Display: e = 0.06;c1 = [120 150 230]/255;c2 = ([120 150 230]+0)/383;c3 = ([120 150 230]+128)/383;patch([0 1 1 0],[0 0 1 1],c1);patch([0 1 1 1-e 1-e 0+e],[0 0 1 1-e 0+e 0+e],c2);patch([0 0 1 1-e 0+e 0+e],[0 1 1 1-e 1-e 0+e],c3);plot([0 1 1 0 0],[0 0 1 1 0]);disp('weights');
  "IW{2,1}(300,:)'" : Constant  Value=[-0.77830433191010395;-1.1507804884055777;0.61433722672040503;-0.51188511238229573;0.022811873811796543;0.46593673251033046;0.72625531164933532;0.38857912708777009;-0.024192468005864554;-0.56777512755228066]
      mask Display: e = 0.06;c1 = [120 150 230]/255;c2 = ([120 150 230]+0)/383;c3 = ([120 150 230]+128)/383;patch([0 1 1 0],[0 0 1 1],c1);patch([0 1 1 1-e 1-e 0+e],[0 0 1 1-e 0+e 0+e],c2);patch([0 0 1 1-e 0+e 0+e],[0 1 1 1-e 1-e 0+e],c3);plot([0 1 1 0 0],[0 0 1 1 0]);disp('weights');
  "IW{2,1}(301,:)'" : Constant  Value=[-0.70804373354334194;-0.042432067508160337;1.1437334664269707;-0.61635450963591265;0.080250629922642092;1.0456985248365305;0.69998877638390944;0.16604074235236574;-0.44362097632206848;-0.45916129081495738]
      mask Display: e = 0.06;c1 = [120 150 230]/255;c2 = ([120 150 230]+0)/383;c3 = ([120 150 230]+128)/383;patch([0 1 1 0],[0 0 1 1],c1);patch([0 1 1 1-e 1-e 0+e],[0 0 1 1-e 0+e 0+e],c2);patch([0 0 1 1-e 0+e 0+e],[0 1 1 1-e 1-e 0+e],c3);plot([0 1 1 0 0],[0 0 1 1 0]);disp('weights');
  "IW{2,1}(302,:)'" : Constant  Value=[0.48423893502143045;0.53238081310829966;0.18801601257782297;0.1869903947090332;1.2247563599513045;0.28175800711734844;0.47377445317541234;-0.033446081159926228;0.95007534790286075;0.16007213825868993]
      mask Display: e = 0.06;c1 = [120 150 230]/255;c2 = ([120 150 230]+0)/383;c3 = ([120 150 230]+128)/383;patch([0 1 1 0],[0 0 1 1],c1);patch([0 1 1 1-e 1-e 0+e],[0 0 1 1-e 0+e 0+e],c2);patch([0 0 1 1-e 0+e 0+e],[0 1 1 1-e 1-e 0+e],c3);plot([0 1 1 0 0],[0 0 1 1 0]);disp('weights');
  "IW{2,1}(303,:)'" : Constant  Value=[-0.74510270947028545;-0.28676454988758859;-0.02412387418865386;0.18474457958032772;1.2745363425693379;0.74941289740187078;-0.074905654508580388;0.27626705720634365;-0.45235862621149803;-0.43804465619162331]
      mask Display: e = 0.06;c1 = [120 150 230]/255;c2 = ([120 150 230]+0)/383;c3 = ([120 150 230]+128)/383;patch([0 1 1 0],[0 0 1 1],c1);patch([0 1 1 1-e 1-e 0+e],[0 0 1 1-e 0+e 0+e],c2);patch([0 0 1 1-e 0+e 0+e],[0 1 1 1-e 1-e 0+e],c3);plot([0 1 1 0 0],[0 0 1 1 0]);disp('weights');
  "IW{2,1}(304,:)'" : Constant  Value=[0.37361975456645413;-0.1908246096568072;-0.58923629334717931;-0.43847913919849496;-0.0049178915558351632;-0.2350433762008739;-0.39780087701869199;-0.26858346362491908;0.46457790946038408;-1.2120974345700257]
      mask Display: e = 0.06;c1 = [120 150 230]/255;c2 = ([120 150 230]+0)/383;c3 = ([120 150 230]+128)/383;patch([0 1 1 0],[0 0 1 1],c1);patch([0 1 1 1-e 1-e 0+e],[0 0 1 1-e 0+e 0+e],c2);patch([0 0 1 1-e 0+e 0+e],[0 1 1 1-e 1-e 0+e],c3);plot([0 1 1 0 0],[0 0 1 1 0]);disp('weights');
  "IW{2,1}(305,:)'" : Constant  Value=[0.70983448469977939;-0.45100803920437144;-0.24349065270734416;0.64422029386583768;-0.20646217608751616;-0.20011508032157543;0.28016417050191311;0.88515513676880331;-0.21916122471764432;0.38473446353339591]
      mask Display: e = 0.06;c1 = [120 150 230]/255;c2 = ([120 150 230]+0)/383;c3 = ([120 150 230]+128)/383;patch([0 1 1 0],[0 0 1 1],c1);patch([0 1 1 1-e 1-e 0+e],[0 0 1 1-e 0+e 0+e],c2);patch([0 0 1 1-e 0+e 0+e],[0 1 1 1-e 1-e 0+e],c3);plot([0 1 1 0 0],[0 0 1 1 0]);disp('weights');
  "IW{2,1}(306,:)'" : Constant  Value=[0.63516174141939674;0.56443480577709049;-0.17120485113766476;0.5346728308195231;1.2903422893149721;0.66868831433965514;0.27800785312036991;0.23488454093047079;-0.0077268133460337424;0.49579869187082232]
      mask Display: e = 0.06;c1 = [120 150 230]/255;c2 = ([120 150 230]+0)/383;c3 = ([120 150 230]+128)/383;patch([0 1 1 0],[0 0 1 1],c1);patch([0 1 1 1-e 1-e 0+e],[0 0 1 1-e 0+e 0+e],c2);patch([0 0 1 1-e 0+e 0+e],[0 1 1 1-e 1-e 0+e],c3);plot([0 1 1 0 0],[0 0 1 1 0]);disp('weights');
  "IW{2,1}(307,:)'" : Constant  Value=[0.073568789113902869;0.055050777607295459;-0.030690563711581936;-0.2325791846103657;0.61459740533806995;0.46605397688937072;0.070717878436853635;0.21138245384459256;-0.10742994787599121;-0.23005494044408858]
      mask Display: e = 0.06;c1 = [120 150 230]/255;c2 = ([120 150 230]+0)/383;c3 = ([120 150 230]+128)/383;patch([0 1 1 0],[0 0 1 1],c1);patch([0 1 1 1-e 1-e 0+e],[0 0 1 1-e 0+e 0+e],c2);patch([0 0 1 1-e 0+e 0+e],[0 1 1 1-e 1-e 0+e],c3);plot([0 1 1 0 0],[0 0 1 1 0]);disp('weights');
  "IW{2,1}(308,:)'" : Constant  Value=[-0.12579061045177517;-0.90047442772612762;0.23607753380849883;0.9392408435513302;1.1238051446667261;0.82795112207195432;0.57897128554353194;0.45132029215927838;0.33075211276722472;-0.32129501236771385]
      mask Display: e = 0.06;c1 = [120 150 230]/255;c2 = ([120 150 230]+0)/383;c3 = ([120 150 230]+128)/383;patch([0 1 1 0],[0 0 1 1],c1);patch([0 1 1 1-e 1-e 0+e],[0 0 1 1-e 0+e 0+e],c2);patch([0 0 1 1-e 0+e 0+e],[0 1 1 1-e 1-e 0+e],c3);plot([0 1 1 0 0],[0 0 1 1 0]);disp('weights');
  "IW{2,1}(309,:)'" : Constant  Value=[0.87099559123892678;-0.038695532307300315;-0.38776787527954976;-0.020201970974874445;0.47594896505930095;-0.42002244787929433;-1.1639630969970161;-0.94086800087573119;-0.35569469387638919;0.23330571893654345]
      mask Display: e = 0.06;c1 = [120 150 230]/255;c2 = ([120 150 230]+0)/383;c3 = ([120 150 230]+128)/383;patch([0 1 1 0],[0 0 1 1],c1);patch([0 1 1 1-e 1-e 0+e],[0 0 1 1-e 0+e 0+e],c2);patch([0 0 1 1-e 0+e 0+e],[0 1 1 1-e 1-e 0+e],c3);plot([0 1 1 0 0],[0 0 1 1 0]);disp('weights');
  "IW{2,1}(31,:)'" : Constant  Value=[0.12335091646177199;-0.31670016193123263;-0.37557117190685174;-1.2105419406405113;1.339184546283009;-0.030408396263917892;-0.017576759222093452;0.5513941121496182;-0.30068136174055965;-0.86132385934585853]
      mask Display: e = 0.06;c1 = [120 150 230]/255;c2 = ([120 150 230]+0)/383;c3 = ([120 150 230]+128)/383;patch([0 1 1 0],[0 0 1 1],c1);patch([0 1 1 1-e 1-e 0+e],[0 0 1 1-e 0+e 0+e],c2);patch([0 0 1 1-e 0+e 0+e],[0 1 1 1-e 1-e 0+e],c3);plot([0 1 1 0 0],[0 0 1 1 0]);disp('weights');
  "IW{2,1}(310,:)'" : Constant  Value=[0.21696687612821625;-0.10730512102956383;1.1762890006565558;-0.36216535593225374;0.70989154668352916;-0.013356758840954663;0.025116484467611611;0.14371485440088377;-0.05166325314641762;-0.76259962793848768]
      mask Display: e = 0.06;c1 = [120 150 230]/255;c2 = ([120 150 230]+0)/383;c3 = ([120 150 230]+128)/383;patch([0 1 1 0],[0 0 1 1],c1);patch([0 1 1 1-e 1-e 0+e],[0 0 1 1-e 0+e 0+e],c2);patch([0 0 1 1-e 0+e 0+e],[0 1 1 1-e 1-e 0+e],c3);plot([0 1 1 0 0],[0 0 1 1 0]);disp('weights');
  "IW{2,1}(311,:)'" : Constant  Value=[0.13996811021351394;-0.46355025227859331;-0.58340897499176947;-0.37744564493163646;-0.16156745404784875;0.20394779271977698;-0.32490063292997889;0.38052612289025622;-0.64597840173200893;0.6695394708117306]
      mask Display: e = 0.06;c1 = [120 150 230]/255;c2 = ([120 150 230]+0)/383;c3 = ([120 150 230]+128)/383;patch([0 1 1 0],[0 0 1 1],c1);patch([0 1 1 1-e 1-e 0+e],[0 0 1 1-e 0+e 0+e],c2);patch([0 0 1 1-e 0+e 0+e],[0 1 1 1-e 1-e 0+e],c3);plot([0 1 1 0 0],[0 0 1 1 0]);disp('weights');
  "IW{2,1}(312,:)'" : Constant  Value=[-0.048824470290672495;-0.08341641547280737;-0.071231329660264811;-0.37019342410355494;-0.99743324177227755;0.32896833474687803;-0.51506601548041497;-0.25307573827941593;-0.31510901172125649;1.2916687613791997]
      mask Display: e = 0.06;c1 = [120 150 230]/255;c2 = ([120 150 230]+0)/383;c3 = ([120 150 230]+128)/383;patch([0 1 1 0],[0 0 1 1],c1);patch([0 1 1 1-e 1-e 0+e],[0 0 1 1-e 0+e 0+e],c2);patch([0 0 1 1-e 0+e 0+e],[0 1 1 1-e 1-e 0+e],c3);plot([0 1 1 0 0],[0 0 1 1 0]);disp('weights');
  "IW{2,1}(313,:)'" : Constant  Value=[0.29412813992509196;0.1543697782436089;1.177770049202669;-0.351135701366454;0.47445500944694874;-0.0041577792105624845;-0.76025564710516202;-0.77551767080043699;0.33746279221143816;-0.78253246468909277]
      mask Display: e = 0.06;c1 = [120 150 230]/255;c2 = ([120 150 230]+0)/383;c3 = ([120 150 230]+128)/383;patch([0 1 1 0],[0 0 1 1],c1);patch([0 1 1 1-e 1-e 0+e],[0 0 1 1-e 0+e 0+e],c2);patch([0 0 1 1-e 0+e 0+e],[0 1 1 1-e 1-e 0+e],c3);plot([0 1 1 0 0],[0 0 1 1 0]);disp('weights');
  "IW{2,1}(314,:)'" : Constant  Value=[1.0613583914899873;0.55305743232366733;-0.43203267400336698;0.7028499621533556;0.73748871340649402;0.33199125700917909;-0.51675744720061745;0.10415278825501778;-0.47817575868613621;-0.11639351007232457]
      mask Display: e = 0.06;c1 = [120 150 230]/255;c2 = ([120 150 230]+0)/383;c3 = ([120 150 230]+128)/383;patch([0 1 1 0],[0 0 1 1],c1);patch([0 1 1 1-e 1-e 0+e],[0 0 1 1-e 0+e 0+e],c2);patch([0 0 1 1-e 0+e 0+e],[0 1 1 1-e 1-e 0+e],c3);plot([0 1 1 0 0],[0 0 1 1 0]);disp('weights');
  "IW{2,1}(315,:)'" : Constant  Value=[0.34758789619206881;0.21231488517434477;0.46094050377056139;-0.2387776347228166;0.40703801357917641;0.36326797836311442;-0.41462034429490457;-0.80422625827599081;0.36816668517206014;0.4621570246555281]
      mask Display: e = 0.06;c1 = [120 150 230]/255;c2 = ([120 150 230]+0)/383;c3 = ([120 150 230]+128)/383;patch([0 1 1 0],[0 0 1 1],c1);patch([0 1 1 1-e 1-e 0+e],[0 0 1 1-e 0+e 0+e],c2);patch([0 0 1 1-e 0+e 0+e],[0 1 1 1-e 1-e 0+e],c3);plot([0 1 1 0 0],[0 0 1 1 0]);disp('weights');
  "IW{2,1}(316,:)'" : Constant  Value=[1.006009789293123;-0.54724174974036954;-0.82720861878953733;0.59022672118178832;-0.93369016110798086;0.002381431537106779;-0.39873768036417423;-0.658389638368159;0.56078712676328579;0.65721611753279907]
      mask Display: e = 0.06;c1 = [120 150 230]/255;c2 = ([120 150 230]+0)/383;c3 = ([120 150 230]+128)/383;patch([0 1 1 0],[0 0 1 1],c1);patch([0 1 1 1-e 1-e 0+e],[0 0 1 1-e 0+e 0+e],c2);patch([0 0 1 1-e 0+e 0+e],[0 1 1 1-e 1-e 0+e],c3);plot([0 1 1 0 0],[0 0 1 1 0]);disp('weights');
  "IW{2,1}(317,:)'" : Constant  Value=[-0.54345797226796166;-0.27956096526644558;0.30366062369764357;-0.64443256576296393;-0.37156222561383223;-0.24716325639069636;-0.31350567381902211;-0.56843191970556139;0.50414799844174973;0.63861226385782599]
      mask Display: e = 0.06;c1 = [120 150 230]/255;c2 = ([120 150 230]+0)/383;c3 = ([120 150 230]+128)/383;patch([0 1 1 0],[0 0 1 1],c1);patch([0 1 1 1-e 1-e 0+e],[0 0 1 1-e 0+e 0+e],c2);patch([0 0 1 1-e 0+e 0+e],[0 1 1 1-e 1-e 0+e],c3);plot([0 1 1 0 0],[0 0 1 1 0]);disp('weights');
  "IW{2,1}(318,:)'" : Constant  Value=[-0.35261700127774348;-0.59450915870632892;0.0013824313162188739;0.22782157356090502;0.82173363758050921;0.063591431346172733;-0.65254036870266985;-0.7465115850431191;0.75551464966942916;-0.73386404112379178]
      mask Display: e = 0.06;c1 = [120 150 230]/255;c2 = ([120 150 230]+0)/383;c3 = ([120 150 230]+128)/383;patch([0 1 1 0],[0 0 1 1],c1);patch([0 1 1 1-e 1-e 0+e],[0 0 1 1-e 0+e 0+e],c2);patch([0 0 1 1-e 0+e 0+e],[0 1 1 1-e 1-e 0+e],c3);plot([0 1 1 0 0],[0 0 1 1 0]);disp('weights');
  "IW{2,1}(319,:)'" : Constant  Value=[1.122722306965459;0.1038079424174887;-0.50405356015587965;-0.24450036420088345;0.22506671624125674;-0.19592349717012947;-0.23540268034711026;-0.067539728660172021;0.38086344140008427;-0.49777194958258197]
      mask Display: e = 0.06;c1 = [120 150 230]/255;c2 = ([120 150 230]+0)/383;c3 = ([120 150 230]+128)/383;patch([0 1 1 0],[0 0 1 1],c1);patch([0 1 1 1-e 1-e 0+e],[0 0 1 1-e 0+e 0+e],c2);patch([0 0 1 1-e 0+e 0+e],[0 1 1 1-e 1-e 0+e],c3);plot([0 1 1 0 0],[0 0 1 1 0]);disp('weights');
  "IW{2,1}(32,:)'" : Constant  Value=[-0.7430632970297858;-0.49034967643088373;0.36367734101764987;0.071349937373047803;-0.71254951702386193;0.65688136119576979;0.13559515351879642;0.62439166829133941;0.32923789131506387;0.20620366912482402]
      mask Display: e = 0.06;c1 = [120 150 230]/255;c2 = ([120 150 230]+0)/383;c3 = ([120 150 230]+128)/383;patch([0 1 1 0],[0 0 1 1],c1);patch([0 1 1 1-e 1-e 0+e],[0 0 1 1-e 0+e 0+e],c2);patch([0 0 1 1-e 0+e 0+e],[0 1 1 1-e 1-e 0+e],c3);plot([0 1 1 0 0],[0 0 1 1 0]);disp('weights');
  "IW{2,1}(320,:)'" : Constant  Value=[-0.69930004488273878;-0.56954752210598458;-0.16159040038358252;-0.54518024639905305;-0.12881428709245707;0.25141602920123862;0.066691848265628004;-0.6085797755852953;1.0512807972146951;-0.11251111574658391]
      mask Display: e = 0.06;c1 = [120 150 230]/255;c2 = ([120 150 230]+0)/383;c3 = ([120 150 230]+128)/383;patch([0 1 1 0],[0 0 1 1],c1);patch([0 1 1 1-e 1-e 0+e],[0 0 1 1-e 0+e 0+e],c2);patch([0 0 1 1-e 0+e 0+e],[0 1 1 1-e 1-e 0+e],c3);plot([0 1 1 0 0],[0 0 1 1 0]);disp('weights');
  "IW{2,1}(321,:)'" : Constant  Value=[-0.49643142796296624;-1.4616901511299576;-0.27768128649933888;0.19677648202963371;-0.55898577591259813;0.1785648700439762;-0.83618391480355447;-0.2729119388940397;-0.68091046637563635;-0.40593138641520743]
      mask Display: e = 0.06;c1 = [120 150 230]/255;c2 = ([120 150 230]+0)/383;c3 = ([120 150 230]+128)/383;patch([0 1 1 0],[0 0 1 1],c1);patch([0 1 1 1-e 1-e 0+e],[0 0 1 1-e 0+e 0+e],c2);patch([0 0 1 1-e 0+e 0+e],[0 1 1 1-e 1-e 0+e],c3);plot([0 1 1 0 0],[0 0 1 1 0]);disp('weights');
  "IW{2,1}(322,:)'" : Constant  Value=[0.44847424263735042;-0.45023654385657175;-0.48022626959255282;0.56500911814189048;-0.71001723852244314;0.56888038800921936;0.63318630253089891;0.1096178110909039;-0.26540135469742787;0.037462345480080525]
      mask Display: e = 0.06;c1 = [120 150 230]/255;c2 = ([120 150 230]+0)/383;c3 = ([120 150 230]+128)/383;patch([0 1 1 0],[0 0 1 1],c1);patch([0 1 1 1-e 1-e 0+e],[0 0 1 1-e 0+e 0+e],c2);patch([0 0 1 1-e 0+e 0+e],[0 1 1 1-e 1-e 0+e],c3);plot([0 1 1 0 0],[0 0 1 1 0]);disp('weights');
  "IW{2,1}(323,:)'" : Constant  Value=[-0.055730312978417476;-0.29572747327568855;-0.54628080229300868;-0.6527964977273133;1.1773128360933929;-0.30587799472088029;-1.061829748065322;-1.2010103874443681;0.7104201910442034;0.41692068076333899]
      mask Display: e = 0.06;c1 = [120 150 230]/255;c2 = ([120 150 230]+0)/383;c3 = ([120 150 230]+128)/383;patch([0 1 1 0],[0 0 1 1],c1);patch([0 1 1 1-e 1-e 0+e],[0 0 1 1-e 0+e 0+e],c2);patch([0 0 1 1-e 0+e 0+e],[0 1 1 1-e 1-e 0+e],c3);plot([0 1 1 0 0],[0 0 1 1 0]);disp('weights');
  "IW{2,1}(324,:)'" : Constant  Value=[-0.13952573137828173;0.2861962180244102;-0.22586376759557575;-0.7619248400506754;-0.12864443028139294;0.6111329069234418;-0.23834977273870156;0.079031814941679573;0.2027880365323001;-0.43024454384810346]
      mask Display: e = 0.06;c1 = [120 150 230]/255;c2 = ([120 150 230]+0)/383;c3 = ([120 150 230]+128)/383;patch([0 1 1 0],[0 0 1 1],c1);patch([0 1 1 1-e 1-e 0+e],[0 0 1 1-e 0+e 0+e],c2);patch([0 0 1 1-e 0+e 0+e],[0 1 1 1-e 1-e 0+e],c3);plot([0 1 1 0 0],[0 0 1 1 0]);disp('weights');
  "IW{2,1}(325,:)'" : Constant  Value=[0.31908859795658534;-0.61043410871654169;0.05016131330849638;0.30763032669766621;-0.72148650876861464;0.4673538732505374;-0.17064849725924902;-0.22624774790614327;0.75554316451654424;0.71834699928849388]
      mask Display: e = 0.06;c1 = [120 150 230]/255;c2 = ([120 150 230]+0)/383;c3 = ([120 150 230]+128)/383;patch([0 1 1 0],[0 0 1 1],c1);patch([0 1 1 1-e 1-e 0+e],[0 0 1 1-e 0+e 0+e],c2);patch([0 0 1 1-e 0+e 0+e],[0 1 1 1-e 1-e 0+e],c3);plot([0 1 1 0 0],[0 0 1 1 0]);disp('weights');
  "IW{2,1}(326,:)'" : Constant  Value=[0.77706510962289577;0.58547673151451052;0.37731524314877002;-0.21011635002256601;0.54813076455427723;0.46355374046979991;0.14567275539253027;0.93174444620739472;0.43288683367553188;-0.16146303162768466]
      mask Display: e = 0.06;c1 = [120 150 230]/255;c2 = ([120 150 230]+0)/383;c3 = ([120 150 230]+128)/383;patch([0 1 1 0],[0 0 1 1],c1);patch([0 1 1 1-e 1-e 0+e],[0 0 1 1-e 0+e 0+e],c2);patch([0 0 1 1-e 0+e 0+e],[0 1 1 1-e 1-e 0+e],c3);plot([0 1 1 0 0],[0 0 1 1 0]);disp('weights');
  "IW{2,1}(327,:)'" : Constant  Value=[0.67139645615808163;0.40532696710437655;-0.40029954787821831;-0.6297001108685224;-0.64964966763127063;0.038807241391143055;-0.089067989921991136;0.19659084913407499;0.58510446238986824;0.44963216795664002]
      mask Display: e = 0.06;c1 = [120 150 230]/255;c2 = ([120 150 230]+0)/383;c3 = ([120 150 230]+128)/383;patch([0 1 1 0],[0 0 1 1],c1);patch([0 1 1 1-e 1-e 0+e],[0 0 1 1-e 0+e 0+e],c2);patch([0 0 1 1-e 0+e 0+e],[0 1 1 1-e 1-e 0+e],c3);plot([0 1 1 0 0],[0 0 1 1 0]);disp('weights');
  "IW{2,1}(328,:)'" : Constant  Value=[0.64199323658992036;-0.60680228057949392;-0.31969074997710106;-0.024107298858842052;0.54757132362903327;-0.14416869250122977;0.14067028802796061;0.68672191100550961;0.13567127154907188;-0.30083156242317521]
      mask Display: e = 0.06;c1 = [120 150 230]/255;c2 = ([120 150 230]+0)/383;c3 = ([120 150 230]+128)/383;patch([0 1 1 0],[0 0 1 1],c1);patch([0 1 1 1-e 1-e 0+e],[0 0 1 1-e 0+e 0+e],c2);patch([0 0 1 1-e 0+e 0+e],[0 1 1 1-e 1-e 0+e],c3);plot([0 1 1 0 0],[0 0 1 1 0]);disp('weights');
  "IW{2,1}(329,:)'" : Constant  Value=[0.23069430239086991;-0.90436865324907312;1.0332866671405874;0.22140779239732522;0.069210296059599219;-0.18017883762606512;-0.78866030869970261;-0.19726008109115561;0.18881626917117564;-0.28916341126049933]
      mask Display: e = 0.06;c1 = [120 150 230]/255;c2 = ([120 150 230]+0)/383;c3 = ([120 150 230]+128)/383;patch([0 1 1 0],[0 0 1 1],c1);patch([0 1 1 1-e 1-e 0+e],[0 0 1 1-e 0+e 0+e],c2);patch([0 0 1 1-e 0+e 0+e],[0 1 1 1-e 1-e 0+e],c3);plot([0 1 1 0 0],[0 0 1 1 0]);disp('weights');
  "IW{2,1}(33,:)'" : Constant  Value=[-0.082728383405184153;-0.56161602565159774;-0.4216123457238749;0.13642462335134192;0.5804209405311378;0.55995729014865481;-0.59738386148164457;-0.30214406903160657;0.54669092837126343;0.083262516579054063]
      mask Display: e = 0.06;c1 = [120 150 230]/255;c2 = ([120 150 230]+0)/383;c3 = ([120 150 230]+128)/383;patch([0 1 1 0],[0 0 1 1],c1);patch([0 1 1 1-e 1-e 0+e],[0 0 1 1-e 0+e 0+e],c2);patch([0 0 1 1-e 0+e 0+e],[0 1 1 1-e 1-e 0+e],c3);plot([0 1 1 0 0],[0 0 1 1 0]);disp('weights');
  "IW{2,1}(330,:)'" : Constant  Value=[-0.16432343426246093;-0.3864455659802904;-0.46025413596621456;0.018100162381909507;0.76684006871705868;0.61307594709207747;0.59325697621202678;-0.30218438980768758;0.68081854237686978;-0.064237321429635896]
      mask Display: e = 0.06;c1 = [120 150 230]/255;c2 = ([120 150 230]+0)/383;c3 = ([120 150 230]+128)/383;patch([0 1 1 0],[0 0 1 1],c1);patch([0 1 1 1-e 1-e 0+e],[0 0 1 1-e 0+e 0+e],c2);patch([0 0 1 1-e 0+e 0+e],[0 1 1 1-e 1-e 0+e],c3);plot([0 1 1 0 0],[0 0 1 1 0]);disp('weights');
  "IW{2,1}(331,:)'" : Constant  Value=[0.25392740292927674;-0.26995976961691326;-0.97776037902584456;-0.16141691117796647;-0.58934882956631229;0.084905900585637295;-0.69243630605429152;-0.48231311281406553;0.27527737330251012;0.096213236763111221]
      mask Display: e = 0.06;c1 = [120 150 230]/255;c2 = ([120 150 230]+0)/383;c3 = ([120 150 230]+128)/383;patch([0 1 1 0],[0 0 1 1],c1);patch([0 1 1 1-e 1-e 0+e],[0 0 1 1-e 0+e 0+e],c2);patch([0 0 1 1-e 0+e 0+e],[0 1 1 1-e 1-e 0+e],c3);plot([0 1 1 0 0],[0 0 1 1 0]);disp('weights');
  "IW{2,1}(332,:)'" : Constant  Value=[0.13055348753019477;-0.18991541306371224;0.036347621006446451;0.27529654811568133;0.093075538069129798;0.44032264410566668;-0.26970187559444908;-0.53396036911802414;0.23216066007011213;-0.1862401372592136]
      mask Display: e = 0.06;c1 = [120 150 230]/255;c2 = ([120 150 230]+0)/383;c3 = ([120 150 230]+128)/383;patch([0 1 1 0],[0 0 1 1],c1);patch([0 1 1 1-e 1-e 0+e],[0 0 1 1-e 0+e 0+e],c2);patch([0 0 1 1-e 0+e 0+e],[0 1 1 1-e 1-e 0+e],c3);plot([0 1 1 0 0],[0 0 1 1 0]);disp('weights');
  "IW{2,1}(333,:)'" : Constant  Value=[-0.29141356976015953;0.58435732068376467;0.18514174997415245;-0.74911963282248661;0.56235575083275546;0.30190835928805271;-1.1310181107720441;-0.37186628848757813;0.63364461972424102;-0.17115328264515695]
      mask Display: e = 0.06;c1 = [120 150 230]/255;c2 = ([120 150 230]+0)/383;c3 = ([120 150 230]+128)/383;patch([0 1 1 0],[0 0 1 1],c1);patch([0 1 1 1-e 1-e 0+e],[0 0 1 1-e 0+e 0+e],c2);patch([0 0 1 1-e 0+e 0+e],[0 1 1 1-e 1-e 0+e],c3);plot([0 1 1 0 0],[0 0 1 1 0]);disp('weights');
  "IW{2,1}(334,:)'" : Constant  Value=[0.92908752142179662;0.23710452704389184;0.077403100697553712;0.22548976270001478;-0.64691164021081826;0.60574150052473796;0.45117058860659409;0.95339572496479885;-0.47550245343141118;-0.27344151241587505]
      mask Display: e = 0.06;c1 = [120 150 230]/255;c2 = ([120 150 230]+0)/383;c3 = ([120 150 230]+128)/383;patch([0 1 1 0],[0 0 1 1],c1);patch([0 1 1 1-e 1-e 0+e],[0 0 1 1-e 0+e 0+e],c2);patch([0 0 1 1-e 0+e 0+e],[0 1 1 1-e 1-e 0+e],c3);plot([0 1 1 0 0],[0 0 1 1 0]);disp('weights');
  "IW{2,1}(335,:)'" : Constant  Value=[0.77160976061130926;0.29564943257462523;-0.10247541811609005;-0.36111738922289932;0.27529955321140998;0.19004801491644774;-0.74537392004888259;0.41837107359037723;-0.36624935570435802;-0.98709107872709212]
